simulink library "vehdynlibtire"  (R2019b)
settings: Solver=ode45  StartTime=0.0  StopTime=10.0  RelTol=1e-3  EnableMultiTasking=on
libraries: vehdynlibtirecommon x6, autolibshared x4, autolibsharedcommon x1
(part 1 of 3)
Description:
  | Vehicle Dynamics Blockset Library: Tire Dynamics
settings Model: ModifiedByFormat=The MathWorks, Inc.  Creator=The MathWorks, Inc.  LastModifiedBy=The MathWorks, Inc.
settings DataIOCC: LimitDataPoints=on  SaveFormat=Array  ReturnWorkspaceOutputs=off
settings OptimizationCC: LifeSpan=inf
settings DebuggingCC: AllowSymbolicDim=off  PregeneratedLibrarySubsystemCodeDiagnostic=none  SFUnexpectedBacktrackingDiag=warning  SFNoUnconditionalDefaultTransitionDiag=warning  SFExecutionAtInitializationDiag=none  ArithmeticOperatorsInVariantConditions=warning
settings HardwareCC: ProdBitPerPointer=32  ProdBitPerSizeT=32  ProdBitPerPtrDiffT=32  ProdLargestAtomicFloat=None  ProdIntDivRoundTo=Undefined  ProdEndianess=Unspecified  ProdWordSize=32  ProdHWDeviceType=32-bit Generic
settings ModelReferenceCC: PropagateSignalLabelsOutOfModel=off
settings SFSimCC: SimUseLocalCustomCode=off  CustomCodeUndefinedFunction=UseInterfaceOnly
settings RTWCC: RTWUseLocalCustomCode=off
settings CodeAppCC: StateflowObjectComments=on
settings GRTTargetCC: TargetLangStandard=C89/C90 (ANSI)  GeneratePreprocessorConditionals=Disable all
settings ConfigComp: CovMetricSettings=dw  CovHtmlReporting=on  CovSaveCumulativeToWorkspaceVar=on  CovSaveSingleToWorkspaceVar=on  CovShowResultsExplorer=off  CovExternalEMLEnable=off

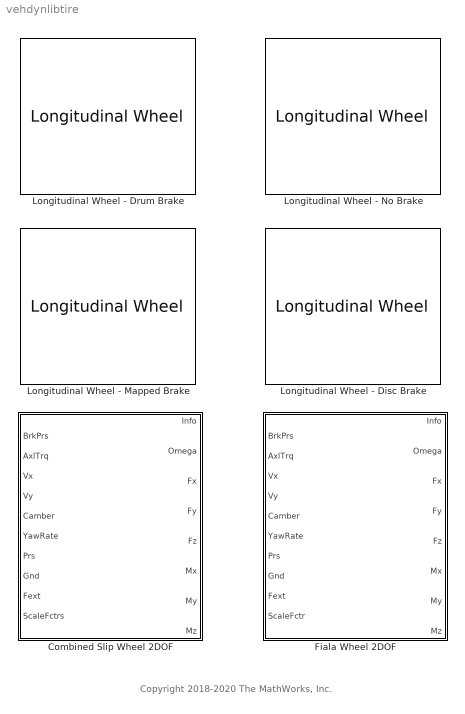
== system vehdynlibtire ==
  note: Copyright 2018-2020 The MathWorks, Inc.
  Combined Slip Wheel 2DOF : Subsystem  mask(Combined Slip Wheel 2DOF){BrakeType=Disc, mu_static=.3, mu_kinetic=.2, disk_abore=.05, Rm=.177, num_pads=2, drum_abore=0.0508, drum_a=0.123, drum_c=0.212, drum_r=0.15, drum_theta1=0, drum_theta2=126, brake_p_bpt=[1 11.4736842105263 21.9473684210526 32.4210526315789 42.8947368421053 53.3684210526316 63.8421052631579 74.3157894736842 84.7894736842105 95.2631578947368 105.736842105263 116.210526315789 126.684210526316 137.157894736842 147.631578947368 158.105263157895 168.578947368421 179.052631578947 189.526315789474 200], brake_n_bpt=[0 52.6315789473684 105.263157894737 157.894736842105 210.526315789474 263.157894736842 315.789473684211 368.421052631579 421.052631578947 473.684210526316 526.315789473684 578.947368421053 631.578947368421 684.210526315789 736.842105263158 789.473684210526 842.105263157895 894.736842105263 947.368421052632 1000], f_brake_t=[43.4900602404453 42.5056030554862 41.5350898940194 40.5780454442085 39.6340111501808 38.7025443887544 37.7832176914519 36.8756180088306 35.9793460143796 35.0940154454303 34.2192524787115 33.3546951383474 32.4999927342521 31.6548053290159 30.8188032315107 29.991666515561 29.1730845621415 28.362755623661 27.5603864089927 26.765691687993;498.991217495636 487.695866636631 476.560505099801 465.579679307235 454.748127933653 444.060772460445 433.51270824929 423.099196101319 412.81565427025 402.657650900201 392.620896861006 382.701238955775 372.894653477208 363.197240090814 353.605216024701 344.114910546964 334.722759712992 325.425301366216 316.219170376863 307.10109410434;954.492374750826 932.886130217776 911.585920305583 890.581313170261 869.862244717126 849.419000532136 829.242198807128 809.322774193808 789.651962526121 770.221286354971 751.0225412433 732.047782773203 713.289314220164 694.739674852612 676.391628817892 658.238154578366 640.272434863842 622.48784710877 604.877954344734 587.436496520688;1409.99353200602 1378.07639379892 1346.61133551136 1315.58294703329 1284.9763615006 1254.77722860383 1224.97168936497 1195.5463522863 1166.48827078199 1137.78492180974 1109.42418562559 1081.39432659063 1053.68397496312 1026.28210961441 999.178041611083 972.361398609768 945.822110014692 919.550392851325 893.536738312604 867.771898937035;1865.49468926121 1823.26665738007 1781.63675071715 1740.58458089631 1700.09047828407 1660.13545667552 1620.7011799228 1581.76993037878 1543.32457903786 1505.34855726451 1467.82583000789 1430.74087040806 1394.07863570608 1357.82454437621 1321.96445440427 1286.48464264117 1251.37178516554 1216.61293859388 1182.19552228048 1148.10730135338;2320.9958465164 2268.45692096121 2216.66216592293 2165.58621475934 2115.20459506754 2065.49368474721 2016.43067048064 1967.99350847127 1920.16088729373 1872.91219271928 1826.22747439018 1780.08741422549 1734.47329644903 1689.36697913801 1644.75086719747 1600.60788667257 1556.92146031639 1513.67548433643 1470.85430624835 1428.44270376973;2776.49700377159 2713.64718454235 2651.68758112871 2590.58784862237 2530.31871185102 2470.8519128189 2412.16016103848 2354.21708656376 2296.9971955496 2240.47582817405 2184.62911877248 2129.43395804292 2074.86795719199 2020.9094138998 1967.53727999066 1914.73113070398 1862.47113546724 1810.73803007899 1759.51309021622 1708.77810618608;3231.99816102678 3158.8374481235 3086.71299633449 3015.58948248539 2945.43282863449 2876.21014089059 2807.88965159632 2740.44066465625 2673.83350380547 2608.03946362882 2543.03076315477 2478.78050186034 2415.26261793494 2352.4518486616 2290.32369278385 2228.85437473538 2168.02081061809 2107.80057582154 2048.17187418409 1989.11350860242;3687.49931828197 3604.02771170464 3521.73841154027 3440.59111634842 3360.54694541796 3281.56836896228 3203.61914215416 3126.66424274874 3050.66981206134 2975.60309908359 2901.43240753707 2828.12704567777 2755.6572786779 2683.9942834234 2613.11010557704 2542.97761876678 2473.57048576894 2404.8631215641 2336.83065815196 2269.44891101877;4143.00047553716 4049.21797528579 3956.76382674606 3865.59275021144 3775.66106220143 3686.92659703397 3599.34863271199 3512.88782084123 3427.50612031721 3343.16673453836 3259.83405191936 3177.4735894952 3096.05193942085 3015.5367181852 2935.89651837023 2857.10086279818 2779.12016091979 2701.92566730665 2625.48944211983 2549.78431343512;4598.50163279235 4494.40823886693 4391.78924195184 4290.59438407447 4190.77517898491 4092.28482510566 3995.07812326983 3899.11139893372 3804.34242857308 3710.73036999313 3618.23569630166 3526.82013331263 3436.44660016381 3347.079152947 3258.68293116342 3171.22410682959 3084.66983607064 2998.98821304921 2914.1482260877 2830.11971585147;5054.00279004754 4939.59850244808 4826.81465715762 4715.59601793749 4605.88929576838 4497.64305317735 4390.80761382767 4285.3349770262 4181.17873682896 4078.2940054479 3976.63734068395 3876.16667713006 3776.84126090677 3678.62158770879 3581.46934395661 3485.34735086099 ...(+2764 chars)], tireParamSet=vdynPassCar.mat, plySteer=off, turnslip=off, PRESMAX=1003118, PRESMIN=9982, FZMAX=10000, FZMIN=100, VXLOW=0.1, KPUMAX=1.5, KPUMIN=-1.5, ALPMAX=1.5708, ALPMIN=-1.5708, CAMMAX=0.173142086627737, CAMMIN=-0.173348165334087, LONGVL=16.7, omegao=0, br=1e-3, UNLOADED_RADIUS=0.309, NOMPRES=224006, FNOMIN=4025, WIDTH=0.209, MASS=9.465, IYY=0.7406, GRAVITY=-9.81, zo=0, zdoto=0, BREFF=8.25094594147963, DREFF=0.260468730454265, FREFF=0.0735298544471851, Q_RE0=1.00866439868088, Q_V1=0.000760413786224011, Q_V2=0.0463384792019201, Q_FZ1=0, Q_FZ2=15.6870832810226, Q_FZ3=0, Q_FCX=0.138643970247602, Q_FCY=0.10843499565426, Q_FCY2=-0.465763352339538, PFZ1=0.69958166705601, VERTICAL_STIFFNESS=207885.061134007, VERTICAL_DAMPING=494.649255786991, LONGITUDINAL_STIFFNESS=388714.175879854, LATERAL_STIFFNESS=157087.404633332, PCFX1=0.18539229191199, PCFX2=0, PCFX3=0, PCFY1=0.163183345037677, PCFY2=0, PCFY3=0.249094918231954, Q_RA1=0.675942571700787, Q_RA2=0.73800463546164, Q_RB1=1.04487486456705, Q_RB2=-1.191763806629, PCX1=1.58523057950359, PDX1=1.0239116238178, PDX2=-0.0842405110022724, PDX3=0, PEX1=0.110312777158455, PEX2=0.313468516038146, PEX3=0, PEX4=0.0016060905760045, PKX1=21.3872544684023, PKX2=14.0006541873175, PKX3=-0.405326109653452, PHX1=0.000212599305364818, PHX2=0.00115950515263055, PVX1=1.59236164471432e-05, PVX2=0.000104321112127671, PPX1=-0.349461321276586, PPX2=0.387840040616429, PPX3=-0.0969947336569324, PPX4=0.0632271859795801, RBX1=12.7633329850276, RBX2=9.5787123658471, RBX3=0, RCX1=1.02796280922059, REX1=-0.45202516851367, REX2=-0.47304886171176, RHX1=0.000233272373115809, QSX1=-0.00788307788961443, QSX2=0.954629515459396, QSX3=0.0155855777667025, QSX4=0.125904607142414, QSX5=1.01110069703963, QSX6=20.1938577118433, QSX7=0.310818120717083, QSX8=-0.0430823751139655, QSX9=0.636494404888216, QSX10=0.142438060591663, QSX11=0.346766530036373, QSX12=0, QSX13=0, QSX14=0, PPMX1=0, PCY1=1.34299950037631, PDY1=0.878267729082195, PDY2=-0.0644597923147385, PDY3=0, PEY1=-0.809776534470972, PEY2=-0.600180598867198, PEY3=0.0991732552633487, PEY4=-6.5577974035573, PEY5=0, PKY1=-15.5714726518315, PKY2=1.73126522291751, PKY3=0.365349873517229, PKY4=1.98176755955416, PKY5=0, PKY6=-0.884005199550313, PKY7=-0.237259727611847, PHY1=-0.00183370557235628, PHY2=0.00346401302716671, PVY1=-0.00675427560163264, PVY2=0.036379218103843, PVY3=-0.163543984089166, PVY4=-0.491003349625726, PPY1=-0.62059646553185, PPY2=-0.0647824842338686, PPY3=-0.164648843290686, PPY4=0.283193909060098, PPY5=0, RBY1=10.7588809173639, RBY2=7.70420065295029, RBY3=3.40283755070691e-06, RBY4=0, RCY1=1.06691874059059, REY1=0.308244924574305, REY2=7.48775032604508e-06, RHY1=0.0118479204960415, RHY2=7.63650177161071e-06, RVY1=0.0560024425050078, RVY2=7.48487127056197e-06, RVY3=0, RVY4=98.4047026517149, RVY5=2.02759273900054, RVY6=15.7623064923347, QSY1=0.00699077564863536, QSY2=0, QSY3=0.00153535478298811, QSY4=8.55710322455322e-05, QSY5=0, QSY6=0, QSY7=0.89443879773793, QSY8=-0.403227641260894, QBZ1=11.666656027484, QBZ2=-1.30355438574485, QBZ3=0, QBZ4=0.177918305399071, QBZ5=-0.162481135068033, QBZ6=0, QBZ9=30.1445534682089, QBZ10=0, QCZ1=1.29026978207574, QDZ1=0.0886972644991399, QDZ2=-0.0058634820161856, QDZ3=0.3805597481383, QDZ4=0, QDZ6=0.00160914918118959, QDZ7=-0.00211036330862154, QDZ8=-0.13921904912557, QDZ9=0.00816585550028243, QDZ10=0, QDZ11=0, QEZ1=-2.19802254534746, QEZ2=1.01850535789165, QEZ3=0, QEZ4=0.278379679112054, QEZ5=-0.548414722765386, QHZ1=0.00148361198869669, QHZ2=0.00202017567585904, QHZ3=0.240316641332066, QHZ4=-0.210114035738085, PPZ1=-0.443927982388615, PPZ2=0, SSZ1=0.00914999585397887, SSZ2=0.0389830656052735, SSZ3=0, SSZ4=0, PDXP1=0.396718274678791, PDXP2=0, PDXP3=0, PKYP1=1.00587060633573, PDYP1=0.40483048923438, PDYP2=0, PDYP3=0, PDYP4=0, PHYP1=0.992731942067188, PHYP2=0.150352945499914, PHYP3=0, PHYP4=-3.98988682633674, PECP1=0.502379254513503, PECP2=0, QDTP1=10.0178654287947, QCRP1=0.200627747200702, QCRP2=0.0995735881599772, QBRP1=0.0997107127960717, QDRP1=1.01432910167423, QDRP2=0, aMode=2}
      mask prompts: BrakeType "vdynblks:vehdynLatTire:blkPrm_BrakeType"; mu_static "autoblks_shared:autoblkLongitudinalWheel:blkPrm_mu_static"; mu_kinetic "autoblks_shared:autoblkLongitudinalWheel:blkPrm_mu_kinetic"; disk_abore "autoblks_shared:autoblkLongitudinalWheel:blkPrm_disk_abore"; Rm "autoblks_shared:autoblkLongitudinalWheel:blkPrm_Rm"; num_pads "autoblks_shared:autoblkLongitudinalWheel:blkPrm_num_pads"; drum_abore "autoblks_shared:autoblkLongitudinalWheel:blkPrm_drum_abore"; drum_a "autoblks_shared:autoblkLongitudinalWheel:blkPrm_drum_a"; drum_c "autoblks_shared:autoblkLongitudinalWheel:blkPrm_drum_c"; drum_r "autoblks_shared:autoblkLongitudinalWheel:blkPrm_drum_r"; drum_theta1 "autoblks_shared:autoblkLongitudinalWheel:blkPrm_drum_theta1"; drum_theta2 "autoblks_shared:autoblkLongitudinalWheel:blkPrm_drum_theta2"; brake_p_bpt "autoblks_shared:autoblkLongitudinalWheel:blkPrm_brake_p_bpt"; brake_n_bpt "autoblks_shared:autoblkLongitudinalWheel:blkPrm_brake_n_bpt"; f_brake_t "autoblks_shared:autoblkLongitudinalWheel:blkPrm_f_brake_t"; tireParamSet "vdynblks:vehdynLatTire:blkPrm_tireParamSet"; plySteer "vdynblks:vehdynLatTire:blkPrm_plySteer"; turnslip "vdynblks:vehdynLatTire:blkPrm_turnslip"; PRESMAX "vdynblks:vehdynLatTire:blkPrm_PRESMAX"; PRESMIN "vdynblks:vehdynLatTire:blkPrm_PRESMIN"; FZMAX "vdynblks:vehdynLatTire:blkPrm_FZMAX"; FZMIN "vdynblks:vehdynLatTire:blkPrm_FZMIN"; VXLOW "vdynblks:vehdynLatTire:blkPrm_VXLOW"; KPUMAX "vdynblks:vehdynLatTire:blkPrm_KPUMAX"; KPUMIN "vdynblks:vehdynLatTire:blkPrm_KPUMIN"; ALPMAX "vdynblks:vehdynLatTire:blkPrm_ALPMAX"; ALPMIN "vdynblks:vehdynLatTire:blkPrm_ALPMIN"; CAMMAX "vdynblks:vehdynLatTire:blkPrm_CAMMAX"; CAMMIN "vdynblks:vehdynLatTire:blkPrm_CAMMIN"; LONGVL "vdynblks:vehdynLatTire:blkPrm_LONGVL"; omegao "vdynblks:vehdynLatTire:blkPrm_omegao"; br "vdynblks:vehdynLatTire:blkPrm_br"; UNLOADED_RADIUS "vdynblks:vehdynLatTire:blkPrm_UNLOADED_RADIUS"; NOMPRES "vdynblks:vehdynLatTire:blkPrm_NOMPRES"; FNOMIN "vdynblks:vehdynLatTire:blkPrm_FNOMIN"; WIDTH "vdynblks:vehdynLatTire:blkPrm_WIDTH"; MASS "vdynblks:vehdynLatTire:blkPrm_MASS"; IYY "vdynblks:vehdynLatTire:blkPrm_IYY"; GRAVITY "vdynblks:vehdynLatTire:blkPrm_GRAVITY"; zo "vdynblks:vehdynLatTire:blkPrm_zo"; zdoto "vdynblks:vehdynLatTire:blkPrm_zdoto"; BREFF "vdynblks:vehdynLatTire:blkPrm_BREFF"; DREFF "vdynblks:vehdynLatTire:blkPrm_DREFF"; FREFF "vdynblks:vehdynLatTire:blkPrm_FREFF"; Q_RE0 "vdynblks:vehdynLatTire:blkPrm_Q_RE0"; Q_V1 "vdynblks:vehdynLatTire:blkPrm_Q_V1"; Q_V2 "vdynblks:vehdynLatTire:blkPrm_Q_V2"; Q_FZ1 "vdynblks:vehdynLatTire:blkPrm_Q_FZ1"; Q_FZ2 "vdynblks:vehdynLatTire:blkPrm_Q_FZ2"; Q_FZ3 "vdynblks:vehdynLatTire:blkPrm_Q_FZ3"; Q_FCX "vdynblks:vehdynLatTire:blkPrm_Q_FCX"; Q_FCY "vdynblks:vehdynLatTire:blkPrm_Q_FCY"; Q_FCY2 "vdynblks:vehdynLatTire:blkPrm_Q_FCY2"; PFZ1 "vdynblks:vehdynLatTire:blkPrm_PFZ1"; VERTICAL_STIFFNESS "vdynblks:vehdynLatTire:blkPrm_VERTICAL_STIFFNESS"; VERTICAL_DAMPING "vdynblks:vehdynLatTire:blkPrm_VERTICAL_DAMPING"; LONGITUDINAL_STIFFNESS "vdynblks:vehdynLatTire:blkPrm_LONGITUDINAL_STIFFNESS"; LATERAL_STIFFNESS "vdynblks:vehdynLatTire:blkPrm_LATERAL_STIFFNESS"; PCFX1 "vdynblks:vehdynLatTire:blkPrm_PCFX1"; PCFX2 "vdynblks:vehdynLatTire:blkPrm_PCFX2"; PCFX3 "vdynblks:vehdynLatTire:blkPrm_PCFX3"; PCFY1 "vdynblks:vehdynLatTire:blkPrm_PCFY1"; PCFY2 "vdynblks:vehdynLatTire:blkPrm_PCFY2"; PCFY3 "vdynblks:vehdynLatTire:blkPrm_PCFY3"; Q_RA1 "vdynblks:vehdynLatTire:blkPrm_Q_RA1"; Q_RA2 "vdynblks:vehdynLatTire:blkPrm_Q_RA2"; Q_RB1 "vdynblks:vehdynLatTire:blkPrm_Q_RB1"; Q_RB2 "vdynblks:vehdynLatTire:blkPrm_Q_RB2"; PCX1 "vdynblks:vehdynLatTire:blkPrm_PCX1"; PDX1 "vdynblks:vehdynLatTire:blkPrm_PDX1"; PDX2 "vdynblks:vehdynLatTire:blkPrm_PDX2"; PDX3 "vdynblks:vehdynLatTire:blkPrm_PDX3"; PEX1 "vdynblks:vehdynLatTire:blkPrm_PEX1"; PEX2 "vdynblks:vehdynLatTire:blkPrm_PEX2"; PEX3 "vdynblks:vehdynLatTire:blkPrm_PEX3"; PEX4 "vdynblks:vehdynLatTire:blkPrm_PEX4"; PKX1 "vdynblks:vehdynLatTire:blkPrm_PKX1"; PKX2 "vdynblks:vehdynLatTire:blkPrm_PKX2"; PKX3 "vdynblks:vehdynLatTire:blkPrm_PKX3"; PHX1 "vdynblks:vehdynLatTire:blkPrm_PHX1"; PHX2 "vdynblks:vehdynLatTire:blkPrm_PHX2"; PVX1 "vdynblks:vehdynLatTire:blkPrm_PVX1"; PVX2 "vdynblks:vehdynLatTire:blkPrm_PVX2"; PPX1 "vdynblks:vehdynLatTire:blkPrm_PPX1"; PPX2 "vdynblks:vehdynLatTire:blkPrm_PPX2"; PPX3 "vdynblks:vehdynLatTire:blkPrm_PPX3"; PPX4 "vdynblks:vehdynLatTire:blkPrm_PPX4"; RBX1 "vdynblks:vehdynLatTire:blkPrm_RBX1"; RBX2 "vdynblks:vehdynLatTire:blkPrm_RBX2"; RBX3 "vdynblks:vehdynLatTire:blkPrm_RBX3"; RCX1 "vdynblks:vehdynLatTire:blkPrm_RCX1"; REX1 "vdynblks:vehdynLatTire:blkPrm_REX1"; REX2 "vdynblks:vehdynLatTire:blkPrm_REX2"; RHX1 "vdynblks:vehdynLatTire:blkPrm_RHX1"; QSX1 "vdynblks:vehdynLatTire:blkPrm_QSX1"; QSX2 "vdynblks:vehdynLatTire:blkPrm_QSX2"; QSX3 "vdynblks:vehdynLatTire:blkPrm_QSX3"; QSX4 "vdynblks:vehdynLatTire:blkPrm_QSX4"; QSX5 "vdynblks:vehdynLatTire:blkPrm_QSX5"; QSX6 "vdynblks:vehdynLatTire:blkPrm_QSX6"; QSX7 "vdynblks:vehdynLatTire:blkPrm_QSX7"; QSX8 "vdynblks:vehdynLatTire:blkPrm_QSX8"; QSX9 "vdynblks:vehdynLatTire:blkPrm_QSX9"; QSX10 "vdynblks:vehdynLatTire:blkPrm_QSX10"; QSX11 "vdynblks:vehdynLatTire:blkPrm_QSX11"; QSX12 "vdynblks:vehdynLatTire:blkPrm_QSX12"; QSX13 "vdynblks:vehdynLatTire:blkPrm_QSX13"; QSX14 "vdynblks:vehdynLatTire:blkPrm_QSX14"; PPMX1 "vdynblks:vehdynLatTire:blkPrm_PPMX1"; PCY1 "vdynblks:vehdynLatTire:blkPrm_PCY1"; PDY1 "vdynblks:vehdynLatTire:blkPrm_PDY1"; PDY2 "vdynblks:vehdynLatTire:blkPrm_PDY2"; PDY3 "vdynblks:vehdynLatTire:blkPrm_PDY3"; PEY1 "vdynblks:vehdynLatTire:blkPrm_PEY1"; PEY2 "vdynblks:vehdynLatTire:blkPrm_PEY2"; PEY3 "vdynblks:vehdynLatTire:blkPrm_PEY3"; PEY4 "vdynblks:vehdynLatTire:blkPrm_PEY4"; PEY5 "vdynblks:vehdynLatTire:blkPrm_PEY5"; PKY1 "vdynblks:vehdynLatTire:blkPrm_PKY1"; PKY2 "vdynblks:vehdynLatTire:blkPrm_PKY2"; PKY3 "vdynblks:vehdynLatTire:blkPrm_PKY3"; PKY4 "vdynblks:vehdynLatTire:blkPrm_PKY4"; PKY5 "vdynblks:vehdynLatTire:blkPrm_PKY5"; PKY6 "vdynblks:vehdynLatTire:blkPrm_PKY6"; PKY7 "vdynblks:vehdynLatTire:blkPrm_PKY7"; PHY1 "vdynblks:vehdynLatTire:blkPrm_PHY1"; PHY2 "vdynblks:vehdynLatTire:blkPrm_PHY2"; PVY1 "vdynblks:vehdynLatTire:blkPrm_PVY1"; PVY2 "vdynblks:vehdynLatTire:blkPrm_PVY2"; PVY3 "vdynblks:vehdynLatTire:blkPrm_PVY3"; PVY4 "vdynblks:vehdynLatTire:blkPrm_PVY4"; PPY1 "vdynblks:vehdynLatTire:blkPrm_PPY1"; PPY2 "vdynblks:vehdynLatTire:blkPrm_PPY2"; PPY3 "vdynblks:vehdynLatTire:blkPrm_PPY3"; PPY4 "vdynblks:vehdynLatTire:blkPrm_PPY4"; PPY5 "vdynblks:vehdynLatTire:blkPrm_PPY5"; RBY1 "vdynblks:vehdynLatTire:blkPrm_RBY1"; RBY2 "vdynblks:vehdynLatTire:blkPrm_RBY2"; RBY3 "vdynblks:vehdynLatTire:blkPrm_RBY3"; RBY4 "vdynblks:vehdynLatTire:blkPrm_RBY4"; RCY1 "vdynblks:vehdynLatTire:blkPrm_RCY1"; REY1 "vdynblks:vehdynLatTire:blkPrm_REY1"; REY2 "vdynblks:vehdynLatTire:blkPrm_REY2"; RHY1 "vdynblks:vehdynLatTire:blkPrm_RHY1"; RHY2 "vdynblks:vehdynLatTire:blkPrm_RHY2"; RVY1 "vdynblks:vehdynLatTire:blkPrm_RVY1"; RVY2 "vdynblks:vehdynLatTire:blkPrm_RVY2"; RVY3 "vdynblks:vehdynLatTire:blkPrm_RVY3"; RVY4 "vdynblks:vehdynLatTire:blkPrm_RVY4"; RVY5 "vdynblks:vehdynLatTire:blkPrm_RVY5"; RVY6 "vdynblks:vehdynLatTire:blkPrm_RVY6"; QSY1 "vdynblks:vehdynLatTire:blkPrm_QSY1"; QSY2 "vdynblks:vehdynLatTire:blkPrm_QSY2"; QSY3 "vdynblks:vehdynLatTire:blkPrm_QSY3"; QSY4 "vdynblks:vehdynLatTire:blkPrm_QSY4"; QSY5 "vdynblks:vehdynLatTire:blkPrm_QSY5"; QSY6 "vdynblks:vehdynLatTire:blkPrm_QSY6"; QSY7 "vdynblks:vehdynLatTire:blkPrm_QSY7"; QSY8 "vdynblks:vehdynLatTire:blkPrm_QSY8"; QBZ1 "vdynblks:vehdynLatTire:blkPrm_QBZ1"; QBZ2 "vdynblks:vehdynLatTire:blkPrm_QBZ2"; QBZ3 "vdynblks:vehdynLatTire:blkPrm_QBZ3"; QBZ4 "vdynblks:vehdynLatTire:blkPrm_QBZ4"; QBZ5 "vdynblks:vehdynLatTire:blkPrm_QBZ5"; QBZ6 "vdynblks:vehdynLatTire:blkPrm_QBZ6"; QBZ9 "vdynblks:vehdynLatTire:blkPrm_QBZ9"; QBZ10 "vdynblks:vehdynLatTire:blkPrm_QBZ10"; QCZ1 "vdynblks:vehdynLatTire:blkPrm_QCZ1"; QDZ1 "vdynblks:vehdynLatTire:blkPrm_QDZ1"; QDZ2 "vdynblks:vehdynLatTire:blkPrm_QDZ2"; QDZ3 "vdynblks:vehdynLatTire:blkPrm_QDZ3"; QDZ4 "vdynblks:vehdynLatTire:blkPrm_QDZ4"; QDZ6 "vdynblks:vehdynLatTire:blkPrm_QDZ6"; QDZ7 "vdynblks:vehdynLatTire:blkPrm_QDZ7"; QDZ8 "vdynblks:vehdynLatTire:blkPrm_QDZ8"; QDZ9 "vdynblks:vehdynLatTire:blkPrm_QDZ9"; QDZ10 "vdynblks:vehdynLatTire:blkPrm_QDZ10"; QDZ11 "vdynblks:vehdynLatTire:blkPrm_QDZ11"; QEZ1 "vdynblks:vehdynLatTire:blkPrm_QEZ1"; QEZ2 "vdynblks:vehdynLatTire:blkPrm_QEZ2"; QEZ3 "vdynblks:vehdynLatTire:blkPrm_QEZ3"; QEZ4 "vdynblks:vehdynLatTire:blkPrm_QEZ4"; QEZ5 "vdynblks:vehdynLatTire:blkPrm_QEZ5"; QHZ1 "vdynblks:vehdynLatTire:blkPrm_QHZ1"; QHZ2 "vdynblks:vehdynLatTire:blkPrm_QHZ2"; QHZ3 "vdynblks:vehdynLatTire:blkPrm_QHZ3"; QHZ4 "vdynblks:vehdynLatTire:blkPrm_QHZ4"; PPZ1 "vdynblks:vehdynLatTire:blkPrm_PPZ1"; PPZ2 "vdynblks:vehdynLatTire:blkPrm_PPZ2"; SSZ1 "vdynblks:vehdynLatTire:blkPrm_SSZ1"; SSZ2 "vdynblks:vehdynLatTire:blkPrm_SSZ2"; SSZ3 "vdynblks:vehdynLatTire:blkPrm_SSZ3"; SSZ4 "vdynblks:vehdynLatTire:blkPrm_SSZ4"; PDXP1 "vdynblks:vehdynLatTire:blkPrm_PDXP1"; PDXP2 "vdynblks:vehdynLatTire:blkPrm_PDXP2"; PDXP3 "vdynblks:vehdynLatTire:blkPrm_PDXP3"; PKYP1 "vdynblks:vehdynLatTire:blkPrm_PKYP1"; PDYP1 "vdynblks:vehdynLatTire:blkPrm_PDYP1"; PDYP2 "vdynblks:vehdynLatTire:blkPrm_PDYP2"; PDYP3 "vdynblks:vehdynLatTire:blkPrm_PDYP3"; PDYP4 "vdynblks:vehdynLatTire:blkPrm_PDYP4"; PHYP1 "vdynblks:vehdynLatTire:blkPrm_PHYP1"; PHYP2 "vdynblks:vehdynLatTire:blkPrm_PHYP2"; PHYP3 "vdynblks:vehdynLatTire:blkPrm_PHYP3"; PHYP4 "vdynblks:vehdynLatTire:blkPrm_PHYP4"; PECP1 "vdynblks:vehdynLatTire:blkPrm_PECP1"; PECP2 "vdynblks:vehdynLatTire:blkPrm_PECP2"; QDTP1 "vdynblks:vehdynLatTire:blkPrm_QDTP1"; QCRP1 "vdynblks:vehdynLatTire:blkPrm_QCRP1"; QCRP2 "vdynblks:vehdynLatTire:blkPrm_QCRP2"; QBRP1 "vdynblks:vehdynLatTire:blkPrm_QBRP1"; QDRP1 "vdynblks:vehdynLatTire:blkPrm_QDRP1"; QDRP2 "vdynblks:vehdynLatTire:blkPrm_QDRP2"
      mask help: vdynblks:vehdynLatTire:blkDesc
      mask init:
      | [~]=vehdynicon('vehdynlibtire',gcb,0)
      mask Help: eval('vdynblkshelp(''vbtireslip'')')
      mask TypeOptions BrakeType: autoblks_shared:autoblkLongitudinalWheel:blkCmb_BrakeType_c1 | autoblks_shared:autoblkLongitudinalWheel:blkCmb_BrakeType_c2 | autoblks_shared:autoblkLongitudinalWheel:blkCmb_BrakeType_c3 | autoblks_shared:autoblkLongitudinalWheel:blkCmb_BrakeType_c4
      mask Callback BrakeType: [~]=vehdynicon('vehdynlibtire',gcb,2)
      mask DialogControl BlockOptions Prompt: autoblks_shared:autoblkLongitudinalWheel:blkDlg_BlockOptions
      mask DialogControl BrakeType Prompt: Brake Type:
      mask DialogControl WheelParams Prompt: Wheel and Tire Parameters
      mask DialogControl brakeParamPanel Prompt: autoblks_shared:autoblkLongitudinalWheel:blkDlg_brakeParamPanel
      mask DialogControl GenParams Prompt: autoblks_shared:autoblkLongitudinalWheel:blkDlg_GenParams
      mask DialogControl mu_static Prompt: Static friction coefficient, mu_static []:
      mask DialogControl mu_kinetic Prompt: Kinetic friction coefficient, mu_kinetic []:
      mask DialogControl DiskBrakeParms Prompt: autoblks_shared:autoblkLongitudinalWheel:blkDlg_DiskBrakeParms
      mask DialogControl disk_abore Prompt: Disc brake actuator bore, disk_abore [m]:
      mask DialogControl Rm Prompt: Brake pad mean radius, Rm [m]:
      mask DialogControl num_pads Prompt: Number of brake pads, num_pads []:
      mask DialogControl DrumBrakeParms Prompt: autoblks_shared:autoblkLongitudinalWheel:blkDlg_DrumBrakeParms
      mask DialogControl drum_abore Prompt: Drum brake actuator bore, drum_abore [m]:
      mask DialogControl drum_a Prompt: Shoe pin to drum center distance, drum_a [m]:
      mask DialogControl drum_c Prompt: Shoe pin center to force application point distance, drum_c [m]:
      mask DialogControl drum_r Prompt: Drum internal radius, drum_r [m]:
      mask DialogControl drum_theta1 Prompt: Shoe pin to pad start angle, drum_theta1 [deg]:
      mask DialogControl drum_theta2 Prompt: Shoe pin to pad end angle, drum_theta2 [deg]:
      mask DialogControl MappedBrakeParms Prompt: autoblks_shared:autoblkLongitudinalWheel:blkDlg_MappedBrakeParms
      mask DialogControl brake_p_bpt Prompt: Brake actuator pressure breakpoints, brake_p_bpt [bar]:
      mask DialogControl brake_n_bpt Prompt: Wheel speed breakpoints, brake_n_bpt [rpm]:
      mask DialogControl f_brake_t Prompt: Brake torque map, f_brake_t [Nm]:
      mask DialogControl PlotBrakeTorqueMap Prompt: autoblks_shared:autoblkLongitudinalWheel:blkDlg_PlotBrakeTorqueMap
      mask DialogControl PlotBrakeTorqueMap Callback: [~]=vehdynicon('vehdynlibtire',gcb,3)
      mask DialogControl tireDataPanel Prompt: Tire
      mask DialogControl tireParamSet Prompt: Tire file or object, tireParamSet []:
      mask DialogControl plySteer Prompt: Include ply/roll steer behavior
      mask DialogControl turnslip Prompt: Include large turn slip effects
      mask DialogControl getFile Prompt: Select file
      mask DialogControl getFile Callback: [~]=vehdynicon('vehdynlibtire',gcb,4)
      mask DialogControl updateMaskVars Prompt: Update mask values from file
      mask DialogControl updateMaskVars Callback: [~]=vehdynicon('vehdynlibtire',gcb,1)
      mask DialogControl tireParamTab Prompt: Tire Parameters
      mask DialogControl simParamPannel Prompt: Simulation
      mask DialogControl PRESMAX Prompt: Maximum pressure, PRESMAX [Pa]:
      mask DialogControl PRESMIN Prompt: Minimum pressure, PRESMIN [Pa]:
      mask DialogControl FZMAX Prompt: Maximum normal force, FZMAX [N]:
      mask DialogControl FZMIN Prompt: Minimum normal force, FZMIN [N]:
      mask DialogControl VXLOW Prompt: Velocity tolerance used to handle low velocity situations, VXLOW [m/s]:
      mask DialogControl KPUMAX Prompt: Max allowable slip ratio (absolute), KPUMAX []:
      mask DialogControl KPUMIN Prompt: Minimum allowable slip ratio (absolute), KPUMIN []:
      mask DialogControl ALPMAX Prompt: Max allowable slip angle (absolute), ALPMAX [rad]:
      mask DialogControl ALPMIN Prompt: Minimum allowable slip angle (absolute), ALPMIN [rad]:
      mask DialogControl CAMMAX Prompt: Maximum allowable camber angle, CAMMAX [rad]:
      mask DialogControl CAMMIN Prompt: Minimum allowable camber angle, CAMMIN [rad]:
      mask DialogControl LONGVL Prompt: Nominal longitudinal speed, LONGVL [m/s]:
      mask DialogControl wheelParamPannel Prompt: Wheel
      mask DialogControl omegao Prompt: Initial rotational velocity, omegao [rad/s]:
      mask DialogControl br Prompt: Rotational damping, br [N*m*s/rad]:
      mask DialogControl UNLOADED_RADIUS Prompt: Unloaded radius, UNLOADED_RADIUS [m]:
      mask DialogControl NOMPRES Prompt: Nominal pressure, NOMPRES [Pa]:
      mask DialogControl FNOMIN Prompt: Nominal normal force, FNOMIN [N]:
      mask DialogControl WIDTH Prompt: Wheel width, WIDTH [m]:
      mask DialogControl inertParamPannel Prompt: Inertial
      mask DialogControl MASS Prompt: Wheel mass, MASS [kg]:
      mask DialogControl IYY Prompt: Rotational inertia (rolling axis), IYY [kg*m^2]:
      mask DialogControl GRAVITY Prompt: Gravity, GRAVITY [m/s^2]:
      mask DialogControl vertParamPannel Prompt: Vertical
      mask DialogControl zo Prompt: Initial tire deflection, zo [m]:
      mask DialogControl zdoto Prompt: Initial wheel vertical velocity (wheel fixed frame), zdoto [m/s]:
      mask DialogControl BREFF Prompt: Effective rolling radius at low load stiffness, BREFF []:
      mask DialogControl DREFF Prompt: Effective rolling radius peak value, DREFF []:
      mask DialogControl FREFF Prompt: Effective rolling radius at high load stiffness, FREFF []:
      mask DialogControl Q_RE0 Prompt: Unloaded to nominal rolling radius ratio, Q_RE0 []:
      mask DialogControl Q_V1 Prompt: Radius rotational speed dependence, Q_V1 []:
      mask DialogControl Q_V2 Prompt: Stiffness rotational speed dependence, Q_V2 []:
      mask DialogControl Q_FZ1 Prompt: Linear load change with deflection, Q_FZ1 []:
      mask DialogControl Q_FZ2 Prompt: Quadratic load change with deflection, Q_FZ2 []:
      mask DialogControl Q_FZ3 Prompt: Linear load change with deflection and quadratic camber, Q_FZ3 []:
      mask DialogControl Q_FCX Prompt: Load response to longitudinal force, Q_FCX []:
      mask DialogControl Q_FCY Prompt: Load response to lateral force, Q_FCY []:
      mask DialogControl Q_FCY2 Prompt: Vertical stiffness change due to lateral load dependency on lateral stiffness, Q_FCY2 []:
      mask DialogControl PFZ1 Prompt: Stiffness response to pressure, PFZ1 []:
      mask DialogControl VERTICAL_STIFFNESS Prompt: Vertical tire stiffness, VERTICAL_STIFFNESS [N/m]:
      mask DialogControl VERTICAL_DAMPING Prompt: Vertical tire damping, VERTICAL_DAMPING [N*s/m]:
      mask DialogControl structParamPannel Prompt: Structural
      mask DialogControl LONGITUDINAL_STIFFNESS Prompt: Longitudinal stiffness, LONGITUDINAL_STIFFNESS [N/m]:
      mask DialogControl LATERAL_STIFFNESS Prompt: Lateral stiffness, LATERAL_STIFFNESS [N/m]:
      mask DialogControl PCFX1 Prompt: Linear vertical deflection influence on longitudinal stiffness, PCFX1 []:
      mask DialogControl PCFX2 Prompt: Quadratic vertical deflection influence on longitudinal stiffness, PCFX2 []:
      mask DialogControl PCFX3 Prompt: Pressure dependency on longitudinal stiffness, PCFX3 []:
      mask DialogControl PCFY1 Prompt: Linear vertical deflection influence on lateral stiffness, PCFY1 []:
      mask DialogControl PCFY2 Prompt: Quadratic vertical deflection influence on lateral stiffness, PCFY2 []:
      mask DialogControl PCFY3 Prompt: Pressure dependency on longitudinal stiffness, PCFY3 []:
      mask DialogControl contParamPannel Prompt: Contact Patch
      mask DialogControl Q_RA1 Prompt: Contact length square root term, Q_RA1 []:
      mask DialogControl Q_RA2 Prompt: Contact length linear term, Q_RA2 []:
      mask DialogControl Q_RB1 Prompt: Contact width root term, Q_RB1 []:
      mask DialogControl Q_RB2 Prompt: Contact width linear term, Q_RB2 []:
      mask DialogControl longParamPannel Prompt: Longitudinal
      mask DialogControl PCX1 Prompt: Cfx shape factor, PCX1 []:
      mask DialogControl PDX1 Prompt: Longitudinal friction at nominal normal load, PDX1 []:
      mask DialogControl PDX2 Prompt: Frictional variation with load, PDX2 []:
      mask DialogControl PDX3 Prompt: Frictional variation with camber, PDX3 [1/rad^2]:
      mask DialogControl PEX1 Prompt: Longitudinal curvature at nominal normal load, PEX1 []:
      mask DialogControl PEX2 Prompt: Variation of curvature factor with load, PEX2 []:
      mask DialogControl PEX3 Prompt: Variation of curvature factor with square of load, PEX3 []:
      mask DialogControl PEX4 Prompt: Longitudinal curvature factor with slip, PEX4 []:
      mask DialogControl PKX1 Prompt: Longitudinal slip stiffness at nominal normal load, PKX1 []:
      mask DialogControl PKX2 Prompt: Variation of slip stiffness with load, PKX2 []:
      mask DialogControl PKX3 Prompt: Slip stiffness exponent factor, PKX3 []:
      mask DialogControl PHX1 Prompt: Horizontal shift in slip ratio at nominal normal load, PHX1 []:
      mask DialogControl PHX2 Prompt: Variation of horizontal slip ratio with load, PHX2 []:
      mask DialogControl PVX1 Prompt: Vertical shift in load at nominal normal load, PVX1 []:
      mask DialogControl PVX2 Prompt: Variation of vertical shift with load, PVX2 []:
      mask DialogControl PPX1 Prompt: Linear variation of longitudinal slip stiffness with tire pressure, PPX1 []:
      mask DialogControl PPX2 Prompt: Quadratic variation of longitudinal slip stiffness with tire pressure, PPX2 []:
      mask DialogControl PPX3 Prompt: Linear variation of peak longitudinal friction with tire pressure, PPX3 []:
      mask DialogControl PPX4 Prompt: Quadratic variation of peak longitudinal friction with tire pressure, PPX4 []:
      mask DialogControl RBX1 Prompt: Combined slip Fx slope factor reduction, RBX1 []:
      mask DialogControl RBX2 Prompt: Slip ratio Fx slope reduction variation, RBX2 []:
      mask DialogControl RBX3 Prompt: Camber influence on combined slip Fx stiffness, RBX3 []:
      mask DialogControl RCX1 Prompt: Shape factor for combined slip Fx reduction, RCX1 []:
      mask DialogControl REX1 Prompt: Combined Fx curvature factor, REX1 []:
      mask DialogControl REX2 Prompt: Combined Fx curvature factor with load, REX2 []:
      mask DialogControl RHX1 Prompt: Combined slip Fx shift factor reduction, RHX1 []:
      mask DialogControl overParamPannel Prompt: Overturning
      mask DialogControl QSX1 Prompt: Vertical shift of overturning moment, QSX1 []:
      mask DialogControl QSX2 Prompt: Overturning moment due to camber, QSX2 []:
      mask DialogControl QSX3 Prompt: Overturning moment due to Fy, QSX3 []:
      mask DialogControl QSX4 Prompt: Mx combined lateral force load and camber, QSX4 []:
      mask DialogControl QSX5 Prompt: Mx load effect due to lateral force and camber, QSX5 []:
      mask DialogControl QSX6 Prompt: Mx load effect due to B-factor, QSX6 []:
      mask DialogControl QSX7 Prompt: Mx due to camber and load, QSX7 []:
      mask DialogControl QSX8 Prompt: Mx due to lateral force and load, QSX8 []:
      mask DialogControl QSX9 Prompt: Mx due to B-factor of lateral force and load, QSX9 []:
      mask DialogControl QSX10 Prompt: Mx due to vertical force and camber, QSX10 []:
      mask DialogControl QSX11 Prompt: Mx due to B-factor of vertical force and camber, QSX11 []:
      mask DialogControl QSX12 Prompt: Mx due to squared camber, QSX12 []:
      mask DialogControl QSX13 Prompt: Mx due to lateral force, QSX13 []:
      mask DialogControl QSX14 Prompt: Mx due to lateral force with camber, QSX14 []:
      mask DialogControl PPMX1 Prompt: Mx due to inflation pressure, PPMX1 []:
      mask DialogControl lateralParamPanel Prompt: Lateral
      mask DialogControl PCY1 Prompt: Cfy shape factor for lateral force, PCY1 []:
      mask DialogControl PDY1 Prompt: Lateral friction muy, PDY1 []:
      mask DialogControl PDY2 Prompt: Lateral friction variation of muy with load, PDY2 []:
      mask DialogControl PDY3 Prompt: Lateral friction variation of muy with squared camber, PDY3 []:
      mask DialogControl PEY1 Prompt: Efy lateral curvature at nominal force FZNOM, PEY1 []:
      mask DialogControl PEY2 Prompt: Efy curvature variation with load PEY2, PEY2 []:
      mask DialogControl PEY3 Prompt: Efy curvature constant camber dependency, PEY3 []:
      mask DialogControl PEY4 Prompt: Efy curvature variation with camber, PEY4 []:
      mask DialogControl PEY5 Prompt: Efy curvature variation with camber squared, PEY5 []:
      mask DialogControl PKY1 Prompt: Maximum KFy/FZNOM stiffness, PKY1 []:
      mask DialogControl PKY2 Prompt: Load at maximum KFy/FZNOM stiffness, PKY2 []:
      mask DialogControl PKY3 Prompt: KFy/FZNOM stiffness variation with camber, PKY3 []:
      mask DialogControl PKY4 Prompt: KFy curvature, PKY4 []:
      mask DialogControl PKY5 Prompt: Variation of peak stiffness with squared camber, PKY5 []:
      mask DialogControl PKY6 Prompt: Fy camber stiffness factor, PKY6 []:
      mask DialogControl PKY7 Prompt: Camber stiffness vertical load dependency, PKY7 []:
      mask DialogControl PHY1 Prompt: SHY horizontal shift at FZNOM, PHY1 []:
      mask DialogControl PHY2 Prompt: SHY variation with load, PHY2 []:
      mask DialogControl PVY1 Prompt: Svy/Fz vertical shift at FZNOM, PVY1 []:
      mask DialogControl PVY2 Prompt: Svy/Fz variation with load, PVY2 []:
      mask DialogControl PVY3 Prompt: Svy/Fz variation with camber, PVY3 []:
      mask DialogControl PVY4 Prompt: Svy/Fz variation with load and camber, PVY4 []:
      mask DialogControl PPY1 Prompt: Cornering stiffness variation with inflation pressure, PPY1 []:
      mask DialogControl PPY2 Prompt: Cornering stiffness variation with inflation pressure induced nominal load dependency, PPY2 []:
      mask DialogControl PPY3 Prompt: Linear inflation pressure on peak lateral friction, PPY3 []:
      mask DialogControl PPY4 Prompt: Quadratic inflation pressure on peak lateral friction, PPY4 []:
      mask DialogControl PPY5 Prompt: Inflation pressure effect on camber stiffness, PPY5 []:
      mask DialogControl RBY1 Prompt: Combined Fy reduction slope factor, RBY1 []:
      mask DialogControl RBY2 Prompt: Fy slope reduction with slip angle, RBY2 []:
      mask DialogControl RBY3 Prompt: Fy shift reduction with slip angle, RBY3 []:
      mask DialogControl RBY4 Prompt: Fy combined stiffness variation from camber, RBY4 []:
      mask DialogControl RCY1 Prompt: Fy combined reduction shape factor, RCY1 []:
      mask DialogControl REY1 Prompt: Fy combined curvature factor, REY1 []:
      mask DialogControl REY2 Prompt: Fy combined curvature factor with load, REY2 []:
      mask DialogControl RHY1 Prompt: Fy combined reduction shift factor, RHY1 []:
      mask DialogControl RHY2 Prompt: Fy combined reduction shift factor with load, RHY2 []:
      mask DialogControl RVY1 Prompt: Slip ratio side force Svyk/Muy*Fz at FZNOM, RVY1 []:
      mask DialogControl RVY2 Prompt: Side force Svyk/Muy*Fz variation with load, RVY2 []:
      mask DialogControl RVY3 Prompt: Side force Svyk/Muy*Fz variation with camber, RVY3 []:
      mask DialogControl RVY4 Prompt: Side force Svyk/Muy*Fz variation with slip angle, RVY4 []:
      mask DialogControl RVY5 Prompt: Side force Svyk/Muy*Fz variation with slip ratio, RVY5 []:
      mask DialogControl RVY6 Prompt: Side force Svyk/Muy*Fz variation with slip ratio arctangent, RVY6 []:
      mask DialogControl rollParamPanel Prompt: Rolling
      mask DialogControl QSY1 Prompt: Torque resistance coefficient, QSY1 []:
      mask DialogControl QSY2 Prompt: Torque resistance due to Fx, QSY2 []:
      mask DialogControl QSY3 Prompt: Torque resistance due to speed, QSY3 []:
      mask DialogControl QSY4 Prompt: Torque resistance due to speed^4, QSY4 []:
      mask DialogControl QSY5 Prompt: Torque resistance due to square of camber, QSY5 []:
      mask DialogControl QSY6 Prompt: Torque resistance due to square of camber and load, QSY6 []:
      mask DialogControl QSY7 Prompt: Torque resistance due to load, QSY7 []:
      mask DialogControl QSY8 Prompt: Torque resistance due to pressure, QSY8 []:
      mask DialogControl alignParamPanel Prompt: Aligning
      mask DialogControl QBZ1 Prompt: Trail slope factor for trail Bpt at FZNOM, QBZ1 []:
      mask DialogControl QBZ2 Prompt: Bpt slope variation with load, QBZ2 []:
      mask DialogControl QBZ3 Prompt: Bpt slope variation with square of load, QBZ3 []:
      mask DialogControl QBZ4 Prompt: Bpt slope variation with camber, QBZ4 []:
      mask DialogControl QBZ5 Prompt: Bpt slope variation with absolute value of camber, QBZ5 []:
      mask DialogControl QBZ6 Prompt: Bpt slope variation with square of camber, QBZ6 []:
      mask DialogControl QBZ9 Prompt: Br of Mzr slope scaling factor, QBZ9 []:
      mask DialogControl QBZ10 Prompt: Br of Mzr cornering stiffness factor, QBZ10 []:
      mask DialogControl QCZ1 Prompt: Cpt pneumatic trail shape factor, QCZ1 []:
      mask DialogControl QDZ1 Prompt: Dpt peak trail, QDZ1 []:
      mask DialogControl QDZ2 Prompt: Dpt peak trail variation with load, QDZ2 []:
      mask DialogControl QDZ3 Prompt: Dpt peak trail variation with camber, QDZ3 []:
      mask DialogControl QDZ4 Prompt: Dpt peak trail variation with square of camber, QDZ4 []:
      mask DialogControl QDZ6 Prompt: Dmr peak residual torque, QDZ6 []:
      mask DialogControl QDZ7 Prompt: Dmr peak residual torque variation with load, QDZ7 []:
      mask DialogControl QDZ8 Prompt: Dmr peak residual torque variation with camber, QDZ8 []:
      mask DialogControl QDZ9 Prompt: Dmr peak residual torque variation with camber and load, QDZ9 []:
      mask DialogControl QDZ10 Prompt: Dmr peak residual torque variation with square of camber, QDZ10 []:
      mask DialogControl QDZ11 Prompt: Dmr peak residual torque variation with square of load, QDZ11 []:
      mask DialogControl QEZ1 Prompt: Ept trail curvature at FZNOM, QEZ1 []:
      mask DialogControl QEZ2 Prompt: Ept variation with load, QEZ2 []:
      mask DialogControl QEZ3 Prompt: Ept variation with square of load, QEZ3 []:
      mask DialogControl QEZ4 Prompt: Ept variation with sign of alpha-t, QEZ4 []:
      mask DialogControl QEZ5 Prompt: Ept variation with sign of alpha-t and camber, QEZ5 []:
      mask DialogControl QHZ1 Prompt: Sht horizontal trail shift at FZNOM, QHZ1 []:
      mask DialogControl QHZ2 Prompt: Sht variation with load, QHZ2 []:
      mask DialogControl QHZ3 Prompt: Sht variation with camber, QHZ3 []:
      mask DialogControl QHZ4 Prompt: Sht variation with load and camber, QHZ4 []:
      mask DialogControl PPZ1 Prompt: Inflation pressure influence on trail length, PPZ1 []:
      mask DialogControl PPZ2 Prompt: Inflation pressure influence on residual aligning torque, PPZ2 []:
      mask DialogControl SSZ1 Prompt: Nominal value of s/R0: effect of Fx on Mz, SSZ1 []:
      mask DialogControl SSZ2 Prompt: s/R0 variation with lateral to nominal force ratio, SSZ2 []:
      mask DialogControl SSZ3 Prompt: s/R0 variation with camber, SSZ3 []:
      mask DialogControl SSZ4 Prompt: s/R0 variation with camber and load, SSZ4 []:
      mask DialogControl turnParamPanel Prompt: Turnslip
      mask DialogControl PDXP1 Prompt: Fx peak reduction due to spin, PDXP1 []:
      mask DialogControl PDXP2 Prompt: Fx peak reduction due to spin with varying load, PDXP2 []:
      mask DialogControl PDXP3 Prompt: Fx peak reduction due to spin with slip ratio, PDXP3 []:
      mask DialogControl PKYP1 Prompt: Cornering stiffness reduction due to spin, PKYP1 []:
      mask DialogControl PDYP1 Prompt: Fy peak reduction due to spin, PDYP1 []:
      mask DialogControl PDYP2 Prompt: Fy peak reduction due to spin with varying load, PDYP2 []:
      mask DialogControl PDYP3 Prompt: Fy peak reduction due to spin with slip angle, PDYP3 []:
      mask DialogControl PDYP4 Prompt: Fy peak reduction due to square root of spin, PDYP4 []:
      mask DialogControl PHYP1 Prompt: Fy vs. slip angle response lateral shift limit, PHYP1 []:
      mask DialogControl PHYP2 Prompt: Fy vs. slip angle response max lateral shift limit, PHYP2 []:
      mask DialogControl PHYP3 Prompt: Fy vs. slip angle response max lateral shift limit with load, PHYP3 []:
      mask DialogControl PHYP4 Prompt: Fy vs. slip angle response lateral shift curvature factor, PHYP4 []:
      mask DialogControl PECP1 Prompt: Camber stiffness reduction due to spin, PECP1 []:
      mask DialogControl PECP2 Prompt: Camber stiffness reduction due to spin with load, PECP2 []:
      mask DialogControl QDTP1 Prompt: Turn slip pneumatic trail reduction factor, QDTP1 []:
      mask DialogControl QCRP1 Prompt: Turn moment for constant turning and zero longitudinal speed, QCRP1 []:
      mask DialogControl QCRP2 Prompt: Turn slip moment increase with spin at 90deg slip angle, QCRP2 []:
      mask DialogControl QBRP1 Prompt: Residual spin torque reduction from side slip, QBRP1 []:
      mask DialogControl QDRP1 Prompt: Turn slip moment peak magnitude, QDRP1 []:
      mask DialogControl QDRP2 Prompt: Turn slip moment curvature, QDRP2 []:
      mask Display:
      | try
      |     IconInfo = vehdynicon('vehdynlibtire',gcb,8);
      | 
      |     image(IconInfo.image, IconInfo.position);
      | 
      |     for i = 1:numel(IconInfo.lconn)
      |         port_label('lconn', i, IconInfo.lconn{i})
      |     end
      | 
      |     for j = 1:numel(IconInfo.rconn)
      |         port_label('rconn', j, IconInfo.rconn{j})
      |     end
      | 
      |     for k = 1:numel(IconInfo.input)
      |         port_label('input', k, IconInfo.input{k})
      |     end
      | 
      |     for m = 1:numel(IconInfo.output)
      |         port_label('output', m, IconInfo.output{m})
      |     end
      | catch
      |     fprintf('2DOF \n Wheel')
      | end
  Fiala Wheel 2DOF : Subsystem  mask(Fiala Wheel 2DOF){BrakeType=Disc, rollingType=Pressure and velocity, vertType=None, Ckappa=1e7, Calpha=4.5e4, Cgamma=1e3, muMin=.8, muMax=1, Lrelx=.05, Lrely=.15, br=1e-3, IYY=0.74, omegao=0, NOMPRES=220000, LONGVL=16, UNLOADED_RADIUS=0.309384029954441, aMy=8e-4, bMy=.001, cMy=1.6e-4, alphaMy=-0.003, betaMy=0.97, QSY1=0.007, QSY2=0, QSY3=0.0015, QSY4=8.5e-05, QSY5=0, QSY6=0, QSY7=0.9, QSY8=-0.4, FNOMIN=4000, lam_My=1, VxMy=-20:1:20, FzMy=0:200:1e4, MyMap=[0,1114.7,4367.1,9707.2,17109,26554,38030,51524,67028,84533,1.0403e+05,1.2552e+05,1.4899e+05,1.7444e+05,2.0185e+05,2.3124e+05,2.6259e+05,2.959e+05,3.3117e+05,3.6839e+05,4.0756e+05,4.4868e+05,4.9174e+05,5.3675e+05,5.8369e+05,6.3257e+05,6.8338e+05,7.3613e+05,7.908e+05,8.474e+05,9.0593e+05,9.6638e+05,1.0288e+06,1.093e+06,1.1593e+06,1.2274e+06,1.2974e+06,1.3694e+06,1.4432e+06,1.519e+06,1.5967e+06,1.6763e+06,1.7578e+06,1.8412e+06,1.9265e+06,2.0137e+06,2.1028e+06,2.1938e+06,2.2867e+06,2.3815e+06,2.4782e+06 0,1024.5,4013.8,8921.9,15725,24406,34953,47356,61605,77694,95616,1.1537e+05,1.3694e+05,1.6032e+05,1.8553e+05,2.1254e+05,2.4135e+05,2.7197e+05,3.0438e+05,3.3859e+05,3.7459e+05,4.1238e+05,4.5196e+05,4.9333e+05,5.3647e+05,5.814e+05,6.281e+05,6.7658e+05,7.2683e+05,7.7885e+05,8.3264e+05,8.8821e+05,9.4553e+05,1.0046e+06,1.0655e+06,1.1281e+06,1.1925e+06,1.2586e+06,1.3265e+06,1.3961e+06,1.4675e+06,1.5407e+06,1.6156e+06,1.6922e+06,1.7706e+06,1.8508e+06,1.9327e+06,2.0163e+06,2.1017e+06,2.1889e+06,2.2777e+06 0,938.57,3677,8173.3,14405,22358,32020,43382,56436,71175,87593,1.0568e+05,1.2545e+05,1.4687e+05,1.6996e+05,1.947e+05,2.211e+05,2.4915e+05,2.7884e+05,3.1018e+05,3.4316e+05,3.7778e+05,4.1404e+05,4.5193e+05,4.9146e+05,5.3261e+05,5.754e+05,6.1981e+05,6.6584e+05,7.135e+05,7.6278e+05,8.1368e+05,8.6619e+05,9.2032e+05,9.7607e+05,1.0334e+06,1.0924e+06,1.153e+06,1.2152e+06,1.279e+06,1.3444e+06,1.4114e+06,1.48e+06,1.5502e+06,1.6221e+06,1.6955e+06,1.7705e+06,1.8471e+06,1.9254e+06,2.0052e+06,2.0866e+06 0,856.81,3356.7,7461.3,13151,20411,29231,39603,51520,64974,79962,96478,1.1452e+05,1.3408e+05,1.5515e+05,1.7774e+05,2.0184e+05,2.2744e+05,2.5455e+05,2.8316e+05,3.1327e+05,3.4487e+05,3.7797e+05,4.1256e+05,4.4864e+05,4.8621e+05,5.2527e+05,5.6581e+05,6.0784e+05,6.5134e+05,6.9633e+05,7.4279e+05,7.9073e+05,8.4015e+05,8.9104e+05,9.4341e+05,9.9724e+05,1.0525e+06,1.1093e+06,1.1676e+06,1.2273e+06,1.2885e+06,1.3511e+06,1.4152e+06,1.4808e+06,1.5478e+06,1.6163e+06,1.6862e+06,1.7576e+06,1.8305e+06,1.9048e+06 0,779.25,3052.9,6785.9,11960,18563,26585,36018,46856,59093,72724,87745,1.0415e+05,1.2194e+05,1.4111e+05,1.6165e+05,1.8357e+05,2.0685e+05,2.3151e+05,2.5753e+05,2.8491e+05,3.1365e+05,3.4376e+05,3.7522e+05,4.0803e+05,4.422e+05,4.7772e+05,5.1459e+05,5.5282e+05,5.9238e+05,6.333e+05,6.7556e+05,7.1916e+05,7.641e+05,8.1039e+05,8.5801e+05,9.0697e+05,9.5727e+05,1.0089e+06,1.0619e+06,1.1162e+06,1.1718e+06,1.2288e+06,1.2871e+06,1.3467e+06,1.4077e+06,1.47e+06,1.5336e+06,1.5985e+06,1.6648e+06,1.7324e+06 0,705.9,2765.5,6147.1,10834,16816,24083,32628,42446,53531,65879,79486,94348,1.1046e+05,1.2783e+05,1.4643e+05,1.6629e+05,1.8738e+05,2.0972e+05,2.3329e+05,2.5809e+05,2.8413e+05,3.114e+05,3.399e+05,3.6962e+05,4.0058e+05,4.3276e+05,4.6616e+05,5.0078e+05,5.3662e+05,5.7369e+05,6.1197e+05,6.5146e+05,6.9218e+05,7.3411e+05,7.7725e+05,8.216e+05,8.6717e+05,9.1394e+05,9.6193e+05,1.0111e+06,1.0615e+06,1.1131e+06,1.1659e+06,1.22e+06,1.2752e+06,1.3316e+06,1.3892e+06,1.4481e+06,1.5081e+06,1.5693e+06 0,636.76,2494.6,5545,9773.1,15169,21724,29432,38288,48287,59426,71700,85106,99642,1.153e+05,1.3209e+05,1.5e+05,1.6903e+05,1.8917e+05,2.1044e+05,2.3281e+05,2.563e+05,2.809e+05,3.066e+05,3.3342e+05,3.6134e+05,3.9037e+05,4.205e+05,4.5173e+05,4.8406e+05,5.1749e+05,5.5202e+05,5.8765e+05,6.2438e+05,6.622e+05,7.0111e+05,7.4112e+05,7.8223e+05,8.2442e+05,8.677e+05,9.1208e+05,9.5754e+05,1.0041e+06,1.0517e+06,1.1005e+06,1.1503e+06,1.2012e+06,1.2532e+06,1.3062e+06,1.3604e+06,1.4156e+06 0,571.82,2240.2,4979.5,8776.4,13622,19508,26430,34383,43363,53365,64388,76427,89480,1.0355e+05,1.1862e+05,1.347e+05,1.5179e+05,1.6988e+05,1.8897e+05,2.0907e+05,2.3016e+05,2.5225e+05,2.7534e+05,2.9942e+05,3.2449e+05,3.5056e+05,3.7761e+05,4.0566e+05,4.3469e+05,4.6472e+05,4.9573e+05,5.2772e+05,5.607e+05,5.9467e+05,6.2961e+05,6.6554e+05,7.0245e+05,7.4034e+05,7.7921e+05,8.1906e+05,8.5989e+05,9.017e+05,9.4448e+05,9.8824e+05,1.033e+06,1.0787e+06,1.1254e+06,1.173e+06,1.2216e+06,1.2712e+06 0,511.09,2002.3,4450.7,7844.3,12175,17436 ...(+15095 chars)], Fpl=10, Cr=1e-3, Kt=.008, Tmeas=298.15, Tamb=298.15, extTamb=off, WIDTH=0.209, bMz=0, mu_static=.3, mu_kinetic=.2, disk_abore=.05, Rm=.177, num_pads=2, drum_abore=0.0508, drum_a=0.123, drum_c=0.212, drum_r=0.15, drum_theta1=0, drum_theta2=126, brake_p_bpt=[1 11.4736842105263 21.9473684210526 32.4210526315789 42.8947368421053 53.3684210526316 63.8421052631579 74.3157894736842 84.7894736842105 95.2631578947368 105.736842105263 116.210526315789 126.684210526316 137.157894736842 147.631578947368 158.105263157895 168.578947368421 179.052631578947 189.526315789474 200], brake_n_bpt=[0 52.6315789473684 105.263157894737 157.894736842105 210.526315789474 263.157894736842 315.789473684211 368.421052631579 421.052631578947 473.684210526316 526.315789473684 578.947368421053 631.578947368421 684.210526315789 736.842105263158 789.473684210526 842.105263157895 894.736842105263 947.368421052632 1000], f_brake_t=[43.4900602404453 42.5056030554862 41.5350898940194 40.5780454442085 39.6340111501808 38.7025443887544 37.7832176914519 36.8756180088306 35.9793460143796 35.0940154454303 34.2192524787115 33.3546951383474 32.4999927342521 31.6548053290159 30.8188032315107 29.991666515561 29.1730845621415 28.362755623661 27.5603864089927 26.765691687993;498.991217495636 487.695866636631 476.560505099801 465.579679307235 454.748127933653 444.060772460445 433.51270824929 423.099196101319 412.81565427025 402.657650900201 392.620896861006 382.701238955775 372.894653477208 363.197240090814 353.605216024701 344.114910546964 334.722759712992 325.425301366216 316.219170376863 307.10109410434;954.492374750826 932.886130217776 911.585920305583 890.581313170261 869.862244717126 849.419000532136 829.242198807128 809.322774193808 789.651962526121 770.221286354971 751.0225412433 732.047782773203 713.289314220164 694.739674852612 676.391628817892 658.238154578366 640.272434863842 622.48784710877 604.877954344734 587.436496520688;1409.99353200602 1378.07639379892 1346.61133551136 1315.58294703329 1284.9763615006 1254.77722860383 1224.97168936497 1195.5463522863 1166.48827078199 1137.78492180974 1109.42418562559 1081.39432659063 1053.68397496312 1026.28210961441 999.178041611083 972.361398609768 945.822110014692 919.550392851325 893.536738312604 867.771898937035;1865.49468926121 1823.26665738007 1781.63675071715 1740.58458089631 1700.09047828407 1660.13545667552 1620.7011799228 1581.76993037878 1543.32457903786 1505.34855726451 1467.82583000789 1430.74087040806 1394.07863570608 1357.82454437621 1321.96445440427 1286.48464264117 1251.37178516554 1216.61293859388 1182.19552228048 1148.10730135338;2320.9958465164 2268.45692096121 2216.66216592293 2165.58621475934 2115.20459506754 2065.49368474721 2016.43067048064 1967.99350847127 1920.16088729373 1872.91219271928 1826.22747439018 1780.08741422549 1734.47329644903 1689.36697913801 1644.75086719747 1600.60788667257 1556.92146031639 1513.67548433643 1470.85430624835 1428.44270376973;2776.49700377159 2713.64718454235 2651.68758112871 2590.58784862237 2530.31871185102 2470.8519128189 2412.16016103848 2354.21708656376 2296.9971955496 2240.47582817405 2184.62911877248 2129.43395804292 2074.86795719199 2020.9094138998 1967.53727999066 1914.73113070398 1862.47113546724 1810.73803007899 1759.51309021622 1708.77810618608;3231.99816102678 3158.8374481235 3086.71299633449 3015.58948248539 2945.43282863449 2876.21014089059 2807.88965159632 2740.44066465625 2673.83350380547 2608.03946362882 2543.03076315477 2478.78050186034 2415.26261793494 2352.4518486616 2290.32369278385 2228.85437473538 2168.02081061809 2107.80057582154 2048.17187418409 1989.11350860242;3687.49931828197 3604.02771170464 3521.73841154027 3440.59111634842 3360.54694541796 3281.56836896228 3203.61914215416 3126.66424274874 3050.66981206134 2975.60309908359 2901.43240753707 2828.12704567777 2755.6572786779 2683.9942834234 2613.11010557704 2542.97761876678 2473.57048576894 2404.8631215641 2336.83065815196 2269.44891101877;4143.00047553716 4049.21797528579 3956.76382674606 3865.59275021144 3775.66106220143 3686.92659703397 3599.34863271199 3512.88782084123 3427.50612031721 3343.16673453836 3259.83405191936 3177.4735894952 3096.05193942085 3015.5367181852 2935.89651837023 2857.10086279818 2779.12016091979 2701.92566730665 2625.48944211983 2549.78431343512;4598.50163279235 4494.40823886693 4391.78924195184 4290.59438407447 4190.77517898491 4092.28482510566 3995.07812326983 3899.11139893372 3804.34242857308 3710.73036999313 3618.23569630166 3526.82013331263 3436.44660016381 3347.079152947 3258.68293116342 3171.22410682959 3084.66983607064 2998.98821304921 2914.1482260877 2830.11971585147;5054.00279004754 4939.59850244808 4826.81465715762 4715.59601793749 4605.88929576838 4497.64305317735 4390.80761382767 4285.3349770262 4181.17873682896 4078.2940054479 3976.63734068395 3876.16667713006 3776.84126090677 3678.62158770879 3581.46934395661 3485.34735086099 ...(+2764 chars)], MASS=9.46491996974568, zo=0, zdoto=0, GRAVITY=-9.81, VERTICAL_DAMPING=494.649255786991, VERTICAL_STIFFNESS=207885.061134007, zFz=[0 .01 .1], pFz=[10000 1000000], Fzz=[0 1e3 1e4; 0 1e4 1e5], zdotFz=[-20 0 20], Fzzdot=[500 0 -500;250 0 -250], FZMAX=10000, FZMIN=100, PRESMAX=1003118, PRESMIN=9982, KPUMAX=1, KPUMIN=-1, ALPMAX=1.5708, ALPMIN=-1.5708, CAMMAX=0.173, CAMMIN=-0.173, TMIN=0, TMAX=400, aMode=2}
      mask prompts: BrakeType "vdynblks:vehdynLatTire:blkPrm_BrakeType"; rollingType "autoblks_shared:autoblkLongitudinalWheel:blkPrm_rollingType"; vertType "vdynblks:vehdyntireFiala:blkPrm_vertType"; Ckappa "vdynblks:vehdyntireFiala:blkPrm_Ckappa"; Calpha "vdynblks:vehdyntireFiala:blkPrm_Calpha"; Cgamma "vdynblks:vehdyntireFiala:blkPrm_Cgamma"; muMin "vdynblks:vehdyntireFiala:blkPrm_muMin"; muMax "vdynblks:vehdyntireFiala:blkPrm_muMax"; Lrelx "vdynblks:vehdyntireFiala:blkPrm_Lrelx"; Lrely "vdynblks:vehdyntireFiala:blkPrm_Lrely"; br "vdynblks:vehdynLatTire:blkPrm_br"; IYY "vdynblks:vehdynLatTire:blkPrm_IYY"; omegao "vdynblks:vehdynLatTire:blkPrm_omegao"; NOMPRES "autoblks_shared:autoblkLongitudinalWheel:blkPrm_NOMPRES"; LONGVL "autoblks_shared:autoblkLongitudinalWheel:blkPrm_LONGVL"; UNLOADED_RADIUS "vdynblks:vehdynLatTire:blkPrm_UNLOADED_RADIUS"; aMy "vdynblks:vehdyntireFiala:blkPrm_aMy"; bMy "vdynblks:vehdyntireFiala:blkPrm_bMy"; cMy "vdynblks:vehdyntireFiala:blkPrm_cMy"; alphaMy "vdynblks:vehdyntireFiala:blkPrm_alphaMy"; betaMy "vdynblks:vehdyntireFiala:blkPrm_betaMy"; QSY1 "autoblks_shared:autoblkLongitudinalWheel:blkPrm_QSY1"; QSY2 "autoblks_shared:autoblkLongitudinalWheel:blkPrm_QSY2"; QSY3 "autoblks_shared:autoblkLongitudinalWheel:blkPrm_QSY3"; QSY4 "autoblks_shared:autoblkLongitudinalWheel:blkPrm_QSY4"; QSY5 "autoblks_shared:autoblkLongitudinalWheel:blkPrm_QSY5"; QSY6 "autoblks_shared:autoblkLongitudinalWheel:blkPrm_QSY6"; QSY7 "autoblks_shared:autoblkLongitudinalWheel:blkPrm_QSY7"; QSY8 "autoblks_shared:autoblkLongitudinalWheel:blkPrm_QSY8"; FNOMIN "autoblks_shared:autoblkLongitudinalWheel:blkPrm_FNOMIN"; lam_My "autoblks_shared:autoblkLongitudinalWheel:blkPrm_lam_My"; VxMy "autoblks_shared:autoblkLongitudinalWheel:blkPrm_VxMy"; FzMy "autoblks_shared:autoblkLongitudinalWheel:blkPrm_FzMy"; MyMap "autoblks_shared:autoblkLongitudinalWheel:blkPrm_MyMap"; Fpl "autoblks_shared:autoblkLongitudinalWheel:blkPrm_Fpl"; Cr "autoblks_shared:autoblkLongitudinalWheel:blkPrm_Cr"; Kt "autoblks_shared:autoblkLongitudinalWheel:blkPrm_Kt"; Tmeas "autoblks_shared:autoblkLongitudinalWheel:blkPrm_Tmeas"; Tamb "autoblks_shared:autoblkLongitudinalWheel:blkPrm_Tamb"; extTamb "autoblks_shared:autoblkLongitudinalWheel:blkPrm_extTamb"; WIDTH "vdynblks:vehdynLatTire:blkPrm_WIDTH"; bMz "vdynblks:vehdyntireFiala:blkPrm_bMz"; mu_static "autoblks_shared:autoblkLongitudinalWheel:blkPrm_mu_static"; mu_kinetic "autoblks_shared:autoblkLongitudinalWheel:blkPrm_mu_kinetic"; disk_abore "autoblks_shared:autoblkLongitudinalWheel:blkPrm_disk_abore"; Rm "autoblks_shared:autoblkLongitudinalWheel:blkPrm_Rm"; num_pads "autoblks_shared:autoblkLongitudinalWheel:blkPrm_num_pads"; drum_abore "autoblks_shared:autoblkLongitudinalWheel:blkPrm_drum_abore"; drum_a "autoblks_shared:autoblkLongitudinalWheel:blkPrm_drum_a"; drum_c "autoblks_shared:autoblkLongitudinalWheel:blkPrm_drum_c"; drum_r "autoblks_shared:autoblkLongitudinalWheel:blkPrm_drum_r"; drum_theta1 "autoblks_shared:autoblkLongitudinalWheel:blkPrm_drum_theta1"; drum_theta2 "autoblks_shared:autoblkLongitudinalWheel:blkPrm_drum_theta2"; brake_p_bpt "autoblks_shared:autoblkLongitudinalWheel:blkPrm_brake_p_bpt"; brake_n_bpt "autoblks_shared:autoblkLongitudinalWheel:blkPrm_brake_n_bpt"; f_brake_t "autoblks_shared:autoblkLongitudinalWheel:blkPrm_f_brake_t"; MASS "vdynblks:vehdynLatTire:blkPrm_MASS"; zo "vdynblks:vehdynLatTire:blkPrm_zo"; zdoto "vdynblks:vehdynLatTire:blkPrm_zdoto"; GRAVITY "vdynblks:vehdynLatTire:blkPrm_GRAVITY"; VERTICAL_DAMPING "vdynblks:vehdynLatTire:blkPrm_VERTICAL_DAMPING"; VERTICAL_STIFFNESS "vdynblks:vehdynLatTire:blkPrm_VERTICAL_STIFFNESS"; zFz "vdynblks:vehdyntireFiala:blkPrm_zFz"; pFz "vdynblks:vehdyntireFiala:blkPrm_pFz"; Fzz "vdynblks:vehdyntireFiala:blkPrm_Fzz"; zdotFz "vdynblks:vehdyntireFiala:blkPrm_zdotFz"; Fzzdot "vdynblks:vehdyntireFiala:blkPrm_Fzzdot"; FZMAX "vdynblks:vehdynLatTire:blkPrm_FZMAX"; FZMIN "vdynblks:vehdynLatTire:blkPrm_FZMIN"; PRESMAX "vdynblks:vehdynLatTire:blkPrm_PRESMAX"; PRESMIN "vdynblks:vehdynLatTire:blkPrm_PRESMIN"; KPUMAX "vdynblks:vehdynLatTire:blkPrm_KPUMAX"; KPUMIN "vdynblks:vehdynLatTire:blkPrm_KPUMIN"; ALPMAX "vdynblks:vehdynLatTire:blkPrm_ALPMAX"; ALPMIN "vdynblks:vehdynLatTire:blkPrm_ALPMIN"; CAMMAX "vdynblks:vehdynLatTire:blkPrm_CAMMAX"; CAMMIN "vdynblks:vehdynLatTire:blkPrm_CAMMIN"; TMIN "autoblks_shared:autoblkLongitudinalWheel:blkPrm_TMIN"; TMAX "autoblks_shared:autoblkLongitudinalWheel:blkPrm_TMAX"
      mask help: vdynblks:vehdyntireFiala:blkDesc
      mask init:
      | [~]=vehdynicon('vehdynlibtirefiala',gcb,0)
      mask Help: eval('vdynblkshelp(''vbtirefiala'')')
      mask TypeOptions BrakeType: autoblks_shared:autoblkLongitudinalWheel:blkCmb_BrakeType_c1 | autoblks_shared:autoblkLongitudinalWheel:blkCmb_BrakeType_c2 | autoblks_shared:autoblkLongitudinalWheel:blkCmb_BrakeType_c3 | autoblks_shared:autoblkLongitudinalWheel:blkCmb_BrakeType_c4
      mask Callback BrakeType: [~]=vehdynicon('vehdynlibtirefiala',gcb,2)
      mask TypeOptions rollingType: autoblks_shared:autoblkLongitudinalWheel:blkCmb_rollingType_c1 | autoblks_shared:autoblkLongitudinalWheel:blkCmb_rollingType_c2 | autoblks_shared:autoblkLongitudinalWheel:blkCmb_rollingType_c5 | autoblks_shared:autoblkLongitudinalWheel:blkCmb_rollingType_c3 | autoblks_shared:autoblkLongitudinalWheel:blkCmb_rollingType_c4
      mask Callback rollingType: [~]=vehdynicon('vehdynlibtirefiala',gcb,1)
      mask TypeOptions vertType: vdynblks:vehdyntireFiala:blkCmb_vertType_c1 | vdynblks:vehdyntireFiala:blkCmb_vertType_c2
      mask Callback vertType: [~]=vehdynicon('vehdynlibtirefiala',gcb,5)
      mask DialogControl BlockOptions Prompt: autoblks_shared:autoblkLongitudinalWheel:blkDlg_BlockOptions
      mask DialogControl BrakeType Prompt: Brake Type:
      mask DialogControl rollingType Prompt: Rolling Resistance:
      mask DialogControl vertType Prompt: Vertical Motion:
      mask DialogControl longlatParamPanel Prompt: Longitudinal and Lateral
      mask DialogControl Ckappa Prompt: Longitudinal stiffness, Ckappa [N]:
      mask DialogControl Calpha Prompt: Lateral stiffness per slip angle, Calpha [N/rad]:
      mask DialogControl Cgamma Prompt: Camber stiffness, Cgamma [N/rad]:
      mask DialogControl muMin Prompt: Kinematic friction, muMin []:
      mask DialogControl muMax Prompt: Static friction, muMax []:
      mask DialogControl Lrelx Prompt: Longitudinal relaxation length, Lrelx [m]:
      mask DialogControl Lrely Prompt: Lateral relaxation length, Lrely [m/rad]:
      mask DialogControl rollingParamPanel Prompt: Rolling
      mask DialogControl br Prompt: Rotational damping, br [N*m*s/rad]:
      mask DialogControl IYY Prompt: Rotational inertia (rolling axis), IYY [kg*m^2]:
      mask DialogControl omegao Prompt: Initial rotational velocity, omegao [rad/s]:
      mask DialogControl NOMPRES Prompt: Nominal inflation pressure, NOMPRES [Pa]:
      mask DialogControl LONGVL Prompt: Nominal longitudinal speed, LONGVL [m/s]:
      mask DialogControl UNLOADED_RADIUS Prompt: Unloaded radius, UNLOADED_RADIUS [m]:
      mask DialogControl SimpMyParams Prompt: autoblks_shared:autoblkLongitudinalWheel:blkDlg_SimpMyParams
      mask DialogControl aMy Prompt: Velocity independent force coefficient, aMy []:
      mask DialogControl bMy Prompt: Linear velocity force component, bMy [s/m]:
      mask DialogControl cMy Prompt: Quadratic velocity force component, cMy [s^2/m^2]:
      mask DialogControl alphaMy Prompt: Tire pressure exponent, alphaMy []:
      mask DialogControl betaMy Prompt: Normal force exponent, betaMy []:
      mask DialogControl MagicMyParams Prompt: autoblks_shared:autoblkLongitudinalWheel:blkDlg_MagicMyParams
      mask DialogControl QSY1 Prompt: Rolling resistance torque coefficient, QSY1 []:
      mask DialogControl QSY2 Prompt: Longitudinal force rolling resistance coefficient, QSY2 []:
      mask DialogControl QSY3 Prompt: Linear rotational speed rolling resistance coefficient, QSY3 []:
      mask DialogControl QSY4 Prompt: Quartic rotational speed rolling resistance coefficient, QSY4 []:
      mask DialogControl QSY5 Prompt: Camber squared rolling resistance torque, QSY5 [1/rad^2]:
      mask DialogControl QSY6 Prompt: Load based camber squared rolling resistance torque, QSY6 [1/rad^2]:
      mask DialogControl QSY7 Prompt: Normal load rolling resistance coefficient, QSY7 []:
      mask DialogControl QSY8 Prompt: Pressure load rolling resistance coefficient, QSY8 []:
      mask DialogControl FNOMIN Prompt: Nominal normal force, FNOMIN [N]:
      mask DialogControl lam_My Prompt: Rolling resistance scaling factor, lam_My []:
      mask DialogControl MappedMyParams Prompt: autoblks_shared:autoblkLongitudinalWheel:blkDlg_MappedMyParams
      mask DialogControl VxMy Prompt: Spin axis velocity breakpoints, VxMy [m/s]:
      mask DialogControl FzMy Prompt: Normal force breakpoints, FzMy [N]:
      mask DialogControl MyMap Prompt: Rolling resistance torque map, MyMap [Nm]:
      mask DialogControl plotMyMap Prompt: autoblks_shared:autoblkLongitudinalWheel:blkDlg_plotMyMap
      mask DialogControl plotMyMap Callback: [~]=vehdynicon('vehdynlibtirefiala',gcb,4)
      mask DialogControl ISOMyParams Prompt: ISO 28580
      mask DialogControl Fpl Prompt: Parasitic losses force, Fpl [N]:
      mask DialogControl Cr Prompt: Rolling resistance constant, Cr [N/kN]:
      mask DialogControl Kt Prompt: Thermal correction factor, Kt [1/degC]:
      mask DialogControl Tmeas Prompt: Measured temperature, Tmeas [K]:
      mask DialogControl Tamb Prompt: Ambient temperature, Tamb [K]:
      mask DialogControl extTamb Prompt: Input ambient temperature
      mask DialogControl alignParamPannel Prompt: Aligning
      mask DialogControl WIDTH Prompt: Wheel width, WIDTH [m]:
      mask DialogControl bMz Prompt: Linear yaw rate resistance, bMz [N*m*s/rad]:
      mask DialogControl brakeParamPanel Prompt: autoblks_shared:autoblkLongitudinalWheel:blkDlg_brakeParamPanel
      mask DialogControl GenParams Prompt: autoblks_shared:autoblkLongitudinalWheel:blkDlg_GenParams
      mask DialogControl mu_static Prompt: Static friction coefficient, mu_static []:
      mask DialogControl mu_kinetic Prompt: Kinetic friction coefficient, mu_kinetic []:
      mask DialogControl DiskBrakeParms Prompt: autoblks_shared:autoblkLongitudinalWheel:blkDlg_DiskBrakeParms
      mask DialogControl disk_abore Prompt: Disc brake actuator bore, disk_abore [m]:
      mask DialogControl Rm Prompt: Brake pad mean radius, Rm [m]:
      mask DialogControl num_pads Prompt: Number of brake pads, num_pads []:
      mask DialogControl DrumBrakeParms Prompt: autoblks_shared:autoblkLongitudinalWheel:blkDlg_DrumBrakeParms
      mask DialogControl drum_abore Prompt: Drum brake actuator bore, drum_abore [m]:
      mask DialogControl drum_a Prompt: Shoe pin to drum center distance, drum_a [m]:
      mask DialogControl drum_c Prompt: Shoe pin center to force application point distance, drum_c [m]:
      mask DialogControl drum_r Prompt: Drum internal radius, drum_r [m]:
      mask DialogControl drum_theta1 Prompt: Shoe pin to pad start angle, drum_theta1 [deg]:
      mask DialogControl drum_theta2 Prompt: Shoe pin to pad end angle, drum_theta2 [deg]:
      mask DialogControl MappedBrakeParms Prompt: autoblks_shared:autoblkLongitudinalWheel:blkDlg_MappedBrakeParms
      mask DialogControl brake_p_bpt Prompt: Brake actuator pressure breakpoints, brake_p_bpt [bar]:
      mask DialogControl brake_n_bpt Prompt: Wheel speed breakpoints, brake_n_bpt [rpm]:
      mask DialogControl f_brake_t Prompt: Brake torque map, f_brake_t [Nm]:
      mask DialogControl PlotBrakeTorqueMap Prompt: autoblks_shared:autoblkLongitudinalWheel:blkDlg_PlotBrakeTorqueMap
      mask DialogControl PlotBrakeTorqueMap Callback: [~]=vehdynicon('vehdynlibtirefiala',gcb,3)
      mask DialogControl vertParamPannel Prompt: Vertical
      mask DialogControl MASS Prompt: Wheel mass, MASS [kg]:
      mask DialogControl zo Prompt: Initial tire deflection, zo [m]:
      mask DialogControl zdoto Prompt: Initial wheel vertical velocity (wheel fixed frame), zdoto [m/s]:
      mask DialogControl GRAVITY Prompt: Gravity, GRAVITY [m/s^2]:
      mask DialogControl vertLinearParam Prompt: Linear stiffness and damping
      mask DialogControl VERTICAL_DAMPING Prompt: Vertical tire damping, VERTICAL_DAMPING [N*s/m]:
      mask DialogControl VERTICAL_STIFFNESS Prompt: Vertical tire stiffness, VERTICAL_STIFFNESS [N/m]:
      mask DialogControl vertMappedParam Prompt: Vertical mapped stiffness and damping
      mask DialogControl zFz Prompt: Vertical deflection breakpoints, zFz [m]:
      mask DialogControl pFz Prompt: Pressure breakpoints, pFz [Pa]:
      mask DialogControl Fzz Prompt: Force due to deflection, Fzz [N]:
      mask DialogControl zdotFz Prompt: Vertical velocity breakpoints, zdotFz [m/s]:
      mask DialogControl Fzzdot Prompt: Force due to velocity, Fzzdot [N]:
      mask DialogControl simParamPannel Prompt: Simulation
      mask DialogControl FZMAX Prompt: Maximum normal force, FZMAX [N]:
      mask DialogControl FZMIN Prompt: Minimum normal force, FZMIN [N]:
      mask DialogControl PRESMAX Prompt: Maximum pressure, PRESMAX [Pa]:
      mask DialogControl PRESMIN Prompt: Minimum pressure, PRESMIN [Pa]:
      mask DialogControl KPUMAX Prompt: Max allowable slip ratio (absolute), KPUMAX []:
      mask DialogControl KPUMIN Prompt: Minimum allowable slip ratio (absolute), KPUMIN []:
      mask DialogControl ALPMAX Prompt: Max allowable slip angle (absolute), ALPMAX [rad]:
      mask DialogControl ALPMIN Prompt: Minimum allowable slip angle (absolute), ALPMIN [rad]:
      mask DialogControl CAMMAX Prompt: Maximum allowable camber angle, CAMMAX [rad]:
      mask DialogControl CAMMIN Prompt: Minimum allowable camber angle, CAMMIN [rad]:
      mask DialogControl TMIN Prompt: Minimum ambient temperature, TMIN, [K]:
      mask DialogControl TMAX Prompt: Maximum ambient temperature, TMAX [K]:
      mask Display:
      | try
      |     IconInfo = vehdynicon('vehdynlibtirefiala',gcb,8);
      | 
      |     image(IconInfo.image, IconInfo.position);
      | 
      |     for i = 1:numel(IconInfo.lconn)
      |         port_label('lconn', i, IconInfo.lconn{i})
      |     end
      | 
      |     for j = 1:numel(IconInfo.rconn)
      |         port_label('rconn', j, IconInfo.rconn{j})
      |     end
      | 
      |     for k = 1:numel(IconInfo.input)
      |         port_label('input', k, IconInfo.input{k})
      |     end
      | 
      |     for m = 1:numel(IconInfo.output)
      |         port_label('output', m, IconInfo.output{m})
      |     end
      | catch
      |     fprintf('2DOF \n Wheel')
      | end
  Longitudinal Wheel - Disc Brake : autolibshared/Longitudinal Wheel  FxType=Magic Formula constant value  rollingType=None  BrakeType=Disc  vertType=None  lam_x=1  extMu=off  aMode=2  br=0.001  Iyy=0.8  omegao=0  Lrel=0.5  Re=0.3  UNLOADED_RADIUS=0.4  LONGVL=16  gamma=0  NOMPRES=220000  press=220000  extPress=off  Dx=1  Cx=1.65  Bx=10  Ex=0.01  PCX1=1.6  PDX1=1  PDX2=-0.08  PDX3=0  PEX1=0.112  PEX2=0.313  PEX3=0  PEX4=0.0016  PKX1=21.7  PKX2=13.77  PKX3=-0.412  PHX1=2.1585E-4  PHX2=0.00115  PVX1=1.5973E-5  PVX2=1.043E-4  PPX1=-0.3489  PPX2=0.382  PPX3=-0.09634  PPX4=0.06447  lam_muV=1  lam_Kxkappa=1  lam_Cx=1  lam_Ex=0  lam_Hx=1  lam_Vx=1  kappaFx=[-1,-0.78476,-0.61585,-0.48329,-0.37927,-0.29764,-0.23357,-0.1833,-0.14384,-0.11288,-0.088587,-0.069519,-0.054556,-0.042813,-0.033598,-0.026367,-0.020691,-0.016238,-0.012743,-0.01,0.01,0.012743,0.016238,0.020691,0.026367,0.033598,0.042813,0.054556,0.069519,0.088587,0.11288,0.14384,0.1833,0.23357,0.29764,0.37927,0.48329,0.61585,0.78476,1]  FzFx=[0,200,400,600,800,1000,1200,1400,1600,1800,2000,2200,2400,2600,2800,3000,3200,3400,3600,3800,4000,4200,4400,4600,4800,5000,5200,5400,5600,5800,6000,6200,6400,6600,6800,7000,7200,7400,7600,7800,8000,8200,8400,8600,8800,9000,9200,9400,9600,9800,10000]  FxMap=|  aMy=84e-4  bMy=6.2e-4  cMy=1.6e-4  alphaMy=-0.003  betaMy=0.97  QSY1=0.007  QSY2=0  QSY3=0.0015  QSY4=8.5e-05  QSY5=0  QSY6=0  QSY7=0.9  QSY8=-0.4  lam_My=1  VxMy=-20:1:20  FzMy=0:200:1e4  MyMap=|  Fpl=10  Cr=1e-3  Kt=.008  Tmeas=25  Tamb=298.15  extTamb=off  mu_static=0.3  mu_kinetic=0.2  disk_abore=0.05  Rm=0.1778  num_pads=2  drum_abore=0.0508  drum_a=0.123  drum_c=0.212  drum_r=0.15  drum_theta1=0  drum_theta2=126  brake_p_bpt=[1 11.4736842105263 21.9473684210526 32.4210526315789 42.8947368421053 53.3684210526316 63.8421052631579 74.3157894736842 84.7894736842105 95.2631578947368 105.736842105263 116.210526315789 126.684210526316 137.157894736842 147.631578947368 158.105263157895 168.578947368421 179.052631578947 189.526315789474 200]  brake_n_bpt=[0 52.6315789473684 105.263157894737 157.894736842105 210.526315789474 263.157894736842 315.789473684211 368.421052631579 421.052631578947 473.684210526316 526.315789473684 578.947368421053 631.578947368421 684.210526315789 736.842105263158 789.473684210526 842.105263157895 894.736842105263 947.368421052632 1000]  f_brake_t=[43.4900602404453 42.5056030554862 41.5350898940194 40.5780454442085 39.6340111501808 38.7025443887544 37.7832176914519 36.8756180088306 35.9793460143796 35.0940154454303 34.2192524787115 33.3546951383474 32.4999927342521 31.6548053290159 30.8188032315107 29.991666515561 29.1730845621415 28.362755623661 27.5603864089927 26.765691687993;498.991217495636 487.695866636631 476.560505099801 465.579679307235 454.748127933653 444.060772460445 433.51270824929 423.099196101319 412.81565427025 402.657650900201 392.620896861006 382.701238955775 372.894653477208 363.197240090814 353.605216024701 344.114910546964 334.722759712992 325.425301366216 316.219170376863 307.10109410434;954.492374750826 932.886130217776 911.585920305583 890.581313170261 869.862244717126 849.419000532136 829.242198807128 809.322774193808 789.651962526121 770.221286354971 751.0225412433 732.047782773203 713.289314220164 694.739674852612 676.391628817892 658.238154578366 640.272434863842 622.48784710877 604.877954344734 587.436496520688;1409.99353200602 1378.07639379892 1346.61133551136 1315.58294703329 1284.9763615006 1254.77722860383 1224.97168936497 1195.5463522863 1166.48827078199 1137.78492180974 1109.42418562559 1081.39432659063 1053.68397496312 1026.28210961441 999.178041611083 972.361398609768 945.822110014692 919.550392851325 893.536738312604 867.771898937035;1865.49468926121 1823.26665738007 1781.63675071715 1740.58458089631 1700.09047828407 1660.13545667552 1620.7011799228 1581.76993037878 1543.32457903786 1505.34855726451 1467.82583000789 1430.74087040806 1394.07863570608 1357.82454437621 1321.96445440427 1286.48464264117 1251.37178516554 1216.61293859388 1182.19552228048 1148.10730135338;2320.9958465164 2268.45692096121 2216.66216592293 2165.58621475934 2115.20459506754 2065.49368474721 2016.43067048064 1967.99350847127 1920.16088729373 1872.91219271928 1826.22747439018 1780.08741422549 1734.47329644903 1689.36697913801 1644.75086719747 1600.60788667257 1556.92146031639 1513.67548433643 1470.85430624835 1428.44270376973;2776.49700377159 2713.64718454235 2651.68758112871 2590.58784862237 2530.31871185102 2470.8519128189 2412.16016103848 2354.21708656376 2296.9971955496 2240.47582817405 2184.62911877248 2129.43395804292 2074.86795719199 2020.9094138998 1967.53727999066 1914.73113070398 1862.47113546724 1810.73803007899 1759.51309021622 1708.77810618608;3231.99816102678 3158.8374481235 3086.71299633449 3015.58948248539 2945.43282863449 2876.21014089059 2807.88965159632 2740.44066465625 2673.83350380547 2608.03946362882 2543.03076315477 2478.78050186034 2415.26261793494 2352.4518486616 2290.32369278385 2228.85437473538 2168.02081061809 2107.80057582154 2048.17187418409 1989.11350860242;3687.49931828197 3604.02771170464 3521.73841154027 3440.59111634842 3360.54694541796 3281.56836896228 3203.61914215416 3126.66424274874 3050.66981206134 2975.60309908359 2901.43240753707 2828.12704567777 2755.6572786779 2683.9942834234 2613.11010557704 2542.97761876678 2473.57048576894 2404.8631215641 2336.83065815196 2269.44891101877;4143.00047553716 4049.21797528579 3956.76382674606 3865.59275021144 3775.66106220143 3686.92659703397 3599.34863271199 3512.88782084123 3427.50612031721 3343.16673453836 3259.83405191936 3177.4735894952 3096.05193942085 3015.5367181852 2935.89651837023 2857.10086279818 2779.12016091979 2701.92566730665 2625.48944211983 2549.78431343512;4598.50163279235 4494.40823886693 4391.78924195184 4290.59438407447 4190.77517898491 4092.28482510566 3995.07812326983 3899.11139893372 3804.34242857308 3710.73036999313 3618.23569630166 3526.82013331263 3436.44660016381 3347.079152947 3258.68293116342 3171.22410682959 3084.66983607064 2998.98821304921 2914.1482260877 2830.11971585147;5054.00279004754 4939.59850244808 4826.81465715762 4715.59601793749 4605.88929576838 4497.64305317735 4390.80761382767 4285.3349770262 4181.17873682896 4078.2940054479 3976.63734068395 3876.16667713006 3776.84126090677 3678.62158770879 3581.46934395661 3485.34735086099 ...(+2764 chars)]  FNOMIN=2000  lam_Fzo=1  m=10  zo=0  zdoto=0  g=9.81  VERTICAL_STIFFNESS=209000.0  VERTICAL_DAMPING=50  Q_RE0=.99  Q_V1=0  Q_V2=0.047  Q_FZ1=0  Q_FZ2=15.4  Q_FCX=0.134  Q_FCY=.11  Q_CAM=0  PFZ1=0.71  Q_FCY2=-0.48  Q_CAM1=85.2  Q_CAM2=257.0  Q_CAM3=0.512  Q_FYS1=-204500.0  Q_FYS2=-60000  Q_FYS3=88211.7  BOTTOM_OFFST=.01  BOTTOM_STIFF=2000000  zFz=[0 .01 .1]  pFz=[10000 1000000]  Fzz=[0 1e3 1e4; 0 1e4 1e5]  zdotFz=[-20 0 20]  Fzzdot=[500 0 -500;250 0 -250]  Gndz=0  extGnd=off  FZMIN=0  FZMAX=10000  PRESMIN=10000  PRESMAX=1000000  kappamax=1.5  VXLOW=1  TMIN=0  TMAX=400  blkID=0
      FxMap=|
      | [-0,-131.22,-262.44,-393.66,-524.88,-656.1,-787.32,-918.54,-1049.8,-1181,-1312.2,-1443.4,-1574.6,-1705.9,-1837.1,-1968.3,-2099.5,-2230.7,-2362,-2493.2,-2624.4,-2755.6,-2886.8,-3018.1,-3149.3,-3280.5,-3411.7,-3542.9,-3674.2,-3805.4,-3936.6,-4067.8,-4199,-4330.2,-4461.5,-4592.7,-4723.9,-4855.1,-4986.3,-5117.6,-5248.8,-5380,-5511.2,-5642.4,-5773.7,-5904.9,-6036.1,-6167.3,-6298.5,-6429.8,-6561
      | -0,-137.87,-275.75,-413.62,-551.49,-689.36,-827.24,-965.11,-1103,-1240.9,-1378.7,-1516.6,-1654.5,-1792.3,-1930.2,-2068.1,-2206,-2343.8,-2481.7,-2619.6,-2757.5,-2895.3,-3033.2,-3171.1,-3308.9,-3446.8,-3584.7,-3722.6,-3860.4,-3998.3,-4136.2,-4274,-4411.9,-4549.8,-4687.7,-4825.5,-4963.4,-5101.3,-5239.2,-5377,-5514.9,-5652.8,-5790.6,-5928.5,-6066.4,-6204.3,-6342.1,-6480,-6617.9,-6755.8,-6893.6
      | -0,-145.88,-291.75,-437.63,-583.5,-729.38,-875.25,-1021.1,-1167,-1312.9,-1458.8,-1604.6,-1750.5,-1896.4,-2042.3,-2188.1,-2334,-2479.9,-2625.8,-2771.6,-2917.5,-3063.4,-3209.3,-3355.1,-3501,-3646.9,-3792.8,-3938.6,-4084.5,-4230.4,-4376.3,-4522.1,-4668,-4813.9,-4959.8,-5105.6,-5251.5,-5397.4,-5543.3,-5689.1,-5835,-5980.9,-6126.8,-6272.6,-6418.5,-6564.4,-6710.3,-6856.1,-7002,-7147.9,-7293.8
      | -0,-155.26,-310.53,-465.79,-621.05,-776.32,-931.58,-1086.8,-1242.1,-1397.4,-1552.6,-1707.9,-1863.2,-2018.4,-2173.7,-2328.9,-2484.2,-2639.5,-2794.7,-2950,-3105.3,-3260.5,-3415.8,-3571.1,-3726.3,-3881.6,-4036.8,-4192.1,-4347.4,-4502.6,-4657.9,-4813.2,-4968.4,-5123.7,-5278.9,-5434.2,-5589.5,-5744.7,-5900,-6055.3,-6210.5,-6365.8,-6521.1,-6676.3,-6831.6,-6986.8,-7142.1,-7297.4,-7452.6,-7607.9,-7763.2
      | -0,-165.86,-331.71,-497.57,-663.43,-829.28,-995.14,-1161,-1326.9,-1492.7,-1658.6,-1824.4,-1990.3,-2156.1,-2322,-2487.8,-2653.7,-2819.6,-2985.4,-3151.3,-3317.1,-3483,-3648.8,-3814.7,-3980.6,-4146.4,-4312.3,-4478.1,-4644,-4809.8,-4975.7,-5141.5,-5307.4,-5473.3,-5639.1,-5805,-5970.8,-6136.7,-6302.5,-6468.4,-6634.3,-6800.1,-6966,-7131.8,-7297.7,-7463.5,-7629.4,-7795.2,-7961.1,-8127,-8292.8
      | -0,-177.09,-354.19,-531.28,-708.38,-885.47,-1062.6,-1239.7,-1416.8,-1593.8,-1770.9,-1948,-2125.1,-2302.2,-2479.3,-2656.4,-2833.5,-3010.6,-3187.7,-3364.8,-3541.9,-3719,-3896.1,-4073.2,-4250.3,-4427.4,-4604.5,-4781.5,-4958.6,-5135.7,-5312.8,-5489.9,-5667,-5844.1,-6021.2,-6198.3,-6375.4,-6552.5,-6729.6,-6906.7,-7083.8,-7260.9,-7438,-7615.1,-7792.1,-7969.2,-8146.3,-8323.4,-8500.5,-8677.6,-8854.7
      | -0,-187.84,-375.67,-563.51,-751.35,-939.18,-1127,-1314.9,-1502.7,-1690.5,-1878.4,-2066.2,-2254,-2441.9,-2629.7,-2817.5,-3005.4,-3193.2,-3381.1,-3568.9,-3756.7,-3944.6,-4132.4,-4320.2,-4508.1,-4695.9,-4883.7,-5071.6,-5259.4,-5447.3,-5635.1,-5822.9,-6010.8,-6198.6,-6386.4,-6574.3,-6762.1,-6949.9,-7137.8,-7325.6,-7513.5,-7701.3,-7889.1,-8077,-8264.8,-8452.6,-8640.5,-8828.3,-9016.1,-9204,-9391.8
      | -0,-196.25,-392.49,-588.74,-784.98,-981.23,-1177.5,-1373.7,-1570,-1766.2,-1962.5,-2158.7,-2354.9,-2551.2,-2747.4,-2943.7,-3139.9,-3336.2,-3532.4,-3728.7,-3924.9,-4121.2,-4317.4,-4513.6,-4709.9,-4906.1,-5102.4,-5298.6,-5494.9,-5691.1,-5887.4,-6083.6,-6279.9,-6476.1,-6672.3,-6868.6,-7064.8,-7261.1,-7457.3,-7653.6,-7849.8,-8046.1,-8242.3,-8438.6,-8634.8,-8831,-9027.3,-9223.5,-9419.8,-9616,-9812.3
      | -0,-199.97,-399.95,-599.92,-799.9,-999.87,-1199.8,-1399.8,-1599.8,-1799.8,-1999.7,-2199.7,-2399.7,-2599.7,-2799.6,-2999.6,-3199.6,-3399.6,-3599.5,-3799.5,-3999.5,-4199.5,-4399.4,-4599.4,-4799.4,-4999.4,-5199.3,-5399.3,-5599.3,-5799.2,-5999.2,-6199.2,-6399.2,-6599.1,-6799.1,-6999.1,-7199.1,-7399,-7599,-7799,-7999,-8198.9,-8398.9,-8598.9,-8798.9,-8998.8,-9198.8,-9398.8,-9598.8,-9798.7,-9998.7
      | -0,-196.87,-393.74,-590.6,-787.47,-984.34,-1181.2,-1378.1,-1574.9,-1771.8,-1968.7,-2165.5,-2362.4,-2559.3,-2756.2,-2953,-3149.9,-3346.8,-3543.6,-3740.5,-3937.4,-4134.2,-4331.1,-4528,-4724.8,-4921.7,-5118.6,-5315.4,-5512.3,-5709.2,-5906,-6102.9,-6299.8,-6496.6,-6693.5,-6890.4,-7087.2,-7284.1,-7481,-7677.8,-7874.7,-8071.6,-8268.5,-8465.3,-8662.2,-8859.1,-9055.9,-9252.8,-9449.7,-9646.5,-9843.4
      | -0,-186.02,-372.04,-558.06,-744.08,-930.1,-1116.1,-1302.1,-1488.2,-1674.2,-1860.2,-2046.2,-2232.2,-2418.3,-2604.3,-2790.3,-2976.3,-3162.3,-3348.4,-3534.4,-3720.4,-3906.4,-4092.4,-4278.5,-4464.5,-4650.5,-4836.5,-5022.5,-5208.6,-5394.6,-5580.6,-5766.6,-5952.6,-6138.7,-6324.7,-6510.7,-6696.7,-6882.7,-7068.7,-7254.8,-7440.8,-7626.8,-7812.8,-7998.8,-8184.9,-8370.9,-8556.9,-8742.9,-8928.9,-9115,-9301
      | -0,-168.44,-336.89,-505.33,-673.78,-842.22,-1010.7,-1179.1,-1347.6,-1516,-1684.4,-1852.9,-2021.3,-2189.8,-2358.2,-2526.7,-2695.1,-2863.5,-3032,-3200.4,-3368.9,-3537.3,-3705.8,-3874.2,-4042.7,-4211.1,-4379.5,-4548,-4716.4,-4884.9,-5053.3,-5221.8,-5390.2,-5558.6,-5727.1,-5895.5,-6064,-6232.4,-6400.9,-6569.3,-6737.8,-6906.2,-7074.6,-7243.1,-7411.5,-7580,-7748.4,-7916.9,-8085.3,-8253.7,-8422.2
      | -0,-146.7,-293.4,-440.1,-586.81,-733.51,-880.21,-1026.9,-1173.6,-1320.3,-1467,-1613.7,-1760.4,-1907.1,-2053.8,-2200.5,-2347.2,-2493.9,-2640.6,-2787.3,-2934,-3080.7,-3227.4,-3374.1,-3520.8,-3667.5,-3814.2,-3960.9,-4107.6,-4254.3,-4401,-4547.7,-4694.5,-4841.2,-4987.9,-5134.6,-5281.3,-5428,-5574.7,-5721.4,-5868.1,-6014.8,-6161.5,-6308.2,-6454.9,-6601.6,-6748.3,-6895,-7041.7,-7188.4,-7335.1
      | -0,-123.75,-247.49,-371.24,-494.99,-618.73,-742.48,-866.23,-989.98,-1113.7,-1237.5,-1361.2,-1485,-1608.7,-1732.5,-1856.2,-1980,-2103.7,-2227.4,-2351.2,-2474.9,-2598.7,-2722.4,-2846.2,-2969.9,-3093.7,-3217.4,-3341.2,-3464.9,-3588.7,-3712.4,-3836.2,-3959.9,-4083.7,-4207.4,-4331.1,-4454.9,-4578.6,-4702.4,-4826.1,-4949.9,-5073.6,-5197.4,-5321.1,-5444.9,-5568.6,-5692.4,-5816.1,-5939.9,-6063.6,-6187.3
      | -0,-101.91,-203.81,-305.72,-407.63,-509.53,-611.44,-713.35,-815.25,-917.16,-1019.1,-1121,-1222.9,-1324.8,-1426.7,-1528.6,-1630.5,-1732.4,-1834.3,-1936.2,-2038.1,-2140,-2241.9,-2343.9,-2445.8,-2547.7,-2649.6,-2751.5,-2853.4,-2955.3,-3057.2,-3159.1,-3261,-3362.9,-3464.8,-3566.7,-3668.6,-3770.5,-3872.5,-3974.4,-4076.3,-4178.2,-4280.1,-4382,-4483.9,-4585.8,-4687.7,-4789.6,-4891.5,-4993.4,-5095.3
      | -0,-82.514,-165.03,-247.54,-330.06,-412.57,-495.09,-577.6,-660.12,-742.63,-825.14,-907.66,-990.17,-1072.7,-1155.2,-1237.7,-1320.2,-1402.7,-1485.3,-1567.8,-1650.3,-1732.8,-1815.3,-1897.8,-1980.3,-2062.9,-2145.4,-2227.9,-2310.4,-2392.9,-2475.4,-2557.9,-2640.5,-2723,-2805.5,-2888,-2970.5,-3053,-3135.6,-3218.1,-3300.6,-3383.1,-3465.6,-3548.1,-3630.6,-3713.2,-3795.7,-3878.2,-3960.7,-4043.2,-4125.7
      | -0,-66.058,-132.12,-198.17,-264.23,-330.29,-396.35,-462.41,-528.46,-594.52,-660.58,-726.64,-792.7,-858.76,-924.81,-990.87,-1056.9,-1123,-1189,-1255.1,-1321.2,-1387.2,-1453.3,-1519.3,-1585.4,-1651.5,-1717.5,-1783.6,-1849.6,-1915.7,-1981.7,-2047.8,-2113.9,-2179.9,-2246,-2312,-2378.1,-2444.2,-2510.2,-2576.3,-2642.3,-2708.4,-2774.4,-2840.5,-2906.6,-2972.6,-3038.7,-3104.7,-3170.8,-3236.8,-3302.9
      | -0,-52.494,-104.99,-157.48,-209.98,-262.47,-314.97,-367.46,-419.95,-472.45,-524.94,-577.44,-629.93,-682.43,-734.92,-787.41,-839.91,-892.4,-944.9,-997.39,-1049.9,-1102.4,-1154.9,-1207.4,-1259.9,-1312.4,-1364.9,-1417.3,-1469.8,-1522.3,-1574.8,-1627.3,-1679.8,-1732.3,-1784.8,-1837.3,-1889.8,-1942.3,-1994.8,-2047.3,-2099.8,-2152.3,-2204.8,-2257.3,-2309.7,-2362.2,-2414.7,-2467.2,-2519.7,-2572.2,-2624.7
      | -0,-41.519,-83.039,-124.56,-166.08,-207.6,-249.12,-290.64,-332.15,-373.67,-415.19,-456.71,-498.23,-539.75,-581.27,-622.79,-664.31,-705.83,-747.35,-788.87,-830.39,-871.91,-913.42,-954.94,-996.46,-1038,-1079.5,-1121,-1162.5,-1204.1,-1245.6,-1287.1,-1328.6,-1370.1,-1411.7,-1453.2,-1494.7,-1536.2,-1577.7,-1619.3,-1660.8,-1702.3,-1743.8,-1785.3,-1826.8,-1868.4,-1909.9,-1951.4,-1992.9,-2034.4,-2076
      | -0,-32.742,-65.483,-98.225,-130.97,-163.71,-196.45,-229.19,-261.93,-294.67,-327.42,-360.16,-392.9,-425.64,-458.38,-491.12,-523.86,-556.61,-589.35,-622.09,-654.83,-687.57,-720.31,-753.06,-785.8,-818.54,-851.28,-884.02,-916.76,-949.5,-982.25,-1015,-1047.7,-1080.5,-1113.2,-1146,-1178.7,-1211.4,-1244.2,-1276.9,-1309.7,-1342.4,-1375.1,-1407.9,-1440.6,-1473.4,-1506.1,-1538.9,-1571.6,-1604.3,-1637.1
      | 0,32.742,65.483,98.225,130.97,163.71,196.45,229.19,261.93,294.67,327.42,360.16,392.9,425.64,458.38,491.12,523.86,556.61,589.35,622.09,654.83,687.57,720.31,753.06,785.8,818.54,851.28,884.02,916.76,949.5,982.25,1015,1047.7,1080.5,1113.2,1146,1178.7,1211.4,1244.2,1276.9,1309.7,1342.4,1375.1,1407.9,1440.6,1473.4,1506.1,1538.9,1571.6,1604.3,1637.1
      | 0,41.519,83.039,124.56,166.08,207.6,249.12,290.64,332.15,373.67,415.19,456.71,498.23,539.75,581.27,622.79,664.31,705.83,747.35,788.87,830.39,871.91,913.42,954.94,996.46,1038,1079.5,1121,1162.5,1204.1,1245.6,1287.1,1328.6,1370.1,1411.7,1453.2,1494.7,1536.2,1577.7,1619.3,1660.8,1702.3,1743.8,1785.3,1826.8,1868.4,1909.9,1951.4,1992.9,2034.4,2076
      | 0,52.494,104.99,157.48,209.98,262.47,314.97,367.46,419.95,472.45,524.94,577.44,629.93,682.43,734.92,787.41,839.91,892.4,944.9,997.39,1049.9,1102.4,1154.9,1207.4,1259.9,1312.4,1364.9,1417.3,1469.8,1522.3,1574.8,1627.3,1679.8,1732.3,1784.8,1837.3,1889.8,1942.3,1994.8,2047.3,2099.8,2152.3,2204.8,2257.3,2309.7,2362.2,2414.7,2467.2,2519.7,2572.2,2624.7
      | 0,66.058,132.12,198.17,264.23,330.29,396.35,462.41,528.46,594.52,660.58,726.64,792.7,858.76,924.81,990.87,1056.9,1123,1189,1255.1,1321.2,1387.2,1453.3,1519.3,1585.4,1651.5,1717.5,1783.6,1849.6,1915.7,1981.7,2047.8,2113.9,2179.9,2246,2312,2378.1,2444.2,2510.2,2576.3,2642.3,2708.4,2774.4,2840.5,2906.6,2972.6,3038.7,3104.7,3170.8,3236.8,3302.9
      | 0,82.514,165.03,247.54,330.06,412.57,495.09,577.6,660.12,742.63,825.14,907.66,990.17,1072.7,1155.2,1237.7,1320.2,1402.7,1485.3,1567.8,1650.3,1732.8,1815.3,1897.8,1980.3,2062.9,2145.4,2227.9,2310.4,2392.9,2475.4,2557.9,2640.5,2723,2805.5,2888,2970.5,3053,3135.6,3218.1,3300.6,3383.1,3465.6,3548.1,3630.6,3713.2,3795.7,3878.2,3960.7,4043.2,4125.7
      | 0,101.91,203.81,305.72,407.63,509.53,611.44,713.35,815.25,917.16,1019.1,1121,1222.9,1324.8,1426.7,1528.6,1630.5,1732.4,1834.3,1936.2,2038.1,2140,2241.9,2343.9,2445.8,2547.7,2649.6,2751.5,2853.4,2955.3,3057.2,3159.1,3261,3362.9,3464.8,3566.7,3668.6,3770.5,3872.5,3974.4,4076.3,4178.2,4280.1,4382,4483.9,4585.8,4687.7,4789.6,4891.5,4993.4,5095.3
      | 0,123.75,247.49,371.24,494.99,618.73,742.48,866.23,989.98,1113.7,1237.5,1361.2,1485,1608.7,1732.5,1856.2,1980,2103.7,2227.4,2351.2,2474.9,2598.7,2722.4,2846.2,2969.9,3093.7,3217.4,3341.2,3464.9,3588.7,3712.4,3836.2,3959.9,4083.7,4207.4,4331.1,4454.9,4578.6,4702.4,4826.1,4949.9,5073.6,5197.4,5321.1,5444.9,5568.6,5692.4,5816.1,5939.9,6063.6,6187.3
      | 0,146.7,293.4,440.1,586.81,733.51,880.21,1026.9,1173.6,1320.3,1467,1613.7,1760.4,1907.1,2053.8,2200.5,2347.2,2493.9,2640.6,2787.3,2934,3080.7,3227.4,3374.1,3520.8,3667.5,3814.2,3960.9,4107.6,4254.3,4401,4547.7,4694.5,4841.2,4987.9,5134.6,5281.3,5428,5574.7,5721.4,5868.1,6014.8,6161.5,6308.2,6454.9,6601.6,6748.3,6895,7041.7,7188.4,7335.1
      | 0,168.44,336.89,505.33,673.78,842.22,1010.7,1179.1,1347.6,1516,1684.4,1852.9,2021.3,2189.8,2358.2,2526.7,2695.1,2863.5,3032,3200.4,3368.9,3537.3,3705.8,3874.2,4042.7,4211.1,4379.5,4548,4716.4,4884.9,5053.3,5221.8,5390.2,5558.6,5727.1,5895.5,6064,6232.4,6400.9,6569.3,6737.8,6906.2,7074.6,7243.1,7411.5,7580,7748.4,7916.9,8085.3,8253.7,8422.2
      | 0,186.02,372.04,558.06,744.08,930.1,1116.1,1302.1,1488.2,1674.2,1860.2,2046.2,2232.2,2418.3,2604.3,2790.3,2976.3,3162.3,3348.4,3534.4,3720.4,3906.4,4092.4,4278.5,4464.5,4650.5,4836.5,5022.5,5208.6,5394.6,5580.6,5766.6,5952.6,6138.7,6324.7,6510.7,6696.7,6882.7,7068.7,7254.8,7440.8,7626.8,7812.8,7998.8,8184.9,8370.9,8556.9,8742.9,8928.9,9115,9301
      | 0,196.87,393.74,590.6,787.47,984.34,1181.2,1378.1,1574.9,1771.8,1968.7,2165.5,2362.4,2559.3,2756.2,2953,3149.9,3346.8,3543.6,3740.5,3937.4,4134.2,4331.1,4528,4724.8,4921.7,5118.6,5315.4,5512.3,5709.2,5906,6102.9,6299.8,6496.6,6693.5,6890.4,7087.2,7284.1,7481,7677.8,7874.7,8071.6,8268.5,8465.3,8662.2,8859.1,9055.9,9252.8,9449.7,9646.5,9843.4
      | 0,199.97,399.95,599.92,799.9,999.87,1199.8,1399.8,1599.8,1799.8,1999.7,2199.7,2399.7,2599.7,2799.6,2999.6,3199.6,3399.6,3599.5,3799.5,3999.5,4199.5,4399.4,4599.4,4799.4,4999.4,5199.3,5399.3,5599.3,5799.2,5999.2,6199.2,6399.2,6599.1,6799.1,6999.1,7199.1,7399,7599,7799,7999,8198.9,8398.9,8598.9,8798.9,8998.8,9198.8,9398.8,9598.8,9798.7,9998.7
      | 0,196.25,392.49,588.74,784.98,981.23,1177.5,1373.7,1570,1766.2,1962.5,2158.7,2354.9,2551.2,2747.4,2943.7,3139.9,3336.2,3532.4,3728.7,3924.9,4121.2,4317.4,4513.6,4709.9,4906.1,5102.4,5298.6,5494.9,5691.1,5887.4,6083.6,6279.9,6476.1,6672.3,6868.6,7064.8,7261.1,7457.3,7653.6,7849.8,8046.1,8242.3,8438.6,8634.8,8831,9027.3,9223.5,9419.8,9616,9812.3
      | 0,187.84,375.67,563.51,751.35,939.18,1127,1314.9,1502.7,1690.5,1878.4,2066.2,2254,2441.9,2629.7,2817.5,3005.4,3193.2,3381.1,3568.9,3756.7,3944.6,4132.4,4320.2,4508.1,4695.9,4883.7,5071.6,5259.4,5447.3,5635.1,5822.9,6010.8,6198.6,6386.4,6574.3,6762.1,6949.9,7137.8,7325.6,7513.5,7701.3,7889.1,8077,8264.8,8452.6,8640.5,8828.3,9016.1,9204,9391.8
      | 0,177.09,354.19,531.28,708.38,885.47,1062.6,1239.7,1416.8,1593.8,1770.9,1948,2125.1,2302.2,2479.3,2656.4,2833.5,3010.6,3187.7,3364.8,3541.9,3719,3896.1,4073.2,4250.3,4427.4,4604.5,4781.5,4958.6,5135.7,5312.8,5489.9,5667,5844.1,6021.2,6198.3,6375.4,6552.5,6729.6,6906.7,7083.8,7260.9,7438,7615.1,7792.1,7969.2,8146.3,8323.4,8500.5,8677.6,8854.7
      | 0,165.86,331.71,497.57,663.43,829.28,995.14,1161,1326.9,1492.7,1658.6,1824.4,1990.3,2156.1,2322,2487.8,2653.7,2819.6,2985.4,3151.3,3317.1,3483,3648.8,3814.7,3980.6,4146.4,4312.3,4478.1,4644,4809.8,4975.7,5141.5,5307.4,5473.3,5639.1,5805,5970.8,6136.7,6302.5,6468.4,6634.3,6800.1,6966,7131.8,7297.7,7463.5,7629.4,7795.2,7961.1,8127,8292.8
      | 0,155.26,310.53,465.79,621.05,776.32,931.58,1086.8,1242.1,1397.4,1552.6,1707.9,1863.2,2018.4,2173.7,2328.9,2484.2,2639.5,2794.7,2950,3105.3,3260.5,3415.8,3571.1,3726.3,3881.6,4036.8,4192.1,4347.4,4502.6,4657.9,4813.2,4968.4,5123.7,5278.9,5434.2,5589.5,5744.7,5900,6055.3,6210.5,6365.8,6521.1,6676.3,6831.6,6986.8,7142.1,7297.4,7452.6,7607.9,7763.2
      | 0,145.88,291.75,437.63,583.5,729.38,875.25,1021.1,1167,1312.9,1458.8,1604.6,1750.5,1896.4,2042.3,2188.1,2334,2479.9,2625.8,2771.6,2917.5,3063.4,3209.3,3355.1,3501,3646.9,3792.8,3938.6,4084.5,4230.4,4376.3,4522.1,4668,4813.9,4959.8,5105.6,5251.5,5397.4,5543.3,5689.1,5835,5980.9,6126.8,6272.6,6418.5,6564.4,6710.3,6856.1,7002,7147.9,7293.8
      | 0,137.87,275.75,413.62,551.49,689.36,827.24,965.11,1103,1240.9,1378.7,1516.6,1654.5,1792.3,1930.2,2068.1,2206,2343.8,2481.7,2619.6,2757.5,2895.3,3033.2,3171.1,3308.9,3446.8,3584.7,3722.6,3860.4,3998.3,4136.2,4274,4411.9,4549.8,4687.7,4825.5,4963.4,5101.3,5239.2,5377,5514.9,5652.8,5790.6,5928.5,6066.4,6204.3,6342.1,6480,6617.9,6755.8,6893.6
      | 0,131.22,262.44,393.66,524.88,656.1,787.32,918.54,1049.8,1181,1312.2,1443.4,1574.6,1705.9,1837.1,1968.3,2099.5,2230.7,2362,2493.2,2624.4,2755.6,2886.8,3018.1,3149.3,3280.5,3411.7,3542.9,3674.2,3805.4,3936.6,4067.8,4199,4330.2,4461.5,4592.7,4723.9,4855.1,4986.3,5117.6,5248.8,5380,5511.2,5642.4,5773.7,5904.9,6036.1,6167.3,6298.5,6429.8,6561]
      MyMap=|
      | [0,1114.7,4367.1,9707.2,17109,26554,38030,51524,67028,84533,1.0403e+05,1.2552e+05,1.4899e+05,1.7444e+05,2.0185e+05,2.3124e+05,2.6259e+05,2.959e+05,3.3117e+05,3.6839e+05,4.0756e+05,4.4868e+05,4.9174e+05,5.3675e+05,5.8369e+05,6.3257e+05,6.8338e+05,7.3613e+05,7.908e+05,8.474e+05,9.0593e+05,9.6638e+05,1.0288e+06,1.093e+06,1.1593e+06,1.2274e+06,1.2974e+06,1.3694e+06,1.4432e+06,1.519e+06,1.5967e+06,1.6763e+06,1.7578e+06,1.8412e+06,1.9265e+06,2.0137e+06,2.1028e+06,2.1938e+06,2.2867e+06,2.3815e+06,2.4782e+06
      | 0,1024.5,4013.8,8921.9,15725,24406,34953,47356,61605,77694,95616,1.1537e+05,1.3694e+05,1.6032e+05,1.8553e+05,2.1254e+05,2.4135e+05,2.7197e+05,3.0438e+05,3.3859e+05,3.7459e+05,4.1238e+05,4.5196e+05,4.9333e+05,5.3647e+05,5.814e+05,6.281e+05,6.7658e+05,7.2683e+05,7.7885e+05,8.3264e+05,8.8821e+05,9.4553e+05,1.0046e+06,1.0655e+06,1.1281e+06,1.1925e+06,1.2586e+06,1.3265e+06,1.3961e+06,1.4675e+06,1.5407e+06,1.6156e+06,1.6922e+06,1.7706e+06,1.8508e+06,1.9327e+06,2.0163e+06,2.1017e+06,2.1889e+06,2.2777e+06
      | 0,938.57,3677,8173.3,14405,22358,32020,43382,56436,71175,87593,1.0568e+05,1.2545e+05,1.4687e+05,1.6996e+05,1.947e+05,2.211e+05,2.4915e+05,2.7884e+05,3.1018e+05,3.4316e+05,3.7778e+05,4.1404e+05,4.5193e+05,4.9146e+05,5.3261e+05,5.754e+05,6.1981e+05,6.6584e+05,7.135e+05,7.6278e+05,8.1368e+05,8.6619e+05,9.2032e+05,9.7607e+05,1.0334e+06,1.0924e+06,1.153e+06,1.2152e+06,1.279e+06,1.3444e+06,1.4114e+06,1.48e+06,1.5502e+06,1.6221e+06,1.6955e+06,1.7705e+06,1.8471e+06,1.9254e+06,2.0052e+06,2.0866e+06
      | 0,856.81,3356.7,7461.3,13151,20411,29231,39603,51520,64974,79962,96478,1.1452e+05,1.3408e+05,1.5515e+05,1.7774e+05,2.0184e+05,2.2744e+05,2.5455e+05,2.8316e+05,3.1327e+05,3.4487e+05,3.7797e+05,4.1256e+05,4.4864e+05,4.8621e+05,5.2527e+05,5.6581e+05,6.0784e+05,6.5134e+05,6.9633e+05,7.4279e+05,7.9073e+05,8.4015e+05,8.9104e+05,9.4341e+05,9.9724e+05,1.0525e+06,1.1093e+06,1.1676e+06,1.2273e+06,1.2885e+06,1.3511e+06,1.4152e+06,1.4808e+06,1.5478e+06,1.6163e+06,1.6862e+06,1.7576e+06,1.8305e+06,1.9048e+06
      | 0,779.25,3052.9,6785.9,11960,18563,26585,36018,46856,59093,72724,87745,1.0415e+05,1.2194e+05,1.4111e+05,1.6165e+05,1.8357e+05,2.0685e+05,2.3151e+05,2.5753e+05,2.8491e+05,3.1365e+05,3.4376e+05,3.7522e+05,4.0803e+05,4.422e+05,4.7772e+05,5.1459e+05,5.5282e+05,5.9238e+05,6.333e+05,6.7556e+05,7.1916e+05,7.641e+05,8.1039e+05,8.5801e+05,9.0697e+05,9.5727e+05,1.0089e+06,1.0619e+06,1.1162e+06,1.1718e+06,1.2288e+06,1.2871e+06,1.3467e+06,1.4077e+06,1.47e+06,1.5336e+06,1.5985e+06,1.6648e+06,1.7324e+06
      | 0,705.9,2765.5,6147.1,10834,16816,24083,32628,42446,53531,65879,79486,94348,1.1046e+05,1.2783e+05,1.4643e+05,1.6629e+05,1.8738e+05,2.0972e+05,2.3329e+05,2.5809e+05,2.8413e+05,3.114e+05,3.399e+05,3.6962e+05,4.0058e+05,4.3276e+05,4.6616e+05,5.0078e+05,5.3662e+05,5.7369e+05,6.1197e+05,6.5146e+05,6.9218e+05,7.3411e+05,7.7725e+05,8.216e+05,8.6717e+05,9.1394e+05,9.6193e+05,1.0111e+06,1.0615e+06,1.1131e+06,1.1659e+06,1.22e+06,1.2752e+06,1.3316e+06,1.3892e+06,1.4481e+06,1.5081e+06,1.5693e+06
      | 0,636.76,2494.6,5545,9773.1,15169,21724,29432,38288,48287,59426,71700,85106,99642,1.153e+05,1.3209e+05,1.5e+05,1.6903e+05,1.8917e+05,2.1044e+05,2.3281e+05,2.563e+05,2.809e+05,3.066e+05,3.3342e+05,3.6134e+05,3.9037e+05,4.205e+05,4.5173e+05,4.8406e+05,5.1749e+05,5.5202e+05,5.8765e+05,6.2438e+05,6.622e+05,7.0111e+05,7.4112e+05,7.8223e+05,8.2442e+05,8.677e+05,9.1208e+05,9.5754e+05,1.0041e+06,1.0517e+06,1.1005e+06,1.1503e+06,1.2012e+06,1.2532e+06,1.3062e+06,1.3604e+06,1.4156e+06
      | 0,571.82,2240.2,4979.5,8776.4,13622,19508,26430,34383,43363,53365,64388,76427,89480,1.0355e+05,1.1862e+05,1.347e+05,1.5179e+05,1.6988e+05,1.8897e+05,2.0907e+05,2.3016e+05,2.5225e+05,2.7534e+05,2.9942e+05,3.2449e+05,3.5056e+05,3.7761e+05,4.0566e+05,4.3469e+05,4.6472e+05,4.9573e+05,5.2772e+05,5.607e+05,5.9467e+05,6.2961e+05,6.6554e+05,7.0245e+05,7.4034e+05,7.7921e+05,8.1906e+05,8.5989e+05,9.017e+05,9.4448e+05,9.8824e+05,1.033e+06,1.0787e+06,1.1254e+06,1.173e+06,1.2216e+06,1.2712e+06
      | 0,511.09,2002.3,4450.7,7844.3,12175,17436,23623,30732,38757,47698,57549,68310,79977,92548,1.0602e+05,1.204e+05,1.3567e+05,1.5184e+05,1.689e+05,1.8686e+05,2.0572e+05,2.2546e+05,2.4609e+05,2.6762e+05,2.9003e+05,3.1332e+05,3.3751e+05,3.6258e+05,3.8853e+05,4.1536e+05,4.4308e+05,4.7167e+05,5.0115e+05,5.3151e+05,5.6274e+05,5.9486e+05,6.2785e+05,6.6171e+05,6.9646e+05,7.3207e+05,7.6857e+05,8.0593e+05,8.4417e+05,8.8328e+05,9.2326e+05,9.6412e+05,1.0058e+06,1.0484e+06,1.0919e+06,1.1362e+06
      | 0,454.56,1780.8,3958.4,6976.8,10828,15508,21011,27333,34471,42422,51185,60755,71132,82313,94296,1.0708e+05,1.2066e+05,1.3505e+05,1.5022e+05,1.662e+05,1.8296e+05,2.0052e+05,2.1888e+05,2.3802e+05,2.5795e+05,2.7867e+05,3.0018e+05,3.2248e+05,3.4556e+05,3.6942e+05,3.9407e+05,4.1951e+05,4.4573e+05,4.7273e+05,5.0051e+05,5.2907e+05,5.5841e+05,5.8853e+05,6.1943e+05,6.5111e+05,6.8356e+05,7.168e+05,7.5081e+05,7.8559e+05,8.2115e+05,8.5749e+05,8.946e+05,9.3248e+05,9.7114e+05,1.0106e+06
      | 0,402.25,1575.9,3502.8,6173.8,9582.1,13723,18592,24187,30503,37540,45293,53762,62945,72839,83443,94756,1.0678e+05,1.195e+05,1.3293e+05,1.4707e+05,1.6191e+05,1.7745e+05,1.9368e+05,2.1062e+05,2.2826e+05,2.466e+05,2.6563e+05,2.8536e+05,3.0578e+05,3.269e+05,3.4872e+05,3.7123e+05,3.9442e+05,4.1832e+05,4.429e+05,4.6817e+05,4.9414e+05,5.2079e+05,5.4814e+05,5.7617e+05,6.0489e+05,6.343e+05,6.6439e+05,6.9517e+05,7.2664e+05,7.588e+05,7.9163e+05,8.2516e+05,8.5937e+05,8.9426e+05
      | 0,354.13,1387.4,3083.9,5435.3,8436,12082,16369,21294,26855,33050,39876,47332,55416,64127,73463,83423,94005,1.0521e+05,1.1703e+05,1.2948e+05,1.4254e+05,1.5622e+05,1.7052e+05,1.8543e+05,2.0096e+05,2.171e+05,2.3386e+05,2.5123e+05,2.6921e+05,2.878e+05,3.0701e+05,3.2682e+05,3.4725e+05,3.6828e+05,3.8993e+05,4.1218e+05,4.3504e+05,4.585e+05,4.8258e+05,5.0725e+05,5.3254e+05,5.5843e+05,5.8493e+05,6.1203e+05,6.3973e+05,6.6804e+05,6.9695e+05,7.2646e+05,7.5658e+05,7.873e+05
      | 0,310.23,1215.4,2701.5,4761.5,7390.2,10584,14339,18654,23526,28952,34932,41464,48546,56176,64355,73080,82351,92166,1.0252e+05,1.1343e+05,1.2487e+05,1.3685e+05,1.4938e+05,1.6244e+05,1.7605e+05,1.9019e+05,2.0487e+05,2.2008e+05,2.3583e+05,2.5212e+05,2.6895e+05,2.863e+05,3.042e+05,3.2262e+05,3.4158e+05,3.6108e+05,3.811e+05,4.0166e+05,4.2275e+05,4.4437e+05,4.6652e+05,4.892e+05,5.1241e+05,5.3615e+05,5.6042e+05,5.8521e+05,6.1054e+05,6.364e+05,6.6278e+05,6.8969e+05
      | 0,270.53,1059.9,2355.8,4152.2,6444.5,9229.4,12504,16267,20515,25247,30462,36158,42334,48988,56120,63728,71813,80372,89405,98911,1.0889e+05,1.1934e+05,1.3026e+05,1.4166e+05,1.5352e+05,1.6585e+05,1.7865e+05,1.9192e+05,2.0566e+05,2.1986e+05,2.3453e+05,2.4967e+05,2.6527e+05,2.8134e+05,2.9787e+05,3.1487e+05,3.3233e+05,3.5026e+05,3.6865e+05,3.875e+05,4.0682e+05,4.266e+05,4.4684e+05,4.6754e+05,4.887e+05,5.1033e+05,5.3241e+05,5.5496e+05,5.7797e+05,6.0143e+05
      | 0,235.04,920.8,2046.8,3607.4,5599,8018.6,10864,14133,17824,21935,26466,31414,36780,42561,48757,55367,62391,69827,77675,85934,94604,1.0368e+05,1.1317e+05,1.2307e+05,1.3338e+05,1.4409e+05,1.5521e+05,1.6674e+05,1.7867e+05,1.9101e+05,2.0376e+05,2.1691e+05,2.3047e+05,2.4443e+05,2.5879e+05,2.7356e+05,2.8873e+05,3.0431e+05,3.2028e+05,3.3666e+05,3.5345e+05,3.7063e+05,3.8821e+05,4.062e+05,4.2459e+05,4.4337e+05,4.6256e+05,4.8215e+05,5.0214e+05,5.2253e+05
      | 0,203.75,798.24,1774.3,3127.2,4853.7,6951.2,9417.7,12252,15451,19015,22943,27233,31884,36896,42267,47997,54086,60533,67336,74496,82011,89882,98108,1.0669e+05,1.1562e+05,1.2491e+05,1.3455e+05,1.4455e+05,1.5489e+05,1.6559e+05,1.7664e+05,1.8804e+05,1.9979e+05,2.1189e+05,2.2434e+05,2.3715e+05,2.503e+05,2.638e+05,2.7765e+05,2.9185e+05,3.064e+05,3.2129e+05,3.3654e+05,3.5213e+05,3.6807e+05,3.8436e+05,4.0099e+05,4.1797e+05,4.353e+05,4.5297e+05
      | 0,176.67,692.15,1538.5,2711.6,4208.6,6027.4,8166.1,10623,13398,16488,19894,23613,27646,31992,36650,41618,46898,52488,58387,64595,71112,77937,85069,92509,1.0026e+05,1.0831e+05,1.1667e+05,1.2533e+05,1.3431e+05,1.4358e+05,1.5316e+05,1.6305e+05,1.7324e+05,1.8373e+05,1.9453e+05,2.0563e+05,2.1703e+05,2.2874e+05,2.4075e+05,2.5306e+05,2.6568e+05,2.7859e+05,2.9181e+05,3.0533e+05,3.1915e+05,3.3327e+05,3.477e+05,3.6242e+05,3.7745e+05,3.9277e+05
      | 0,153.8,602.54,1339.3,2360.6,3663.8,5247,7108.9,9247.9,11663,14353,17318,20556,24067,27850,31905,36230,40826,45692,50828,56232,61905,67847,74056,80533,87277,94287,1.0156e+05,1.0911e+05,1.1692e+05,1.2499e+05,1.3333e+05,1.4194e+05,1.5081e+05,1.5994e+05,1.6934e+05,1.7901e+05,1.8894e+05,1.9913e+05,2.0958e+05,2.203e+05,2.3128e+05,2.4253e+05,2.5403e+05,2.658e+05,2.7783e+05,2.9013e+05,3.0268e+05,3.155e+05,3.2858e+05,3.4192e+05
      | 0,135.13,529.41,1176.8,2074.1,3219.1,4610.2,6246.1,8125.5,10248,12611,15216,18061,21146,24470,28033,31833,35871,40147,44659,49407,54392,59612,65068,70759,76684,82844,89238,95866,1.0273e+05,1.0982e+05,1.1715e+05,1.2471e+05,1.3251e+05,1.4053e+05,1.4879e+05,1.5728e+05,1.66e+05,1.7496e+05,1.8415e+05,1.9356e+05,2.0321e+05,2.1309e+05,2.232e+05,2.3354e+05,2.4411e+05,2.5492e+05,2.6595e+05,2.7721e+05,2.887e+05,3.0042e+05
      | 0,120.67,472.76,1050.9,1852.1,2874.6,4116.9,5577.7,7256.1,9151,11262,13588,16129,18883,21852,25033,28427,32033,35851,39880,44121,48572,53234,58105,63187,68479,73979,79689,85608,91735,98071,1.0462e+05,1.1137e+05,1.1833e+05,1.255e+05,1.3287e+05,1.4045e+05,1.4824e+05,1.5624e+05,1.6444e+05,1.7285e+05,1.8147e+05,1.9029e+05,1.9932e+05,2.0855e+05,2.1799e+05,2.2764e+05,2.3749e+05,2.4755e+05,2.5781e+05,2.6828e+05
      | 0,110.42,432.59,961.56,1694.8,2630.4,3767.1,5103.8,6639.5,8373.5,10305,12433,14758,17279,19995,22906,26012,29311,32805,36492,40372,44445,48710,53168,57818,62660,67694,72918,78334,83941,89738,95727,1.019e+05,1.0827e+05,1.1483e+05,1.2158e+05,1.2852e+05,1.3565e+05,1.4296e+05,1.5047e+05,1.5816e+05,1.6605e+05,1.7412e+05,1.8238e+05,1.9083e+05,1.9947e+05,2.083e+05,2.1731e+05,2.2651e+05,2.359e+05,2.4548e+05
      | 0,120.67,472.76,1050.9,1852.1,2874.6,4116.9,5577.7,7256.1,9151,11262,13588,16129,18883,21852,25033,28427,32033,35851,39880,44121,48572,53234,58105,63187,68479,73979,79689,85608,91735,98071,1.0462e+05,1.1137e+05,1.1833e+05,1.255e+05,1.3287e+05,1.4045e+05,1.4824e+05,1.5624e+05,1.6444e+05,1.7285e+05,1.8147e+05,1.9029e+05,1.9932e+05,2.0855e+05,2.1799e+05,2.2764e+05,2.3749e+05,2.4755e+05,2.5781e+05,2.6828e+05
      | 0,135.13,529.41,1176.8,2074.1,3219.1,4610.2,6246.1,8125.5,10248,12611,15216,18061,21146,24470,28033,31833,35871,40147,44659,49407,54392,59612,65068,70759,76684,82844,89238,95866,1.0273e+05,1.0982e+05,1.1715e+05,1.2471e+05,1.3251e+05,1.4053e+05,1.4879e+05,1.5728e+05,1.66e+05,1.7496e+05,1.8415e+05,1.9356e+05,2.0321e+05,2.1309e+05,2.232e+05,2.3354e+05,2.4411e+05,2.5492e+05,2.6595e+05,2.7721e+05,2.887e+05,3.0042e+05
      | 0,153.8,602.54,1339.3,2360.6,3663.8,5247,7108.9,9247.9,11663,14353,17318,20556,24067,27850,31905,36230,40826,45692,50828,56232,61905,67847,74056,80533,87277,94287,1.0156e+05,1.0911e+05,1.1692e+05,1.2499e+05,1.3333e+05,1.4194e+05,1.5081e+05,1.5994e+05,1.6934e+05,1.7901e+05,1.8894e+05,1.9913e+05,2.0958e+05,2.203e+05,2.3128e+05,2.4253e+05,2.5403e+05,2.658e+05,2.7783e+05,2.9013e+05,3.0268e+05,3.155e+05,3.2858e+05,3.4192e+05
      | 0,176.67,692.15,1538.5,2711.6,4208.6,6027.4,8166.1,10623,13398,16488,19894,23613,27646,31992,36650,41618,46898,52488,58387,64595,71112,77937,85069,92509,1.0026e+05,1.0831e+05,1.1667e+05,1.2533e+05,1.3431e+05,1.4358e+05,1.5316e+05,1.6305e+05,1.7324e+05,1.8373e+05,1.9453e+05,2.0563e+05,2.1703e+05,2.2874e+05,2.4075e+05,2.5306e+05,2.6568e+05,2.7859e+05,2.9181e+05,3.0533e+05,3.1915e+05,3.3327e+05,3.477e+05,3.6242e+05,3.7745e+05,3.9277e+05
      | 0,203.75,798.24,1774.3,3127.2,4853.7,6951.2,9417.7,12252,15451,19015,22943,27233,31884,36896,42267,47997,54086,60533,67336,74496,82011,89882,98108,1.0669e+05,1.1562e+05,1.2491e+05,1.3455e+05,1.4455e+05,1.5489e+05,1.6559e+05,1.7664e+05,1.8804e+05,1.9979e+05,2.1189e+05,2.2434e+05,2.3715e+05,2.503e+05,2.638e+05,2.7765e+05,2.9185e+05,3.064e+05,3.2129e+05,3.3654e+05,3.5213e+05,3.6807e+05,3.8436e+05,4.0099e+05,4.1797e+05,4.353e+05,4.5297e+05
      | 0,235.04,920.8,2046.8,3607.4,5599,8018.6,10864,14133,17824,21935,26466,31414,36780,42561,48757,55367,62391,69827,77675,85934,94604,1.0368e+05,1.1317e+05,1.2307e+05,1.3338e+05,1.4409e+05,1.5521e+05,1.6674e+05,1.7867e+05,1.9101e+05,2.0376e+05,2.1691e+05,2.3047e+05,2.4443e+05,2.5879e+05,2.7356e+05,2.8873e+05,3.0431e+05,3.2028e+05,3.3666e+05,3.5345e+05,3.7063e+05,3.8821e+05,4.062e+05,4.2459e+05,4.4337e+05,4.6256e+05,4.8215e+05,5.0214e+05,5.2253e+05
      | 0,270.53,1059.9,2355.8,4152.2,6444.5,9229.4,12504,16267,20515,25247,30462,36158,42334,48988,56120,63728,71813,80372,89405,98911,1.0889e+05,1.1934e+05,1.3026e+05,1.4166e+05,1.5352e+05,1.6585e+05,1.7865e+05,1.9192e+05,2.0566e+05,2.1986e+05,2.3453e+05,2.4967e+05,2.6527e+05,2.8134e+05,2.9787e+05,3.1487e+05,3.3233e+05,3.5026e+05,3.6865e+05,3.875e+05,4.0682e+05,4.266e+05,4.4684e+05,4.6754e+05,4.887e+05,5.1033e+05,5.3241e+05,5.5496e+05,5.7797e+05,6.0143e+05
      | 0,310.23,1215.4,2701.5,4761.5,7390.2,10584,14339,18654,23526,28952,34932,41464,48546,56176,64355,73080,82351,92166,1.0252e+05,1.1343e+05,1.2487e+05,1.3685e+05,1.4938e+05,1.6244e+05,1.7605e+05,1.9019e+05,2.0487e+05,2.2008e+05,2.3583e+05,2.5212e+05,2.6895e+05,2.863e+05,3.042e+05,3.2262e+05,3.4158e+05,3.6108e+05,3.811e+05,4.0166e+05,4.2275e+05,4.4437e+05,4.6652e+05,4.892e+05,5.1241e+05,5.3615e+05,5.6042e+05,5.8521e+05,6.1054e+05,6.364e+05,6.6278e+05,6.8969e+05
      | 0,354.13,1387.4,3083.9,5435.3,8436,12082,16369,21294,26855,33050,39876,47332,55416,64127,73463,83423,94005,1.0521e+05,1.1703e+05,1.2948e+05,1.4254e+05,1.5622e+05,1.7052e+05,1.8543e+05,2.0096e+05,2.171e+05,2.3386e+05,2.5123e+05,2.6921e+05,2.878e+05,3.0701e+05,3.2682e+05,3.4725e+05,3.6828e+05,3.8993e+05,4.1218e+05,4.3504e+05,4.585e+05,4.8258e+05,5.0725e+05,5.3254e+05,5.5843e+05,5.8493e+05,6.1203e+05,6.3973e+05,6.6804e+05,6.9695e+05,7.2646e+05,7.5658e+05,7.873e+05
      | 0,402.25,1575.9,3502.8,6173.8,9582.1,13723,18592,24187,30503,37540,45293,53762,62945,72839,83443,94756,1.0678e+05,1.195e+05,1.3293e+05,1.4707e+05,1.6191e+05,1.7745e+05,1.9368e+05,2.1062e+05,2.2826e+05,2.466e+05,2.6563e+05,2.8536e+05,3.0578e+05,3.269e+05,3.4872e+05,3.7123e+05,3.9442e+05,4.1832e+05,4.429e+05,4.6817e+05,4.9414e+05,5.2079e+05,5.4814e+05,5.7617e+05,6.0489e+05,6.343e+05,6.6439e+05,6.9517e+05,7.2664e+05,7.588e+05,7.9163e+05,8.2516e+05,8.5937e+05,8.9426e+05
      | 0,454.56,1780.8,3958.4,6976.8,10828,15508,21011,27333,34471,42422,51185,60755,71132,82313,94296,1.0708e+05,1.2066e+05,1.3505e+05,1.5022e+05,1.662e+05,1.8296e+05,2.0052e+05,2.1888e+05,2.3802e+05,2.5795e+05,2.7867e+05,3.0018e+05,3.2248e+05,3.4556e+05,3.6942e+05,3.9407e+05,4.1951e+05,4.4573e+05,4.7273e+05,5.0051e+05,5.2907e+05,5.5841e+05,5.8853e+05,6.1943e+05,6.5111e+05,6.8356e+05,7.168e+05,7.5081e+05,7.8559e+05,8.2115e+05,8.5749e+05,8.946e+05,9.3248e+05,9.7114e+05,1.0106e+06
      | 0,511.09,2002.3,4450.7,7844.3,12175,17436,23623,30732,38757,47698,57549,68310,79977,92548,1.0602e+05,1.204e+05,1.3567e+05,1.5184e+05,1.689e+05,1.8686e+05,2.0572e+05,2.2546e+05,2.4609e+05,2.6762e+05,2.9003e+05,3.1332e+05,3.3751e+05,3.6258e+05,3.8853e+05,4.1536e+05,4.4308e+05,4.7167e+05,5.0115e+05,5.3151e+05,5.6274e+05,5.9486e+05,6.2785e+05,6.6171e+05,6.9646e+05,7.3207e+05,7.6857e+05,8.0593e+05,8.4417e+05,8.8328e+05,9.2326e+05,9.6412e+05,1.0058e+06,1.0484e+06,1.0919e+06,1.1362e+06
      | 0,571.82,2240.2,4979.5,8776.4,13622,19508,26430,34383,43363,53365,64388,76427,89480,1.0355e+05,1.1862e+05,1.347e+05,1.5179e+05,1.6988e+05,1.8897e+05,2.0907e+05,2.3016e+05,2.5225e+05,2.7534e+05,2.9942e+05,3.2449e+05,3.5056e+05,3.7761e+05,4.0566e+05,4.3469e+05,4.6472e+05,4.9573e+05,5.2772e+05,5.607e+05,5.9467e+05,6.2961e+05,6.6554e+05,7.0245e+05,7.4034e+05,7.7921e+05,8.1906e+05,8.5989e+05,9.017e+05,9.4448e+05,9.8824e+05,1.033e+06,1.0787e+06,1.1254e+06,1.173e+06,1.2216e+06,1.2712e+06
      | 0,636.76,2494.6,5545,9773.1,15169,21724,29432,38288,48287,59426,71700,85106,99642,1.153e+05,1.3209e+05,1.5e+05,1.6903e+05,1.8917e+05,2.1044e+05,2.3281e+05,2.563e+05,2.809e+05,3.066e+05,3.3342e+05,3.6134e+05,3.9037e+05,4.205e+05,4.5173e+05,4.8406e+05,5.1749e+05,5.5202e+05,5.8765e+05,6.2438e+05,6.622e+05,7.0111e+05,7.4112e+05,7.8223e+05,8.2442e+05,8.677e+05,9.1208e+05,9.5754e+05,1.0041e+06,1.0517e+06,1.1005e+06,1.1503e+06,1.2012e+06,1.2532e+06,1.3062e+06,1.3604e+06,1.4156e+06
      | 0,705.9,2765.5,6147.1,10834,16816,24083,32628,42446,53531,65879,79486,94348,1.1046e+05,1.2783e+05,1.4643e+05,1.6629e+05,1.8738e+05,2.0972e+05,2.3329e+05,2.5809e+05,2.8413e+05,3.114e+05,3.399e+05,3.6962e+05,4.0058e+05,4.3276e+05,4.6616e+05,5.0078e+05,5.3662e+05,5.7369e+05,6.1197e+05,6.5146e+05,6.9218e+05,7.3411e+05,7.7725e+05,8.216e+05,8.6717e+05,9.1394e+05,9.6193e+05,1.0111e+06,1.0615e+06,1.1131e+06,1.1659e+06,1.22e+06,1.2752e+06,1.3316e+06,1.3892e+06,1.4481e+06,1.5081e+06,1.5693e+06
      | 0,779.25,3052.9,6785.9,11960,18563,26585,36018,46856,59093,72724,87745,1.0415e+05,1.2194e+05,1.4111e+05,1.6165e+05,1.8357e+05,2.0685e+05,2.3151e+05,2.5753e+05,2.8491e+05,3.1365e+05,3.4376e+05,3.7522e+05,4.0803e+05,4.422e+05,4.7772e+05,5.1459e+05,5.5282e+05,5.9238e+05,6.333e+05,6.7556e+05,7.1916e+05,7.641e+05,8.1039e+05,8.5801e+05,9.0697e+05,9.5727e+05,1.0089e+06,1.0619e+06,1.1162e+06,1.1718e+06,1.2288e+06,1.2871e+06,1.3467e+06,1.4077e+06,1.47e+06,1.5336e+06,1.5985e+06,1.6648e+06,1.7324e+06
      | 0,856.81,3356.7,7461.3,13151,20411,29231,39603,51520,64974,79962,96478,1.1452e+05,1.3408e+05,1.5515e+05,1.7774e+05,2.0184e+05,2.2744e+05,2.5455e+05,2.8316e+05,3.1327e+05,3.4487e+05,3.7797e+05,4.1256e+05,4.4864e+05,4.8621e+05,5.2527e+05,5.6581e+05,6.0784e+05,6.5134e+05,6.9633e+05,7.4279e+05,7.9073e+05,8.4015e+05,8.9104e+05,9.4341e+05,9.9724e+05,1.0525e+06,1.1093e+06,1.1676e+06,1.2273e+06,1.2885e+06,1.3511e+06,1.4152e+06,1.4808e+06,1.5478e+06,1.6163e+06,1.6862e+06,1.7576e+06,1.8305e+06,1.9048e+06
      | 0,938.57,3677,8173.3,14405,22358,32020,43382,56436,71175,87593,1.0568e+05,1.2545e+05,1.4687e+05,1.6996e+05,1.947e+05,2.211e+05,2.4915e+05,2.7884e+05,3.1018e+05,3.4316e+05,3.7778e+05,4.1404e+05,4.5193e+05,4.9146e+05,5.3261e+05,5.754e+05,6.1981e+05,6.6584e+05,7.135e+05,7.6278e+05,8.1368e+05,8.6619e+05,9.2032e+05,9.7607e+05,1.0334e+06,1.0924e+06,1.153e+06,1.2152e+06,1.279e+06,1.3444e+06,1.4114e+06,1.48e+06,1.5502e+06,1.6221e+06,1.6955e+06,1.7705e+06,1.8471e+06,1.9254e+06,2.0052e+06,2.0866e+06
      | 0,1024.5,4013.8,8921.9,15725,24406,34953,47356,61605,77694,95616,1.1537e+05,1.3694e+05,1.6032e+05,1.8553e+05,2.1254e+05,2.4135e+05,2.7197e+05,3.0438e+05,3.3859e+05,3.7459e+05,4.1238e+05,4.5196e+05,4.9333e+05,5.3647e+05,5.814e+05,6.281e+05,6.7658e+05,7.2683e+05,7.7885e+05,8.3264e+05,8.8821e+05,9.4553e+05,1.0046e+06,1.0655e+06,1.1281e+06,1.1925e+06,1.2586e+06,1.3265e+06,1.3961e+06,1.4675e+06,1.5407e+06,1.6156e+06,1.6922e+06,1.7706e+06,1.8508e+06,1.9327e+06,2.0163e+06,2.1017e+06,2.1889e+06,2.2777e+06
      | 0,1114.7,4367.1,9707.2,17109,26554,38030,51524,67028,84533,1.0403e+05,1.2552e+05,1.4899e+05,1.7444e+05,2.0185e+05,2.3124e+05,2.6259e+05,2.959e+05,3.3117e+05,3.6839e+05,4.0756e+05,4.4868e+05,4.9174e+05,5.3675e+05,5.8369e+05,6.3257e+05,6.8338e+05,7.3613e+05,7.908e+05,8.474e+05,9.0593e+05,9.6638e+05,1.0288e+06,1.093e+06,1.1593e+06,1.2274e+06,1.2974e+06,1.3694e+06,1.4432e+06,1.519e+06,1.5967e+06,1.6763e+06,1.7578e+06,1.8412e+06,1.9265e+06,2.0137e+06,2.1028e+06,2.1938e+06,2.2867e+06,2.3815e+06,2.4782e+06]
      settings: SourceProductName=Powertrain Blockset  SourceProductBaseCode=PW
  Longitudinal Wheel - Drum Brake : autolibshared/Longitudinal Wheel  FxType=Magic Formula constant value  rollingType=Pressure and velocity  BrakeType=Drum  vertType=None  lam_x=1  extMu=off  aMode=2  br=0.001  Iyy=0.8  omegao=0  Lrel=0.5  Re=0.3  UNLOADED_RADIUS=0.4  LONGVL=16  gamma=0  NOMPRES=220000  press=220000  extPress=off  Dx=1  Cx=1.65  Bx=10  Ex=0.01  PCX1=1.6  PDX1=1  PDX2=-0.08  PDX3=0  PEX1=0.112  PEX2=0.313  PEX3=0  PEX4=0.0016  PKX1=21.7  PKX2=13.77  PKX3=-0.412  PHX1=2.1585E-4  PHX2=0.00115  PVX1=1.5973E-5  PVX2=1.043E-4  PPX1=-0.3489  PPX2=0.382  PPX3=-0.09634  PPX4=0.06447  lam_muV=1  lam_Kxkappa=1  lam_Cx=1  lam_Ex=0  lam_Hx=1  lam_Vx=1  kappaFx=[-1,-0.78476,-0.61585,-0.48329,-0.37927,-0.29764,-0.23357,-0.1833,-0.14384,-0.11288,-0.088587,-0.069519,-0.054556,-0.042813,-0.033598,-0.026367,-0.020691,-0.016238,-0.012743,-0.01,0.01,0.012743,0.016238,0.020691,0.026367,0.033598,0.042813,0.054556,0.069519,0.088587,0.11288,0.14384,0.1833,0.23357,0.29764,0.37927,0.48329,0.61585,0.78476,1]  FzFx=[0,200,400,600,800,1000,1200,1400,1600,1800,2000,2200,2400,2600,2800,3000,3200,3400,3600,3800,4000,4200,4400,4600,4800,5000,5200,5400,5600,5800,6000,6200,6400,6600,6800,7000,7200,7400,7600,7800,8000,8200,8400,8600,8800,9000,9200,9400,9600,9800,10000]  FxMap=|  aMy=84e-4  bMy=6.2e-4  cMy=1.6e-4  alphaMy=-0.003  betaMy=0.97  QSY1=0.007  QSY2=0  QSY3=0.0015  QSY4=8.5e-05  QSY5=0  QSY6=0  QSY7=0.9  QSY8=-0.4  lam_My=1  VxMy=-20:1:20  FzMy=0:200:1e4  MyMap=|  Fpl=10  Cr=1e-3  Kt=.008  Tmeas=25  Tamb=298.15  extTamb=off  mu_static=0.3  mu_kinetic=0.2  disk_abore=0.05  Rm=0.1778  num_pads=2  drum_abore=0.0508  drum_a=0.123  drum_c=0.212  drum_r=0.15  drum_theta1=0  drum_theta2=126  brake_p_bpt=[1 11.4736842105263 21.9473684210526 32.4210526315789 42.8947368421053 53.3684210526316 63.8421052631579 74.3157894736842 84.7894736842105 95.2631578947368 105.736842105263 116.210526315789 126.684210526316 137.157894736842 147.631578947368 158.105263157895 168.578947368421 179.052631578947 189.526315789474 200]  brake_n_bpt=[0 52.6315789473684 105.263157894737 157.894736842105 210.526315789474 263.157894736842 315.789473684211 368.421052631579 421.052631578947 473.684210526316 526.315789473684 578.947368421053 631.578947368421 684.210526315789 736.842105263158 789.473684210526 842.105263157895 894.736842105263 947.368421052632 1000]  f_brake_t=[43.4900602404453 42.5056030554862 41.5350898940194 40.5780454442085 39.6340111501808 38.7025443887544 37.7832176914519 36.8756180088306 35.9793460143796 35.0940154454303 34.2192524787115 33.3546951383474 32.4999927342521 31.6548053290159 30.8188032315107 29.991666515561 29.1730845621415 28.362755623661 27.5603864089927 26.765691687993;498.991217495636 487.695866636631 476.560505099801 465.579679307235 454.748127933653 444.060772460445 433.51270824929 423.099196101319 412.81565427025 402.657650900201 392.620896861006 382.701238955775 372.894653477208 363.197240090814 353.605216024701 344.114910546964 334.722759712992 325.425301366216 316.219170376863 307.10109410434;954.492374750826 932.886130217776 911.585920305583 890.581313170261 869.862244717126 849.419000532136 829.242198807128 809.322774193808 789.651962526121 770.221286354971 751.0225412433 732.047782773203 713.289314220164 694.739674852612 676.391628817892 658.238154578366 640.272434863842 622.48784710877 604.877954344734 587.436496520688;1409.99353200602 1378.07639379892 1346.61133551136 1315.58294703329 1284.9763615006 1254.77722860383 1224.97168936497 1195.5463522863 1166.48827078199 1137.78492180974 1109.42418562559 1081.39432659063 1053.68397496312 1026.28210961441 999.178041611083 972.361398609768 945.822110014692 919.550392851325 893.536738312604 867.771898937035;1865.49468926121 1823.26665738007 1781.63675071715 1740.58458089631 1700.09047828407 1660.13545667552 1620.7011799228 1581.76993037878 1543.32457903786 1505.34855726451 1467.82583000789 1430.74087040806 1394.07863570608 1357.82454437621 1321.96445440427 1286.48464264117 1251.37178516554 1216.61293859388 1182.19552228048 1148.10730135338;2320.9958465164 2268.45692096121 2216.66216592293 2165.58621475934 2115.20459506754 2065.49368474721 2016.43067048064 1967.99350847127 1920.16088729373 1872.91219271928 1826.22747439018 1780.08741422549 1734.47329644903 1689.36697913801 1644.75086719747 1600.60788667257 1556.92146031639 1513.67548433643 1470.85430624835 1428.44270376973;2776.49700377159 2713.64718454235 2651.68758112871 2590.58784862237 2530.31871185102 2470.8519128189 2412.16016103848 2354.21708656376 2296.9971955496 2240.47582817405 2184.62911877248 2129.43395804292 2074.86795719199 2020.9094138998 1967.53727999066 1914.73113070398 1862.47113546724 1810.73803007899 1759.51309021622 1708.77810618608;3231.99816102678 3158.8374481235 3086.71299633449 3015.58948248539 2945.43282863449 2876.21014089059 2807.88965159632 2740.44066465625 2673.83350380547 2608.03946362882 2543.03076315477 2478.78050186034 2415.26261793494 2352.4518486616 2290.32369278385 2228.85437473538 2168.02081061809 2107.80057582154 2048.17187418409 1989.11350860242;3687.49931828197 3604.02771170464 3521.73841154027 3440.59111634842 3360.54694541796 3281.56836896228 3203.61914215416 3126.66424274874 3050.66981206134 2975.60309908359 2901.43240753707 2828.12704567777 2755.6572786779 2683.9942834234 2613.11010557704 2542.97761876678 2473.57048576894 2404.8631215641 2336.83065815196 2269.44891101877;4143.00047553716 4049.21797528579 3956.76382674606 3865.59275021144 3775.66106220143 3686.92659703397 3599.34863271199 3512.88782084123 3427.50612031721 3343.16673453836 3259.83405191936 3177.4735894952 3096.05193942085 3015.5367181852 2935.89651837023 2857.10086279818 2779.12016091979 2701.92566730665 2625.48944211983 2549.78431343512;4598.50163279235 4494.40823886693 4391.78924195184 4290.59438407447 4190.77517898491 4092.28482510566 3995.07812326983 3899.11139893372 3804.34242857308 3710.73036999313 3618.23569630166 3526.82013331263 3436.44660016381 3347.079152947 3258.68293116342 3171.22410682959 3084.66983607064 2998.98821304921 2914.1482260877 2830.11971585147;5054.00279004754 4939.59850244808 4826.81465715762 4715.59601793749 4605.88929576838 4497.64305317735 4390.80761382767 4285.3349770262 4181.17873682896 4078.2940054479 3976.63734068395 3876.16667713006 3776.84126090677 3678.62158770879 3581.46934395661 3485.34735086099 ...(+2764 chars)]  FNOMIN=2000  lam_Fzo=1  m=10  zo=0  zdoto=0  g=9.81  VERTICAL_STIFFNESS=209000.0  VERTICAL_DAMPING=50  Q_RE0=.99  Q_V1=0  Q_V2=0.047  Q_FZ1=0  Q_FZ2=15.4  Q_FCX=0.134  Q_FCY=.11  Q_CAM=0  PFZ1=0.71  Q_FCY2=-0.48  Q_CAM1=85.2  Q_CAM2=257.0  Q_CAM3=0.512  Q_FYS1=-204500.0  Q_FYS2=-60000  Q_FYS3=88211.7  BOTTOM_OFFST=.01  BOTTOM_STIFF=2000000  zFz=[0 .01 .1]  pFz=[10000 1000000]  Fzz=[0 1e3 1e4; 0 1e4 1e5]  zdotFz=[-20 0 20]  Fzzdot=[500 0 -500;250 0 -250]  Gndz=0  extGnd=off  FZMIN=0  FZMAX=10000  PRESMIN=10000  PRESMAX=1000000  kappamax=1.5  VXLOW=1  TMIN=0  TMAX=400  blkID=0
      | [-0,-131.22,-262.44,-393.66,-524.88,-656.1,-787.32,-918.54,-1049.8,-1181,-1312.2,-1443.4,-1574.6,-1705.9,-1837.1,-1968.3,-2099.5,-2230.7,-2362,-2493.2,-2624.4,-2755.6,-2886.8,-3018.1,-3149.3,-3280.5,-3411.7,-3542.9,-3674.2,-3805.4,-3936.6,-4067.8,-4199,-4330.2,-4461.5,-4592.7,-4723.9,-4855.1,-4986.3,-5117.6,-5248.8,-5380,-5511.2,-5642.4,-5773.7,-5904.9,-6036.1,-6167.3,-6298.5,-6429.8,-6561
      | -0,-137.87,-275.75,-413.62,-551.49,-689.36,-827.24,-965.11,-1103,-1240.9,-1378.7,-1516.6,-1654.5,-1792.3,-1930.2,-2068.1,-2206,-2343.8,-2481.7,-2619.6,-2757.5,-2895.3,-3033.2,-3171.1,-3308.9,-3446.8,-3584.7,-3722.6,-3860.4,-3998.3,-4136.2,-4274,-4411.9,-4549.8,-4687.7,-4825.5,-4963.4,-5101.3,-5239.2,-5377,-5514.9,-5652.8,-5790.6,-5928.5,-6066.4,-6204.3,-6342.1,-6480,-6617.9,-6755.8,-6893.6
      | -0,-145.88,-291.75,-437.63,-583.5,-729.38,-875.25,-1021.1,-1167,-1312.9,-1458.8,-1604.6,-1750.5,-1896.4,-2042.3,-2188.1,-2334,-2479.9,-2625.8,-2771.6,-2917.5,-3063.4,-3209.3,-3355.1,-3501,-3646.9,-3792.8,-3938.6,-4084.5,-4230.4,-4376.3,-4522.1,-4668,-4813.9,-4959.8,-5105.6,-5251.5,-5397.4,-5543.3,-5689.1,-5835,-5980.9,-6126.8,-6272.6,-6418.5,-6564.4,-6710.3,-6856.1,-7002,-7147.9,-7293.8
      | -0,-155.26,-310.53,-465.79,-621.05,-776.32,-931.58,-1086.8,-1242.1,-1397.4,-1552.6,-1707.9,-1863.2,-2018.4,-2173.7,-2328.9,-2484.2,-2639.5,-2794.7,-2950,-3105.3,-3260.5,-3415.8,-3571.1,-3726.3,-3881.6,-4036.8,-4192.1,-4347.4,-4502.6,-4657.9,-4813.2,-4968.4,-5123.7,-5278.9,-5434.2,-5589.5,-5744.7,-5900,-6055.3,-6210.5,-6365.8,-6521.1,-6676.3,-6831.6,-6986.8,-7142.1,-7297.4,-7452.6,-7607.9,-7763.2
      | -0,-165.86,-331.71,-497.57,-663.43,-829.28,-995.14,-1161,-1326.9,-1492.7,-1658.6,-1824.4,-1990.3,-2156.1,-2322,-2487.8,-2653.7,-2819.6,-2985.4,-3151.3,-3317.1,-3483,-3648.8,-3814.7,-3980.6,-4146.4,-4312.3,-4478.1,-4644,-4809.8,-4975.7,-5141.5,-5307.4,-5473.3,-5639.1,-5805,-5970.8,-6136.7,-6302.5,-6468.4,-6634.3,-6800.1,-6966,-7131.8,-7297.7,-7463.5,-7629.4,-7795.2,-7961.1,-8127,-8292.8
      | -0,-177.09,-354.19,-531.28,-708.38,-885.47,-1062.6,-1239.7,-1416.8,-1593.8,-1770.9,-1948,-2125.1,-2302.2,-2479.3,-2656.4,-2833.5,-3010.6,-3187.7,-3364.8,-3541.9,-3719,-3896.1,-4073.2,-4250.3,-4427.4,-4604.5,-4781.5,-4958.6,-5135.7,-5312.8,-5489.9,-5667,-5844.1,-6021.2,-6198.3,-6375.4,-6552.5,-6729.6,-6906.7,-7083.8,-7260.9,-7438,-7615.1,-7792.1,-7969.2,-8146.3,-8323.4,-8500.5,-8677.6,-8854.7
      | -0,-187.84,-375.67,-563.51,-751.35,-939.18,-1127,-1314.9,-1502.7,-1690.5,-1878.4,-2066.2,-2254,-2441.9,-2629.7,-2817.5,-3005.4,-3193.2,-3381.1,-3568.9,-3756.7,-3944.6,-4132.4,-4320.2,-4508.1,-4695.9,-4883.7,-5071.6,-5259.4,-5447.3,-5635.1,-5822.9,-6010.8,-6198.6,-6386.4,-6574.3,-6762.1,-6949.9,-7137.8,-7325.6,-7513.5,-7701.3,-7889.1,-8077,-8264.8,-8452.6,-8640.5,-8828.3,-9016.1,-9204,-9391.8
      | -0,-196.25,-392.49,-588.74,-784.98,-981.23,-1177.5,-1373.7,-1570,-1766.2,-1962.5,-2158.7,-2354.9,-2551.2,-2747.4,-2943.7,-3139.9,-3336.2,-3532.4,-3728.7,-3924.9,-4121.2,-4317.4,-4513.6,-4709.9,-4906.1,-5102.4,-5298.6,-5494.9,-5691.1,-5887.4,-6083.6,-6279.9,-6476.1,-6672.3,-6868.6,-7064.8,-7261.1,-7457.3,-7653.6,-7849.8,-8046.1,-8242.3,-8438.6,-8634.8,-8831,-9027.3,-9223.5,-9419.8,-9616,-9812.3
      | -0,-199.97,-399.95,-599.92,-799.9,-999.87,-1199.8,-1399.8,-1599.8,-1799.8,-1999.7,-2199.7,-2399.7,-2599.7,-2799.6,-2999.6,-3199.6,-3399.6,-3599.5,-3799.5,-3999.5,-4199.5,-4399.4,-4599.4,-4799.4,-4999.4,-5199.3,-5399.3,-5599.3,-5799.2,-5999.2,-6199.2,-6399.2,-6599.1,-6799.1,-6999.1,-7199.1,-7399,-7599,-7799,-7999,-8198.9,-8398.9,-8598.9,-8798.9,-8998.8,-9198.8,-9398.8,-9598.8,-9798.7,-9998.7
      | -0,-196.87,-393.74,-590.6,-787.47,-984.34,-1181.2,-1378.1,-1574.9,-1771.8,-1968.7,-2165.5,-2362.4,-2559.3,-2756.2,-2953,-3149.9,-3346.8,-3543.6,-3740.5,-3937.4,-4134.2,-4331.1,-4528,-4724.8,-4921.7,-5118.6,-5315.4,-5512.3,-5709.2,-5906,-6102.9,-6299.8,-6496.6,-6693.5,-6890.4,-7087.2,-7284.1,-7481,-7677.8,-7874.7,-8071.6,-8268.5,-8465.3,-8662.2,-8859.1,-9055.9,-9252.8,-9449.7,-9646.5,-9843.4
      | -0,-186.02,-372.04,-558.06,-744.08,-930.1,-1116.1,-1302.1,-1488.2,-1674.2,-1860.2,-2046.2,-2232.2,-2418.3,-2604.3,-2790.3,-2976.3,-3162.3,-3348.4,-3534.4,-3720.4,-3906.4,-4092.4,-4278.5,-4464.5,-4650.5,-4836.5,-5022.5,-5208.6,-5394.6,-5580.6,-5766.6,-5952.6,-6138.7,-6324.7,-6510.7,-6696.7,-6882.7,-7068.7,-7254.8,-7440.8,-7626.8,-7812.8,-7998.8,-8184.9,-8370.9,-8556.9,-8742.9,-8928.9,-9115,-9301
      | -0,-168.44,-336.89,-505.33,-673.78,-842.22,-1010.7,-1179.1,-1347.6,-1516,-1684.4,-1852.9,-2021.3,-2189.8,-2358.2,-2526.7,-2695.1,-2863.5,-3032,-3200.4,-3368.9,-3537.3,-3705.8,-3874.2,-4042.7,-4211.1,-4379.5,-4548,-4716.4,-4884.9,-5053.3,-5221.8,-5390.2,-5558.6,-5727.1,-5895.5,-6064,-6232.4,-6400.9,-6569.3,-6737.8,-6906.2,-7074.6,-7243.1,-7411.5,-7580,-7748.4,-7916.9,-8085.3,-8253.7,-8422.2
      | -0,-146.7,-293.4,-440.1,-586.81,-733.51,-880.21,-1026.9,-1173.6,-1320.3,-1467,-1613.7,-1760.4,-1907.1,-2053.8,-2200.5,-2347.2,-2493.9,-2640.6,-2787.3,-2934,-3080.7,-3227.4,-3374.1,-3520.8,-3667.5,-3814.2,-3960.9,-4107.6,-4254.3,-4401,-4547.7,-4694.5,-4841.2,-4987.9,-5134.6,-5281.3,-5428,-5574.7,-5721.4,-5868.1,-6014.8,-6161.5,-6308.2,-6454.9,-6601.6,-6748.3,-6895,-7041.7,-7188.4,-7335.1
      | -0,-123.75,-247.49,-371.24,-494.99,-618.73,-742.48,-866.23,-989.98,-1113.7,-1237.5,-1361.2,-1485,-1608.7,-1732.5,-1856.2,-1980,-2103.7,-2227.4,-2351.2,-2474.9,-2598.7,-2722.4,-2846.2,-2969.9,-3093.7,-3217.4,-3341.2,-3464.9,-3588.7,-3712.4,-3836.2,-3959.9,-4083.7,-4207.4,-4331.1,-4454.9,-4578.6,-4702.4,-4826.1,-4949.9,-5073.6,-5197.4,-5321.1,-5444.9,-5568.6,-5692.4,-5816.1,-5939.9,-6063.6,-6187.3
      | -0,-101.91,-203.81,-305.72,-407.63,-509.53,-611.44,-713.35,-815.25,-917.16,-1019.1,-1121,-1222.9,-1324.8,-1426.7,-1528.6,-1630.5,-1732.4,-1834.3,-1936.2,-2038.1,-2140,-2241.9,-2343.9,-2445.8,-2547.7,-2649.6,-2751.5,-2853.4,-2955.3,-3057.2,-3159.1,-3261,-3362.9,-3464.8,-3566.7,-3668.6,-3770.5,-3872.5,-3974.4,-4076.3,-4178.2,-4280.1,-4382,-4483.9,-4585.8,-4687.7,-4789.6,-4891.5,-4993.4,-5095.3
      | -0,-82.514,-165.03,-247.54,-330.06,-412.57,-495.09,-577.6,-660.12,-742.63,-825.14,-907.66,-990.17,-1072.7,-1155.2,-1237.7,-1320.2,-1402.7,-1485.3,-1567.8,-1650.3,-1732.8,-1815.3,-1897.8,-1980.3,-2062.9,-2145.4,-2227.9,-2310.4,-2392.9,-2475.4,-2557.9,-2640.5,-2723,-2805.5,-2888,-2970.5,-3053,-3135.6,-3218.1,-3300.6,-3383.1,-3465.6,-3548.1,-3630.6,-3713.2,-3795.7,-3878.2,-3960.7,-4043.2,-4125.7
      | -0,-66.058,-132.12,-198.17,-264.23,-330.29,-396.35,-462.41,-528.46,-594.52,-660.58,-726.64,-792.7,-858.76,-924.81,-990.87,-1056.9,-1123,-1189,-1255.1,-1321.2,-1387.2,-1453.3,-1519.3,-1585.4,-1651.5,-1717.5,-1783.6,-1849.6,-1915.7,-1981.7,-2047.8,-2113.9,-2179.9,-2246,-2312,-2378.1,-2444.2,-2510.2,-2576.3,-2642.3,-2708.4,-2774.4,-2840.5,-2906.6,-2972.6,-3038.7,-3104.7,-3170.8,-3236.8,-3302.9
      | -0,-52.494,-104.99,-157.48,-209.98,-262.47,-314.97,-367.46,-419.95,-472.45,-524.94,-577.44,-629.93,-682.43,-734.92,-787.41,-839.91,-892.4,-944.9,-997.39,-1049.9,-1102.4,-1154.9,-1207.4,-1259.9,-1312.4,-1364.9,-1417.3,-1469.8,-1522.3,-1574.8,-1627.3,-1679.8,-1732.3,-1784.8,-1837.3,-1889.8,-1942.3,-1994.8,-2047.3,-2099.8,-2152.3,-2204.8,-2257.3,-2309.7,-2362.2,-2414.7,-2467.2,-2519.7,-2572.2,-2624.7
      | -0,-41.519,-83.039,-124.56,-166.08,-207.6,-249.12,-290.64,-332.15,-373.67,-415.19,-456.71,-498.23,-539.75,-581.27,-622.79,-664.31,-705.83,-747.35,-788.87,-830.39,-871.91,-913.42,-954.94,-996.46,-1038,-1079.5,-1121,-1162.5,-1204.1,-1245.6,-1287.1,-1328.6,-1370.1,-1411.7,-1453.2,-1494.7,-1536.2,-1577.7,-1619.3,-1660.8,-1702.3,-1743.8,-1785.3,-1826.8,-1868.4,-1909.9,-1951.4,-1992.9,-2034.4,-2076
      | -0,-32.742,-65.483,-98.225,-130.97,-163.71,-196.45,-229.19,-261.93,-294.67,-327.42,-360.16,-392.9,-425.64,-458.38,-491.12,-523.86,-556.61,-589.35,-622.09,-654.83,-687.57,-720.31,-753.06,-785.8,-818.54,-851.28,-884.02,-916.76,-949.5,-982.25,-1015,-1047.7,-1080.5,-1113.2,-1146,-1178.7,-1211.4,-1244.2,-1276.9,-1309.7,-1342.4,-1375.1,-1407.9,-1440.6,-1473.4,-1506.1,-1538.9,-1571.6,-1604.3,-1637.1
      | 0,32.742,65.483,98.225,130.97,163.71,196.45,229.19,261.93,294.67,327.42,360.16,392.9,425.64,458.38,491.12,523.86,556.61,589.35,622.09,654.83,687.57,720.31,753.06,785.8,818.54,851.28,884.02,916.76,949.5,982.25,1015,1047.7,1080.5,1113.2,1146,1178.7,1211.4,1244.2,1276.9,1309.7,1342.4,1375.1,1407.9,1440.6,1473.4,1506.1,1538.9,1571.6,1604.3,1637.1
      | 0,41.519,83.039,124.56,166.08,207.6,249.12,290.64,332.15,373.67,415.19,456.71,498.23,539.75,581.27,622.79,664.31,705.83,747.35,788.87,830.39,871.91,913.42,954.94,996.46,1038,1079.5,1121,1162.5,1204.1,1245.6,1287.1,1328.6,1370.1,1411.7,1453.2,1494.7,1536.2,1577.7,1619.3,1660.8,1702.3,1743.8,1785.3,1826.8,1868.4,1909.9,1951.4,1992.9,2034.4,2076
      | 0,52.494,104.99,157.48,209.98,262.47,314.97,367.46,419.95,472.45,524.94,577.44,629.93,682.43,734.92,787.41,839.91,892.4,944.9,997.39,1049.9,1102.4,1154.9,1207.4,1259.9,1312.4,1364.9,1417.3,1469.8,1522.3,1574.8,1627.3,1679.8,1732.3,1784.8,1837.3,1889.8,1942.3,1994.8,2047.3,2099.8,2152.3,2204.8,2257.3,2309.7,2362.2,2414.7,2467.2,2519.7,2572.2,2624.7
      | 0,66.058,132.12,198.17,264.23,330.29,396.35,462.41,528.46,594.52,660.58,726.64,792.7,858.76,924.81,990.87,1056.9,1123,1189,1255.1,1321.2,1387.2,1453.3,1519.3,1585.4,1651.5,1717.5,1783.6,1849.6,1915.7,1981.7,2047.8,2113.9,2179.9,2246,2312,2378.1,2444.2,2510.2,2576.3,2642.3,2708.4,2774.4,2840.5,2906.6,2972.6,3038.7,3104.7,3170.8,3236.8,3302.9
      | 0,82.514,165.03,247.54,330.06,412.57,495.09,577.6,660.12,742.63,825.14,907.66,990.17,1072.7,1155.2,1237.7,1320.2,1402.7,1485.3,1567.8,1650.3,1732.8,1815.3,1897.8,1980.3,2062.9,2145.4,2227.9,2310.4,2392.9,2475.4,2557.9,2640.5,2723,2805.5,2888,2970.5,3053,3135.6,3218.1,3300.6,3383.1,3465.6,3548.1,3630.6,3713.2,3795.7,3878.2,3960.7,4043.2,4125.7
      | 0,101.91,203.81,305.72,407.63,509.53,611.44,713.35,815.25,917.16,1019.1,1121,1222.9,1324.8,1426.7,1528.6,1630.5,1732.4,1834.3,1936.2,2038.1,2140,2241.9,2343.9,2445.8,2547.7,2649.6,2751.5,2853.4,2955.3,3057.2,3159.1,3261,3362.9,3464.8,3566.7,3668.6,3770.5,3872.5,3974.4,4076.3,4178.2,4280.1,4382,4483.9,4585.8,4687.7,4789.6,4891.5,4993.4,5095.3
      | 0,123.75,247.49,371.24,494.99,618.73,742.48,866.23,989.98,1113.7,1237.5,1361.2,1485,1608.7,1732.5,1856.2,1980,2103.7,2227.4,2351.2,2474.9,2598.7,2722.4,2846.2,2969.9,3093.7,3217.4,3341.2,3464.9,3588.7,3712.4,3836.2,3959.9,4083.7,4207.4,4331.1,4454.9,4578.6,4702.4,4826.1,4949.9,5073.6,5197.4,5321.1,5444.9,5568.6,5692.4,5816.1,5939.9,6063.6,6187.3
      | 0,146.7,293.4,440.1,586.81,733.51,880.21,1026.9,1173.6,1320.3,1467,1613.7,1760.4,1907.1,2053.8,2200.5,2347.2,2493.9,2640.6,2787.3,2934,3080.7,3227.4,3374.1,3520.8,3667.5,3814.2,3960.9,4107.6,4254.3,4401,4547.7,4694.5,4841.2,4987.9,5134.6,5281.3,5428,5574.7,5721.4,5868.1,6014.8,6161.5,6308.2,6454.9,6601.6,6748.3,6895,7041.7,7188.4,7335.1
      | 0,168.44,336.89,505.33,673.78,842.22,1010.7,1179.1,1347.6,1516,1684.4,1852.9,2021.3,2189.8,2358.2,2526.7,2695.1,2863.5,3032,3200.4,3368.9,3537.3,3705.8,3874.2,4042.7,4211.1,4379.5,4548,4716.4,4884.9,5053.3,5221.8,5390.2,5558.6,5727.1,5895.5,6064,6232.4,6400.9,6569.3,6737.8,6906.2,7074.6,7243.1,7411.5,7580,7748.4,7916.9,8085.3,8253.7,8422.2
      | 0,186.02,372.04,558.06,744.08,930.1,1116.1,1302.1,1488.2,1674.2,1860.2,2046.2,2232.2,2418.3,2604.3,2790.3,2976.3,3162.3,3348.4,3534.4,3720.4,3906.4,4092.4,4278.5,4464.5,4650.5,4836.5,5022.5,5208.6,5394.6,5580.6,5766.6,5952.6,6138.7,6324.7,6510.7,6696.7,6882.7,7068.7,7254.8,7440.8,7626.8,7812.8,7998.8,8184.9,8370.9,8556.9,8742.9,8928.9,9115,9301
      | 0,196.87,393.74,590.6,787.47,984.34,1181.2,1378.1,1574.9,1771.8,1968.7,2165.5,2362.4,2559.3,2756.2,2953,3149.9,3346.8,3543.6,3740.5,3937.4,4134.2,4331.1,4528,4724.8,4921.7,5118.6,5315.4,5512.3,5709.2,5906,6102.9,6299.8,6496.6,6693.5,6890.4,7087.2,7284.1,7481,7677.8,7874.7,8071.6,8268.5,8465.3,8662.2,8859.1,9055.9,9252.8,9449.7,9646.5,9843.4
      | 0,199.97,399.95,599.92,799.9,999.87,1199.8,1399.8,1599.8,1799.8,1999.7,2199.7,2399.7,2599.7,2799.6,2999.6,3199.6,3399.6,3599.5,3799.5,3999.5,4199.5,4399.4,4599.4,4799.4,4999.4,5199.3,5399.3,5599.3,5799.2,5999.2,6199.2,6399.2,6599.1,6799.1,6999.1,7199.1,7399,7599,7799,7999,8198.9,8398.9,8598.9,8798.9,8998.8,9198.8,9398.8,9598.8,9798.7,9998.7
      | 0,196.25,392.49,588.74,784.98,981.23,1177.5,1373.7,1570,1766.2,1962.5,2158.7,2354.9,2551.2,2747.4,2943.7,3139.9,3336.2,3532.4,3728.7,3924.9,4121.2,4317.4,4513.6,4709.9,4906.1,5102.4,5298.6,5494.9,5691.1,5887.4,6083.6,6279.9,6476.1,6672.3,6868.6,7064.8,7261.1,7457.3,7653.6,7849.8,8046.1,8242.3,8438.6,8634.8,8831,9027.3,9223.5,9419.8,9616,9812.3
      | 0,187.84,375.67,563.51,751.35,939.18,1127,1314.9,1502.7,1690.5,1878.4,2066.2,2254,2441.9,2629.7,2817.5,3005.4,3193.2,3381.1,3568.9,3756.7,3944.6,4132.4,4320.2,4508.1,4695.9,4883.7,5071.6,5259.4,5447.3,5635.1,5822.9,6010.8,6198.6,6386.4,6574.3,6762.1,6949.9,7137.8,7325.6,7513.5,7701.3,7889.1,8077,8264.8,8452.6,8640.5,8828.3,9016.1,9204,9391.8
      | 0,177.09,354.19,531.28,708.38,885.47,1062.6,1239.7,1416.8,1593.8,1770.9,1948,2125.1,2302.2,2479.3,2656.4,2833.5,3010.6,3187.7,3364.8,3541.9,3719,3896.1,4073.2,4250.3,4427.4,4604.5,4781.5,4958.6,5135.7,5312.8,5489.9,5667,5844.1,6021.2,6198.3,6375.4,6552.5,6729.6,6906.7,7083.8,7260.9,7438,7615.1,7792.1,7969.2,8146.3,8323.4,8500.5,8677.6,8854.7
      | 0,165.86,331.71,497.57,663.43,829.28,995.14,1161,1326.9,1492.7,1658.6,1824.4,1990.3,2156.1,2322,2487.8,2653.7,2819.6,2985.4,3151.3,3317.1,3483,3648.8,3814.7,3980.6,4146.4,4312.3,4478.1,4644,4809.8,4975.7,5141.5,5307.4,5473.3,5639.1,5805,5970.8,6136.7,6302.5,6468.4,6634.3,6800.1,6966,7131.8,7297.7,7463.5,7629.4,7795.2,7961.1,8127,8292.8
      | 0,155.26,310.53,465.79,621.05,776.32,931.58,1086.8,1242.1,1397.4,1552.6,1707.9,1863.2,2018.4,2173.7,2328.9,2484.2,2639.5,2794.7,2950,3105.3,3260.5,3415.8,3571.1,3726.3,3881.6,4036.8,4192.1,4347.4,4502.6,4657.9,4813.2,4968.4,5123.7,5278.9,5434.2,5589.5,5744.7,5900,6055.3,6210.5,6365.8,6521.1,6676.3,6831.6,6986.8,7142.1,7297.4,7452.6,7607.9,7763.2
      | 0,145.88,291.75,437.63,583.5,729.38,875.25,1021.1,1167,1312.9,1458.8,1604.6,1750.5,1896.4,2042.3,2188.1,2334,2479.9,2625.8,2771.6,2917.5,3063.4,3209.3,3355.1,3501,3646.9,3792.8,3938.6,4084.5,4230.4,4376.3,4522.1,4668,4813.9,4959.8,5105.6,5251.5,5397.4,5543.3,5689.1,5835,5980.9,6126.8,6272.6,6418.5,6564.4,6710.3,6856.1,7002,7147.9,7293.8
      | 0,137.87,275.75,413.62,551.49,689.36,827.24,965.11,1103,1240.9,1378.7,1516.6,1654.5,1792.3,1930.2,2068.1,2206,2343.8,2481.7,2619.6,2757.5,2895.3,3033.2,3171.1,3308.9,3446.8,3584.7,3722.6,3860.4,3998.3,4136.2,4274,4411.9,4549.8,4687.7,4825.5,4963.4,5101.3,5239.2,5377,5514.9,5652.8,5790.6,5928.5,6066.4,6204.3,6342.1,6480,6617.9,6755.8,6893.6
      | 0,131.22,262.44,393.66,524.88,656.1,787.32,918.54,1049.8,1181,1312.2,1443.4,1574.6,1705.9,1837.1,1968.3,2099.5,2230.7,2362,2493.2,2624.4,2755.6,2886.8,3018.1,3149.3,3280.5,3411.7,3542.9,3674.2,3805.4,3936.6,4067.8,4199,4330.2,4461.5,4592.7,4723.9,4855.1,4986.3,5117.6,5248.8,5380,5511.2,5642.4,5773.7,5904.9,6036.1,6167.3,6298.5,6429.8,6561]
      | [0,1114.7,4367.1,9707.2,17109,26554,38030,51524,67028,84533,1.0403e+05,1.2552e+05,1.4899e+05,1.7444e+05,2.0185e+05,2.3124e+05,2.6259e+05,2.959e+05,3.3117e+05,3.6839e+05,4.0756e+05,4.4868e+05,4.9174e+05,5.3675e+05,5.8369e+05,6.3257e+05,6.8338e+05,7.3613e+05,7.908e+05,8.474e+05,9.0593e+05,9.6638e+05,1.0288e+06,1.093e+06,1.1593e+06,1.2274e+06,1.2974e+06,1.3694e+06,1.4432e+06,1.519e+06,1.5967e+06,1.6763e+06,1.7578e+06,1.8412e+06,1.9265e+06,2.0137e+06,2.1028e+06,2.1938e+06,2.2867e+06,2.3815e+06,2.4782e+06
      | 0,1024.5,4013.8,8921.9,15725,24406,34953,47356,61605,77694,95616,1.1537e+05,1.3694e+05,1.6032e+05,1.8553e+05,2.1254e+05,2.4135e+05,2.7197e+05,3.0438e+05,3.3859e+05,3.7459e+05,4.1238e+05,4.5196e+05,4.9333e+05,5.3647e+05,5.814e+05,6.281e+05,6.7658e+05,7.2683e+05,7.7885e+05,8.3264e+05,8.8821e+05,9.4553e+05,1.0046e+06,1.0655e+06,1.1281e+06,1.1925e+06,1.2586e+06,1.3265e+06,1.3961e+06,1.4675e+06,1.5407e+06,1.6156e+06,1.6922e+06,1.7706e+06,1.8508e+06,1.9327e+06,2.0163e+06,2.1017e+06,2.1889e+06,2.2777e+06
      | 0,938.57,3677,8173.3,14405,22358,32020,43382,56436,71175,87593,1.0568e+05,1.2545e+05,1.4687e+05,1.6996e+05,1.947e+05,2.211e+05,2.4915e+05,2.7884e+05,3.1018e+05,3.4316e+05,3.7778e+05,4.1404e+05,4.5193e+05,4.9146e+05,5.3261e+05,5.754e+05,6.1981e+05,6.6584e+05,7.135e+05,7.6278e+05,8.1368e+05,8.6619e+05,9.2032e+05,9.7607e+05,1.0334e+06,1.0924e+06,1.153e+06,1.2152e+06,1.279e+06,1.3444e+06,1.4114e+06,1.48e+06,1.5502e+06,1.6221e+06,1.6955e+06,1.7705e+06,1.8471e+06,1.9254e+06,2.0052e+06,2.0866e+06
      | 0,856.81,3356.7,7461.3,13151,20411,29231,39603,51520,64974,79962,96478,1.1452e+05,1.3408e+05,1.5515e+05,1.7774e+05,2.0184e+05,2.2744e+05,2.5455e+05,2.8316e+05,3.1327e+05,3.4487e+05,3.7797e+05,4.1256e+05,4.4864e+05,4.8621e+05,5.2527e+05,5.6581e+05,6.0784e+05,6.5134e+05,6.9633e+05,7.4279e+05,7.9073e+05,8.4015e+05,8.9104e+05,9.4341e+05,9.9724e+05,1.0525e+06,1.1093e+06,1.1676e+06,1.2273e+06,1.2885e+06,1.3511e+06,1.4152e+06,1.4808e+06,1.5478e+06,1.6163e+06,1.6862e+06,1.7576e+06,1.8305e+06,1.9048e+06
      | 0,779.25,3052.9,6785.9,11960,18563,26585,36018,46856,59093,72724,87745,1.0415e+05,1.2194e+05,1.4111e+05,1.6165e+05,1.8357e+05,2.0685e+05,2.3151e+05,2.5753e+05,2.8491e+05,3.1365e+05,3.4376e+05,3.7522e+05,4.0803e+05,4.422e+05,4.7772e+05,5.1459e+05,5.5282e+05,5.9238e+05,6.333e+05,6.7556e+05,7.1916e+05,7.641e+05,8.1039e+05,8.5801e+05,9.0697e+05,9.5727e+05,1.0089e+06,1.0619e+06,1.1162e+06,1.1718e+06,1.2288e+06,1.2871e+06,1.3467e+06,1.4077e+06,1.47e+06,1.5336e+06,1.5985e+06,1.6648e+06,1.7324e+06
      | 0,705.9,2765.5,6147.1,10834,16816,24083,32628,42446,53531,65879,79486,94348,1.1046e+05,1.2783e+05,1.4643e+05,1.6629e+05,1.8738e+05,2.0972e+05,2.3329e+05,2.5809e+05,2.8413e+05,3.114e+05,3.399e+05,3.6962e+05,4.0058e+05,4.3276e+05,4.6616e+05,5.0078e+05,5.3662e+05,5.7369e+05,6.1197e+05,6.5146e+05,6.9218e+05,7.3411e+05,7.7725e+05,8.216e+05,8.6717e+05,9.1394e+05,9.6193e+05,1.0111e+06,1.0615e+06,1.1131e+06,1.1659e+06,1.22e+06,1.2752e+06,1.3316e+06,1.3892e+06,1.4481e+06,1.5081e+06,1.5693e+06
      | 0,636.76,2494.6,5545,9773.1,15169,21724,29432,38288,48287,59426,71700,85106,99642,1.153e+05,1.3209e+05,1.5e+05,1.6903e+05,1.8917e+05,2.1044e+05,2.3281e+05,2.563e+05,2.809e+05,3.066e+05,3.3342e+05,3.6134e+05,3.9037e+05,4.205e+05,4.5173e+05,4.8406e+05,5.1749e+05,5.5202e+05,5.8765e+05,6.2438e+05,6.622e+05,7.0111e+05,7.4112e+05,7.8223e+05,8.2442e+05,8.677e+05,9.1208e+05,9.5754e+05,1.0041e+06,1.0517e+06,1.1005e+06,1.1503e+06,1.2012e+06,1.2532e+06,1.3062e+06,1.3604e+06,1.4156e+06
      | 0,571.82,2240.2,4979.5,8776.4,13622,19508,26430,34383,43363,53365,64388,76427,89480,1.0355e+05,1.1862e+05,1.347e+05,1.5179e+05,1.6988e+05,1.8897e+05,2.0907e+05,2.3016e+05,2.5225e+05,2.7534e+05,2.9942e+05,3.2449e+05,3.5056e+05,3.7761e+05,4.0566e+05,4.3469e+05,4.6472e+05,4.9573e+05,5.2772e+05,5.607e+05,5.9467e+05,6.2961e+05,6.6554e+05,7.0245e+05,7.4034e+05,7.7921e+05,8.1906e+05,8.5989e+05,9.017e+05,9.4448e+05,9.8824e+05,1.033e+06,1.0787e+06,1.1254e+06,1.173e+06,1.2216e+06,1.2712e+06
      | 0,511.09,2002.3,4450.7,7844.3,12175,17436,23623,30732,38757,47698,57549,68310,79977,92548,1.0602e+05,1.204e+05,1.3567e+05,1.5184e+05,1.689e+05,1.8686e+05,2.0572e+05,2.2546e+05,2.4609e+05,2.6762e+05,2.9003e+05,3.1332e+05,3.3751e+05,3.6258e+05,3.8853e+05,4.1536e+05,4.4308e+05,4.7167e+05,5.0115e+05,5.3151e+05,5.6274e+05,5.9486e+05,6.2785e+05,6.6171e+05,6.9646e+05,7.3207e+05,7.6857e+05,8.0593e+05,8.4417e+05,8.8328e+05,9.2326e+05,9.6412e+05,1.0058e+06,1.0484e+06,1.0919e+06,1.1362e+06
      | 0,454.56,1780.8,3958.4,6976.8,10828,15508,21011,27333,34471,42422,51185,60755,71132,82313,94296,1.0708e+05,1.2066e+05,1.3505e+05,1.5022e+05,1.662e+05,1.8296e+05,2.0052e+05,2.1888e+05,2.3802e+05,2.5795e+05,2.7867e+05,3.0018e+05,3.2248e+05,3.4556e+05,3.6942e+05,3.9407e+05,4.1951e+05,4.4573e+05,4.7273e+05,5.0051e+05,5.2907e+05,5.5841e+05,5.8853e+05,6.1943e+05,6.5111e+05,6.8356e+05,7.168e+05,7.5081e+05,7.8559e+05,8.2115e+05,8.5749e+05,8.946e+05,9.3248e+05,9.7114e+05,1.0106e+06
      | 0,402.25,1575.9,3502.8,6173.8,9582.1,13723,18592,24187,30503,37540,45293,53762,62945,72839,83443,94756,1.0678e+05,1.195e+05,1.3293e+05,1.4707e+05,1.6191e+05,1.7745e+05,1.9368e+05,2.1062e+05,2.2826e+05,2.466e+05,2.6563e+05,2.8536e+05,3.0578e+05,3.269e+05,3.4872e+05,3.7123e+05,3.9442e+05,4.1832e+05,4.429e+05,4.6817e+05,4.9414e+05,5.2079e+05,5.4814e+05,5.7617e+05,6.0489e+05,6.343e+05,6.6439e+05,6.9517e+05,7.2664e+05,7.588e+05,7.9163e+05,8.2516e+05,8.5937e+05,8.9426e+05
      | 0,354.13,1387.4,3083.9,5435.3,8436,12082,16369,21294,26855,33050,39876,47332,55416,64127,73463,83423,94005,1.0521e+05,1.1703e+05,1.2948e+05,1.4254e+05,1.5622e+05,1.7052e+05,1.8543e+05,2.0096e+05,2.171e+05,2.3386e+05,2.5123e+05,2.6921e+05,2.878e+05,3.0701e+05,3.2682e+05,3.4725e+05,3.6828e+05,3.8993e+05,4.1218e+05,4.3504e+05,4.585e+05,4.8258e+05,5.0725e+05,5.3254e+05,5.5843e+05,5.8493e+05,6.1203e+05,6.3973e+05,6.6804e+05,6.9695e+05,7.2646e+05,7.5658e+05,7.873e+05
      | 0,310.23,1215.4,2701.5,4761.5,7390.2,10584,14339,18654,23526,28952,34932,41464,48546,56176,64355,73080,82351,92166,1.0252e+05,1.1343e+05,1.2487e+05,1.3685e+05,1.4938e+05,1.6244e+05,1.7605e+05,1.9019e+05,2.0487e+05,2.2008e+05,2.3583e+05,2.5212e+05,2.6895e+05,2.863e+05,3.042e+05,3.2262e+05,3.4158e+05,3.6108e+05,3.811e+05,4.0166e+05,4.2275e+05,4.4437e+05,4.6652e+05,4.892e+05,5.1241e+05,5.3615e+05,5.6042e+05,5.8521e+05,6.1054e+05,6.364e+05,6.6278e+05,6.8969e+05
      | 0,270.53,1059.9,2355.8,4152.2,6444.5,9229.4,12504,16267,20515,25247,30462,36158,42334,48988,56120,63728,71813,80372,89405,98911,1.0889e+05,1.1934e+05,1.3026e+05,1.4166e+05,1.5352e+05,1.6585e+05,1.7865e+05,1.9192e+05,2.0566e+05,2.1986e+05,2.3453e+05,2.4967e+05,2.6527e+05,2.8134e+05,2.9787e+05,3.1487e+05,3.3233e+05,3.5026e+05,3.6865e+05,3.875e+05,4.0682e+05,4.266e+05,4.4684e+05,4.6754e+05,4.887e+05,5.1033e+05,5.3241e+05,5.5496e+05,5.7797e+05,6.0143e+05
      | 0,235.04,920.8,2046.8,3607.4,5599,8018.6,10864,14133,17824,21935,26466,31414,36780,42561,48757,55367,62391,69827,77675,85934,94604,1.0368e+05,1.1317e+05,1.2307e+05,1.3338e+05,1.4409e+05,1.5521e+05,1.6674e+05,1.7867e+05,1.9101e+05,2.0376e+05,2.1691e+05,2.3047e+05,2.4443e+05,2.5879e+05,2.7356e+05,2.8873e+05,3.0431e+05,3.2028e+05,3.3666e+05,3.5345e+05,3.7063e+05,3.8821e+05,4.062e+05,4.2459e+05,4.4337e+05,4.6256e+05,4.8215e+05,5.0214e+05,5.2253e+05
      | 0,203.75,798.24,1774.3,3127.2,4853.7,6951.2,9417.7,12252,15451,19015,22943,27233,31884,36896,42267,47997,54086,60533,67336,74496,82011,89882,98108,1.0669e+05,1.1562e+05,1.2491e+05,1.3455e+05,1.4455e+05,1.5489e+05,1.6559e+05,1.7664e+05,1.8804e+05,1.9979e+05,2.1189e+05,2.2434e+05,2.3715e+05,2.503e+05,2.638e+05,2.7765e+05,2.9185e+05,3.064e+05,3.2129e+05,3.3654e+05,3.5213e+05,3.6807e+05,3.8436e+05,4.0099e+05,4.1797e+05,4.353e+05,4.5297e+05
      | 0,176.67,692.15,1538.5,2711.6,4208.6,6027.4,8166.1,10623,13398,16488,19894,23613,27646,31992,36650,41618,46898,52488,58387,64595,71112,77937,85069,92509,1.0026e+05,1.0831e+05,1.1667e+05,1.2533e+05,1.3431e+05,1.4358e+05,1.5316e+05,1.6305e+05,1.7324e+05,1.8373e+05,1.9453e+05,2.0563e+05,2.1703e+05,2.2874e+05,2.4075e+05,2.5306e+05,2.6568e+05,2.7859e+05,2.9181e+05,3.0533e+05,3.1915e+05,3.3327e+05,3.477e+05,3.6242e+05,3.7745e+05,3.9277e+05
      | 0,153.8,602.54,1339.3,2360.6,3663.8,5247,7108.9,9247.9,11663,14353,17318,20556,24067,27850,31905,36230,40826,45692,50828,56232,61905,67847,74056,80533,87277,94287,1.0156e+05,1.0911e+05,1.1692e+05,1.2499e+05,1.3333e+05,1.4194e+05,1.5081e+05,1.5994e+05,1.6934e+05,1.7901e+05,1.8894e+05,1.9913e+05,2.0958e+05,2.203e+05,2.3128e+05,2.4253e+05,2.5403e+05,2.658e+05,2.7783e+05,2.9013e+05,3.0268e+05,3.155e+05,3.2858e+05,3.4192e+05
      | 0,135.13,529.41,1176.8,2074.1,3219.1,4610.2,6246.1,8125.5,10248,12611,15216,18061,21146,24470,28033,31833,35871,40147,44659,49407,54392,59612,65068,70759,76684,82844,89238,95866,1.0273e+05,1.0982e+05,1.1715e+05,1.2471e+05,1.3251e+05,1.4053e+05,1.4879e+05,1.5728e+05,1.66e+05,1.7496e+05,1.8415e+05,1.9356e+05,2.0321e+05,2.1309e+05,2.232e+05,2.3354e+05,2.4411e+05,2.5492e+05,2.6595e+05,2.7721e+05,2.887e+05,3.0042e+05
